simulink model "kinovaMicoSimscapeModel"  (R2021b)
(part 21 of 50)

Y2_4_1=(5991417*ddqr2)/50000000 - (1786417*ddqr3)/50000000 - (203*ddqr1*cos(q2))/100000 - (3393*ddqr2*cos(q3))/31250 + (3393*ddqr3*cos(q3))/62500 - (4329*ddqr4*cos(q4))/625000 - (1369*ddqr2*cos(2*q4))/2000000 + (1369*ddqr3*cos(2*q4))/2000000 + (3393*dq2*dqr3*sin(q3))/62500 + (3393*dq3*dqr2*sin(q3))/62500 - (3393*dq3*dqr3*sin(q3))/62500 + (4329*dq4*dqr4*sin(q4))/625000 - (841*dq1*dqr1*sin(2*q2))/20000 + (1369*dq2*dqr4*sin(2*q4))/2000000 + (1369*dq4*dqr2*sin(2*q4))/2000000 - (1369*dq3*dqr4*sin(2*q4))/2000000 - (1369*dq4*dqr3*sin(2*q4))/2000000 + (819*ddqr1*cos(q2)*cos(q3))/625000 + (1073*ddqr1*cos(q2)*cos(q4))/100000 + (1073*ddqr4*cos(q3)*cos(q4))/100000 + (819*ddqr1*sin(q2)*sin(q3))/625000 + (1073*ddqr2*sin(q3)*sin(q4))/50000 - (1073*ddqr3*sin(q3)*sin(q4))/100000 - (3393*dq1*dqr1*cos(2*q2)*sin(q3))/62500 + (3393*dq1*dqr1*sin(2*q2)*cos(q3))/62500 - (4329*ddqr1*cos(q2)*cos(q3)*cos(q4))/625000 - (259*ddqr1*cos(q2)*sin(q3)*sin(q4))/1000000 + (259*ddqr1*cos(q3)*sin(q2)*sin(q4))/1000000 - (4329*ddqr1*cos(q4)*sin(q2)*sin(q3))/625000 + (1717967*dq1*dqr1*cos(2*q2)*sin(2*q3))/100000000 - (1717967*dq1*dqr1*cos(2*q3)*sin(2*q2))/100000000 + (1369*ddqr1*sin(2*q4)*cos(q2)*sin(q3))/2000000 - (1369*ddqr1*sin(2*q4)*cos(q3)*sin(q2))/2000000 - (1369*dq1*dqr4*cos(q2)*sin(q3))/2000000 + (1369*dq1*dqr4*cos(q3)*sin(q2))/2000000 - (1369*dq4*dqr1*cos(q2)*sin(q3))/2000000 + (1369*dq4*dqr1*cos(q3)*sin(q2))/2000000 - (1073*dq1*dqr4*cos(q2)*sin(q4))/100000 - (1073*dq4*dqr1*cos(q2)*sin(q4))/100000 + (1073*dq2*dqr3*cos(q3)*sin(q4))/100000 + (1073*dq3*dqr2*cos(q3)*sin(q4))/100000 + (1073*dq2*dqr4*cos(q4)*sin(q3))/100000 - (1073*dq3*dqr3*cos(q3)*sin(q4))/100000 + (1073*dq4*dqr2*cos(q4)*sin(q3))/100000 - (1073*dq3*dqr4*cos(q4)*sin(q3))/100000 - (1073*dq4*dqr3*cos(q4)*sin(q3))/100000 - (1073*dq4*dqr4*cos(q3)*sin(q4))/100000 - (1073*dq1*dqr1*cos(2*q2)*cos(q3)*sin(q4))/100000 + (1369*dq1*dqr4*cos(2*q4)*cos(q2)*sin(q3))/2000000 - (1369*dq1*dqr4*cos(2*q4)*cos(q3)*sin(q2))/2000000 + (1369*dq4*dqr1*cos(2*q4)*cos(q2)*sin(q3))/2000000 - (1369*dq4*dqr1*cos(2*q4)*cos(q3)*sin(q2))/2000000 - (1073*dq1*dqr1*sin(2*q2)*sin(q3)*sin(q4))/100000 + (4329*dq1*dqr1*cos(2*q2)*cos(2*q3)*sin(q4))/625000 + (4329*dq1*dqr1*sin(2*q2)*sin(2*q3)*sin(q4))/625000 + (4329*dq1*dqr4*cos(q2)*cos(q3)*sin(q4))/625000 + (4329*dq4*dqr1*cos(q2)*cos(q3)*sin(q4))/625000 + (1369*dq1*dqr1*cos(2*q2)*cos(2*q4)*sin(2*q3))/4000000 - (1369*dq1*dqr1*cos(2*q3)*cos(2*q4)*sin(2*q2))/4000000 + (4329*dq1*dqr4*sin(q2)*sin(q3)*sin(q4))/625000 + (4329*dq4*dqr1*sin(q2)*sin(q3)*sin(q4))/625000;
Y2_5_1=(25433*dq3*dqr2*sin(q3))/400000 - (841*dq1*dqr1*sin(2*q2))/20000 - (25433*dq1*dqr1*cos(2*q2)*sin(q3))/400000 + (25433*dq1*dqr1*sin(2*q2)*cos(q3))/400000 - (1369*dq5*dqr1*cos(q2)*sin(q3))/4000000 + (1369*dq5*dqr1*cos(q3)*sin(q2))/4000000 + (4107*dq4*dqr1*cos(2*q5)*cos(q2)*sin(q3))/16000000 - (4107*dq4*dqr1*cos(2*q5)*cos(q3)*sin(q2))/16000000 - dq1*dqr1*cos(2*q2)*sin(2*q3)*((23717*3^(1/2))/40000000 - 36744657/1600000000) + dq1*dqr1*cos(2*q3)*sin(2*q2)*((23717*3^(1/2))/40000000 - 36744657/1600000000) - dq4*dqr1*cos(q2)*sin(q3)*((23717*3^(1/2))/20000000 + 2122493/800000000) + dq4*dqr1*cos(q3)*sin(q2)*((23717*3^(1/2))/20000000 + 2122493/800000000) + (1073*3^(1/2)*dq3*dqr2*cos(q5)*sin(q3))/200000 + (1073*dq4*dqr1*cos(q2)*cos(q4)*sin(q5))/100000 + (1073*dq4*dqr1*cos(q2)*cos(q5)*sin(q4))/200000 - (1073*dq3*dqr2*cos(q3)*cos(q4)*sin(q5))/100000 - (1073*dq3*dqr2*cos(q3)*cos(q5)*sin(q4))/200000 + (1073*dq5*dqr1*cos(q2)*cos(q4)*sin(q5))/200000 + (1073*dq5*dqr1*cos(q2)*cos(q5)*sin(q4))/100000 - (1073*dq4*dqr2*cos(q4)*cos(q5)*sin(q3))/200000 - (1073*dq5*dqr2*cos(q4)*cos(q5)*sin(q3))/100000 + (12321*dq1*dqr1*cos(2*q2)*cos(2*q5)*sin(2*q3))/32000000 - (12321*dq1*dqr1*cos(2*q3)*cos(2*q5)*sin(2*q2))/32000000 + (1073*dq4*dqr2*sin(q3)*sin(q4)*sin(q5))/100000 + (1073*dq5*dqr2*sin(q3)*sin(q4)*sin(q5))/200000 - dq4*dqr1*cos(q2)*sin(q4)*((18589*3^(1/2))/2000000 + 1073/100000) + dq3*dqr2*cos(q3)*sin(q4)*((18589*3^(1/2))/2000000 + 1073/100000) + dq4*dqr2*cos(q4)*sin(q3)*((18589*3^(1/2))/2000000 + 1073/100000) + (1369*dq1*dqr1*cos(2*q2)*cos(2*q4)*cos(2*q5)*sin(2*q3))/6400000 - (1369*dq1*dqr1*cos(2*q3)*cos(2*q4)*cos(2*q5)*sin(2*q2))/6400000 + (1073*dq1*dqr1*sin(2*q2)*cos(q4)*sin(q3)*sin(q5))/100000 + (1073*dq1*dqr1*sin(2*q2)*cos(q5)*sin(q3)*sin(q4))/200000 - (1369*3^(1/2)*dq5*dqr1*cos(q2)*cos(q3)*sin(q4))/4000000 - (1369*dq1*dqr1*cos(2*q2)*sin(2*q3)*sin(2*q4)*sin(2*q5))/8000000 + (1369*dq1*dqr1*cos(2*q3)*sin(2*q2)*sin(2*q4)*sin(2*q5))/8000000 - dq1*dqr1*cos(2*q2)*cos(q3)*sin(q4)*((18589*3^(1/2))/2000000 + 1073/100000) - (1369*3^(1/2)*dq5*dqr1*sin(q2)*sin(q3)*sin(q4))/4000000 - (32449*dq1*dqr1*cos(2*q2)*cos(2*q3)*cos(q4)*sin(q5))/4000000 + (1369*dq4*dqr1*cos(2*q4)*cos(2*q5)*cos(q2)*sin(q3))/3200000 - (1369*dq4*dqr1*cos(2*q4)*cos(2*q5)*cos(q3)*sin(q2))/3200000 + (1369*dq5*dqr1*cos(2*q4)*cos(2*q5)*cos(q2)*sin(q3))/4000000 - (1369*dq5*dqr1*cos(2*q4)*cos(2*q5)*cos(q3)*sin(q2))/4000000 - dq1*dqr1*sin(2*q2)*sin(q3)*sin(q4)*((18589*3^(1/2))/2000000 + 1073/100000) + dq1*dqr1*cos(2*q2)*cos(2*q4)*sin(2*q3)*((23717*3^(1/2))/40000000 + 1574893/1600000000) - dq1*dqr1*cos(2*q3)*cos(2*q4)*sin(2*q2)*((23717*3^(1/2))/40000000 + 1574893/1600000000) + dq4*dqr1*cos(2*q4)*cos(q2)*sin(q3)*((23717*3^(1/2))/20000000 + 1574893/800000000) - dq4*dqr1*cos(2*q4)*cos(q3)*sin(q2)*((23717*3^(1/2))/20000000 + 1574893/800000000) - (32449*dq1*dqr1*sin(2*q2)*sin(2*q3)*cos(q4)*sin(q5))/4000000 - (1369*dq4*dqr1*sin(2*q4)*sin(2*q5)*cos(q2)*sin(q3))/4000000 + (1369*dq4*dqr1*sin(2*q4)*sin(2*q5)*cos(q3)*sin(q2))/4000000 - (1369*dq5*dqr1*sin(2*q4)*sin(2*q5)*cos(q2)*sin(q3))/3200000 + (1369*dq5*dqr1*sin(2*q4)*sin(2*q5)*cos(q3)*sin(q2))/3200000 - (1073*3^(1/2)*dq1*dqr1*cos(2*q2)*cos(q5)*sin(q3))/200000 + (1073*3^(1/2)*dq1*dqr1*sin(2*q2)*cos(q3)*cos(q5))/200000 - (32449*dq4*dqr1*cos(q2)*cos(q3)*cos(q4)*sin(q5))/4000000 - (32449*dq5*dqr1*cos(q2)*cos(q3)*cos(q4)*sin(q5))/8000000 - (32449*dq5*dqr1*cos(q2)*cos(q3)*cos(q5)*sin(q4))/4000000 + dq1*dqr1*cos(2*q2)*sin(2*q3)*cos(q5)*((348207*3^(1/2))/80000000 + 1369/4000000) - dq1*dqr1*cos(2*q3)*sin(2*q2)*cos(q5)*((348207*3^(1/2))/80000000 + 1369/4000000) + dq1*dqr1*cos(2*q2)*cos(2*q3)*sin(q4)*((548467*3^(1/2))/80000000 + 32449/4000000) - (32449*dq4*dqr1*cos(q4)*sin(q2)*sin(q3)*sin(q5))/4000000 - (32449*dq5*dqr1*cos(q4)*sin(q2)*sin(q3)*sin(q5))/8000000 - (32449*dq5*dqr1*cos(q5)*sin(q2)*sin(q3)*sin(q4))/4000000 + dq1*dqr1*sin(2*q2)*sin(2*q3)*sin(q4)*((548467*3^(1/2))/80000000 + 32449/4000000) + dq4*dqr1*cos(q2)*cos(q5)*sin(q3)*((23717*3^(1/2))/40000000 + 1369/2000000) - dq4*dqr1*cos(q3)*cos(q5)*sin(q2)*((23717*3^(1/2))/40000000 + 1369/2000000) + dq5*dqr1*cos(q2)*cos(q5)*sin(q3)*((23717*3^(1/2))/40000000 + 1369/2000000) - dq5*dqr1*cos(q3)*cos(q5)*sin(q2)*((23717*3^(1/2))/40000000 + 1369/2000000) + dq4*dqr1*cos(q2)*cos(q3)*sin(q4)*((548467*3^(1/2))/80000000 + 32449/4000000) + (1073*dq1*dqr1*cos(2*q2)*cos(q3)*cos(q4)*sin(q5))/100000 + (1073*dq1*dqr1*cos(2*q2)*cos(q3)*cos(q5)*sin(q4))/200000 + dq4*dqr1*sin(q2)*sin(q3)*sin(q4)*((548467*3^(1/2))/80000000 + 32449/4000000) - (1369*3^(1/2)*dq1*dqr1*cos(2*q2)*cos(2*q3)*cos(2*q5)*sin(q4))/8000000 - (1369*3^(1/2)*dq1*dqr1*cos(2*q2)*cos(2*q3)*sin(2*q5)*cos(q4))/4000000 - dq4*dqr1*cos(2*q4)*cos(q2)*cos(q5)*sin(q3)*((23717*3^(1/2))/40000000 + 1369/2000000) + dq4*dqr1*cos(2*q4)*cos(q3)*cos(q5)*sin(q2)*((23717*3^(1/2))/40000000 + 1369/2000000) - dq5*dqr1*cos(2*q4)*cos(q2)*cos(q5)*sin(q3)*((23717*3^(1/2))/40000000 + 1369/2000000) + dq5*dqr1*cos(2*q4)*cos(q3)*cos(q5)*sin(q2)*((23717*3^(1/2))/40000000 + 1369/2000000) - (1369*3^(1/2)*dq1*dqr1*cos(2*q5)*sin(2*q2)*sin(2*q3)*sin(q4))/8000000 - (1369*3^(1/2)*dq1*dqr1*sin(2*q2)*sin(2*q3)*sin(2*q5)*cos(q4))/4000000 + dq4*dqr1*sin(2*q4)*cos(q2)*sin(q3)*sin(q5)*((23717*3^(1/2))/20000000 + 1369/1000000) - dq4*dqr1*sin(2*q4)*cos(q3)*sin(q2)*sin(q5)*((23717*3^(1/2))/20000000 + 1369/1000000) + dq5*dqr1*sin(2*q4)*cos(q2)*sin(q3)*sin(q5)*((23717*3^(1/2))/80000000 + 1369/4000000) - dq5*dqr1*sin(2*q4)*cos(q3)*sin(q2)*sin(q5)*((23717*3^(1/2))/80000000 + 1369/4000000) - (1369*3^(1/2)*dq4*dqr1*cos(2*q5)*cos(q2)*cos(q3)*sin(q4))/8000000 - (1369*3^(1/2)*dq4*dqr1*sin(2*q5)*cos(q2)*cos(q3)*cos(q4))/4000000 - (1369*3^(1/2)*dq5*dqr1*cos(2*q5)*cos(q2)*cos(q3)*sin(q4))/4000000 - (1369*3^(1/2)*dq5*dqr1*sin(2*q5)*cos(q2)*cos(q3)*cos(q4))/8000000 + dq1*dqr1*cos(2*q2)*cos(2*q3)*cos(q5)*sin(q4)*((1369*3^(1/2))/2000000 - 45547/20000000) - (1369*3^(1/2)*dq4*dqr1*cos(2*q5)*sin(q2)*sin(q3)*sin(q4))/8000000 - (1369*3^(1/2)*dq4*dqr1*sin(2*q5)*cos(q4)*sin(q2)*sin(q3))/4000000 - (1369*3^(1/2)*dq5*dqr1*cos(2*q5)*sin(q2)*sin(q3)*sin(q4))/4000000 - (1369*3^(1/2)*dq5*dqr1*sin(2*q5)*cos(q4)*sin(q2)*sin(q3))/8000000 + dq1*dqr1*sin(2*q2)*sin(2*q3)*cos(q5)*sin(q4)*((1369*3^(1/2))/2000000 - 45547/20000000) + dq4*dqr1*cos(q2)*cos(q3)*cos(q5)*sin(q4)*((1369*3^(1/2))/2000000 - 45547/20000000) + dq4*dqr1*cos(q5)*sin(q2)*sin(q3)*sin(q4)*((1369*3^(1/2))/2000000 - 45547/20000000) - dq1*dqr1*cos(2*q2)*cos(2*q4)*sin(2*q3)*cos(q5)*((23717*3^(1/2))/80000000 + 1369/4000000) + dq1*dqr1*cos(2*q3)*cos(2*q4)*sin(2*q2)*cos(q5)*((23717*3^(1/2))/80000000 + 1369/4000000) + dq1*dqr1*cos(2*q2)*sin(2*q3)*sin(2*q4)*sin(q5)*((23717*3^(1/2))/40000000 + 1369/2000000) - dq1*dqr1*cos(2*q3)*sin(2*q2)*sin(2*q4)*sin(q5)*((23717*3^(1/2))/40000000 + 1369/2000000);
Y2_5_2=(25433*dq2*dqr3*sin(q3))/400000 - (25433*dq3*dqr3*sin(q3))/400000 - (4107*dq5*dqr2*sin(2*q5))/16000000 + (4107*dq5*dqr3*sin(2*q5))/16000000 - dq5*dqr2*sin(q5)*((300773*3^(1/2))/80000000 - 1369/4000000) + dq5*dqr3*sin(q5)*((300773*3^(1/2))/80000000 - 1369/4000000) + dq4*dqr4*sin(q4)*((548467*3^(1/2))/80000000 + 32449/4000000) - (1369*3^(1/2)*dq5*dqr4*sin(q4))/4000000 + (1369*dq2*dqr4*cos(2*q4)*sin(2*q5))/4000000 + (1369*dq2*dqr4*cos(2*q5)*sin(2*q4))/3200000 + (1369*dq4*dqr2*cos(2*q4)*sin(2*q5))/4000000 + (1369*dq4*dqr2*cos(2*q5)*sin(2*q4))/3200000 - (1369*dq3*dqr4*cos(2*q4)*sin(2*q5))/4000000 - (1369*dq3*dqr4*cos(2*q5)*sin(2*q4))/3200000 - (1369*dq4*dqr3*cos(2*q4)*sin(2*q5))/4000000 - (1369*dq4*dqr3*cos(2*q5)*sin(2*q4))/3200000 + (1369*dq5*dqr2*cos(2*q4)*sin(2*q5))/3200000 + (1369*dq5*dqr2*cos(2*q5)*sin(2*q4))/4000000 - (1369*dq5*dqr3*cos(2*q4)*sin(2*q5))/3200000 - (1369*dq5*dqr3*cos(2*q5)*sin(2*q4))/4000000 + dq2*dqr4*sin(2*q4)*((23717*3^(1/2))/20000000 + 1574893/800000000) + dq4*dqr2*sin(2*q4)*((23717*3^(1/2))/20000000 + 1574893/800000000) - dq3*dqr4*sin(2*q4)*((23717*3^(1/2))/20000000 + 1574893/800000000) - dq4*dqr3*sin(2*q4)*((23717*3^(1/2))/20000000 + 1574893/800000000) - (32449*dq4*dqr4*cos(q4)*sin(q5))/4000000 - (32449*dq5*dqr4*cos(q4)*sin(q5))/8000000 - (32449*dq5*dqr4*cos(q5)*sin(q4))/4000000 + dq4*dqr4*cos(q5)*sin(q4)*((1369*3^(1/2))/2000000 - 45547/20000000) + (4107*dq1*dqr4*cos(2*q5)*cos(q2)*sin(q3))/16000000 - (4107*dq1*dqr4*cos(2*q5)*cos(q3)*sin(q2))/16000000 - dq1*dqr4*cos(q2)*sin(q3)*((23717*3^(1/2))/20000000 + 2122493/800000000) + dq1*dqr4*cos(q3)*sin(q2)*((23717*3^(1/2))/20000000 + 2122493/800000000) + (1073*3^(1/2)*dq2*dqr3*cos(q5)*sin(q3))/200000 - (1073*3^(1/2)*dq3*dqr3*cos(q5)*sin(q3))/200000 + (1073*3^(1/2)*dq5*dqr2*cos(q3)*sin(q5))/200000 - (1073*3^(1/2)*dq5*dqr3*cos(q3)*sin(q5))/200000 - dq2*dqr4*cos(2*q4)*sin(q5)*((23717*3^(1/2))/20000000 + 1369/1000000) - dq4*dqr2*cos(2*q4)*sin(q5)*((23717*3^(1/2))/20000000 + 1369/1000000) + dq3*dqr4*cos(2*q4)*sin(q5)*((23717*3^(1/2))/20000000 + 1369/1000000) + dq4*dqr3*cos(2*q4)*sin(q5)*((23717*3^(1/2))/20000000 + 1369/1000000) - dq2*dqr4*sin(2*q4)*cos(q5)*((23717*3^(1/2))/40000000 + 1369/2000000) - dq4*dqr2*sin(2*q4)*cos(q5)*((23717*3^(1/2))/40000000 + 1369/2000000) + dq3*dqr4*sin(2*q4)*cos(q5)*((23717*3^(1/2))/40000000 + 1369/2000000) + dq4*dqr3*sin(2*q4)*cos(q5)*((23717*3^(1/2))/40000000 + 1369/2000000) - dq5*dqr2*sin(2*q4)*cos(q5)*((23717*3^(1/2))/40000000 + 1369/2000000) + dq5*dqr3*sin(2*q4)*cos(q5)*((23717*3^(1/2))/40000000 + 1369/2000000) - dq5*dqr2*cos(2*q4)*sin(q5)*((23717*3^(1/2))/80000000 + 1369/4000000) + dq5*dqr3*cos(2*q4)*sin(q5)*((23717*3^(1/2))/80000000 + 1369/4000000) - (1369*3^(1/2)*dq4*dqr4*cos(2*q5)*sin(q4))/8000000 - (1369*3^(1/2)*dq4*dqr4*sin(2*q5)*cos(q4))/4000000 - (1369*3^(1/2)*dq5*dqr4*cos(2*q5)*sin(q4))/4000000 - (1369*3^(1/2)*dq5*dqr4*sin(2*q5)*cos(q4))/8000000 + (1073*dq1*dqr4*cos(q2)*cos(q4)*sin(q5))/100000 + (1073*dq1*dqr4*cos(q2)*cos(q5)*sin(q4))/200000 - (1073*dq2*dqr3*cos(q3)*cos(q4)*sin(q5))/100000 - (1073*dq2*dqr3*cos(q3)*cos(q5)*sin(q4))/200000 - (1073*dq2*dqr4*cos(q4)*cos(q5)*sin(q3))/200000 + (1073*dq3*dqr3*cos(q3)*cos(q4)*sin(q5))/100000 + (1073*dq3*dqr3*cos(q3)*cos(q5)*sin(q4))/200000 + (1073*dq3*dqr4*cos(q4)*cos(q5)*sin(q3))/200000 + (1073*dq4*dqr3*cos(q4)*cos(q5)*sin(q3))/200000 + (1073*dq4*dqr4*cos(q3)*cos(q4)*sin(q5))/100000 + (1073*dq4*dqr4*cos(q3)*cos(q5)*sin(q4))/200000 + (1073*dq5*dqr3*cos(q4)*cos(q5)*sin(q3))/100000 + (1073*dq5*dqr4*cos(q3)*cos(q4)*sin(q5))/200000 + (1073*dq5*dqr4*cos(q3)*cos(q5)*sin(q4))/100000 + (1073*dq2*dqr4*sin(q3)*sin(q4)*sin(q5))/100000 - (1073*dq3*dqr4*sin(q3)*sin(q4)*sin(q5))/100000 - (1073*dq4*dqr3*sin(q3)*sin(q4)*sin(q5))/100000 - (1073*dq5*dqr3*sin(q3)*sin(q4)*sin(q5))/200000 - dq1*dqr4*cos(q2)*sin(q4)*((18589*3^(1/2))/2000000 + 1073/100000) + dq2*dqr3*cos(q3)*sin(q4)*((18589*3^(1/2))/2000000 + 1073/100000) + dq2*dqr4*cos(q4)*sin(q3)*((18589*3^(1/2))/2000000 + 1073/100000) - dq3*dqr3*cos(q3)*sin(q4)*((18589*3^(1/2))/2000000 + 1073/100000) - dq3*dqr4*cos(q4)*sin(q3)*((18589*3^(1/2))/2000000 + 1073/100000) - dq4*dqr3*cos(q4)*sin(q3)*((18589*3^(1/2))/2000000 + 1073/100000) - dq4*dqr4*cos(q3)*sin(q4)*((18589*3^(1/2))/2000000 + 1073/100000) + (1369*dq1*dqr4*cos(2*q4)*cos(2*q5)*cos(q2)*sin(q3))/3200000 - (1369*dq1*dqr4*cos(2*q4)*cos(2*q5)*cos(q3)*sin(q2))/3200000 + dq1*dqr4*cos(2*q4)*cos(q2)*sin(q3)*((23717*3^(1/2))/20000000 + 1574893/800000000) - dq1*dqr4*cos(2*q4)*cos(q3)*sin(q2)*((23717*3^(1/2))/20000000 + 1574893/800000000) - (1369*dq1*dqr4*sin(2*q4)*sin(2*q5)*cos(q2)*sin(q3))/4000000 + (1369*dq1*dqr4*sin(2*q4)*sin(2*q5)*cos(q3)*sin(q2))/4000000 - (32449*dq1*dqr4*cos(q2)*cos(q3)*cos(q4)*sin(q5))/4000000 - (32449*dq1*dqr4*cos(q4)*sin(q2)*sin(q3)*sin(q5))/4000000 - (32449*dq1*dqr5*cos(q5)*sin(q2)*sin(q3)*sin(q4))/4000000 + dq1*dqr4*cos(q2)*cos(q5)*sin(q3)*((23717*3^(1/2))/40000000 + 1369/2000000) - dq1*dqr4*cos(q3)*cos(q5)*sin(q2)*((23717*3^(1/2))/40000000 + 1369/2000000) + dq1*dqr4*cos(q2)*cos(q3)*sin(q4)*((548467*3^(1/2))/80000000 + 32449/4000000) + dq1*dqr4*sin(q2)*sin(q3)*sin(q4)*((548467*3^(1/2))/80000000 + 32449/4000000) - dq1*dqr4*cos(2*q4)*cos(q2)*cos(q5)*sin(q3)*((23717*3^(1/2))/40000000 + 1369/2000000) + dq1*dqr4*cos(2*q4)*cos(q3)*cos(q5)*sin(q2)*((23717*3^(1/2))/40000000 + 1369/2000000) + dq1*dqr4*sin(2*q4)*cos(q2)*sin(q3)*sin(q5)*((23717*3^(1/2))/20000000 + 1369/1000000) - dq1*dqr4*sin(2*q4)*cos(q3)*sin(q2)*sin(q5)*((23717*3^(1/2))/20000000 + 1369/1000000) - (1369*3^(1/2)*dq1*dqr4*cos(2*q5)*cos(q2)*cos(q3)*sin(q4))/8000000 - (1369*3^(1/2)*dq1*dqr4*sin(2*q5)*cos(q2)*cos(q3)*cos(q4))/4000000 - (1369*3^(1/2)*dq1*dqr4*cos(2*q5)*sin(q2)*sin(q3)*sin(q4))/8000000 - (1369*3^(1/2)*dq1*dqr4*sin(2*q5)*cos(q4)*sin(q2)*sin(q3))/4000000 + dq1*dqr4*cos(q2)*cos(q3)*cos(q5)*sin(q4)*((1369*3^(1/2))/2000000 - 45547/20000000) + dq1*dqr4*cos(q5)*sin(q2)*sin(q3)*sin(q4)*((1369*3^(1/2))/2000000 - 45547/20000000);
Y2_5_3=(4107*dq3*dqr5*sin(2*q5))/16000000 - (4107*dq2*dqr5*sin(2*q5))/16000000 + (6139*ddqr1*cos(q2)*cos(q3))/4000000 + (6139*ddqr1*sin(q2)*sin(q3))/4000000 - (32449*ddqr4*sin(q4)*sin(q5))/4000000 - ddqr2*sin(2*q4)*sin(q5)*((23717*3^(1/2))/20000000 + 1369/1000000) + ddqr3*sin(2*q4)*sin(q5)*((23717*3^(1/2))/20000000 + 1369/1000000) - dq2*dqr5*sin(q5)*((300773*3^(1/2))/80000000 - 1369/4000000) + dq3*dqr5*sin(q5)*((300773*3^(1/2))/80000000 - 1369/4000000) - (1073*ddqr1*cos(q2)*cos(q4)*cos(q5))/200000 - (1369*3^(1/2)*ddqr4*sin(2*q5)*sin(q4))/4000000 + (1073*ddqr1*cos(q2)*sin(q4)*sin(q5))/100000 - (1073*ddqr2*cos(q4)*sin(q3)*sin(q5))/50000 - (1073*ddqr2*cos(q5)*sin(q3)*sin(q4))/100000 + (1073*ddqr3*cos(q4)*sin(q3)*sin(q5))/100000 + (1073*ddqr3*cos(q5)*sin(q3)*sin(q4))/200000 + (1073*ddqr4*cos(q3)*sin(q4)*sin(q5))/100000 + (1073*ddqr5*cos(q3)*sin(q4)*sin(q5))/200000 - (1369*3^(1/2)*dq4*dqr5*sin(q4))/4000000 + ddqr1*cos(q2)*cos(q4)*((18589*3^(1/2))/2000000 + 1073/100000) + (1369*dq2*dqr5*cos(2*q4)*sin(2*q5))/3200000 + (1369*dq2*dqr5*cos(2*q5)*sin(2*q4))/4000000 - (1369*dq3*dqr5*cos(2*q4)*sin(2*q5))/3200000 - (1369*dq3*dqr5*cos(2*q5)*sin(2*q4))/4000000 + ddqr2*sin(q3)*sin(q4)*((18589*3^(1/2))/1000000 + 1073/50000) - ddqr3*sin(q3)*sin(q4)*((18589*3^(1/2))/2000000 + 1073/100000) - ddqr5*sin(q4)*sin(q5)*((1369*3^(1/2))/2000000 + 58349/10000000) - (1369*dq1*dqr5*cos(q2)*sin(q3))/4000000 + (1369*dq1*dqr5*cos(q3)*sin(q2))/4000000 - (32449*dq4*dqr5*cos(q4)*sin(q5))/8000000 - (32449*dq4*dqr5*cos(q5)*sin(q4))/4000000 - (32449*dq5*dqr5*cos(q4)*sin(q5))/4000000 - (1073*3^(1/2)*ddqr5*sin(q3)*sin(q5))/200000 - dq5*dqr5*cos(q5)*sin(q4)*((1369*3^(1/2))/2000000 + 58349/10000000) + ddqr1*sin(2*q4)*cos(q2)*sin(q3)*((23717*3^(1/2))/20000000 + 1574893/800000000) - ddqr1*sin(2*q4)*cos(q3)*sin(q2)*((23717*3^(1/2))/20000000 + 1574893/800000000) - (32449*ddqr1*cos(q2)*cos(q3)*sin(q4)*sin(q5))/4000000 + (259*ddqr1*cos(q2)*cos(q4)*sin(q3)*sin(q5))/1000000 + (259*ddqr1*cos(q2)*cos(q5)*sin(q3)*sin(q4))/2000000 - (259*ddqr1*cos(q3)*cos(q4)*sin(q2)*sin(q5))/1000000 - (259*ddqr1*cos(q3)*cos(q5)*sin(q2)*sin(q4))/2000000 + (1073*3^(1/2)*dq2*dqr5*cos(q3)*sin(q5))/200000 - (1073*3^(1/2)*dq3*dqr5*cos(q3)*sin(q5))/200000 - (1073*3^(1/2)*dq5*dqr5*cos(q5)*sin(q3))/200000 - (32449*ddqr1*sin(q2)*sin(q3)*sin(q4)*sin(q5))/4000000 - dq2*dqr5*sin(2*q4)*cos(q5)*((23717*3^(1/2))/40000000 + 1369/2000000) + dq3*dqr5*sin(2*q4)*cos(q5)*((23717*3^(1/2))/40000000 + 1369/2000000) - dq2*dqr5*cos(2*q4)*sin(q5)*((23717*3^(1/2))/80000000 + 1369/4000000) + dq3*dqr5*cos(2*q4)*sin(q5)*((23717*3^(1/2))/80000000 + 1369/4000000) - ddqr1*cos(q2)*cos(q3)*cos(q4)*((548467*3^(1/2))/80000000 + 32449/4000000) - ddqr1*cos(q2)*sin(q3)*sin(q4)*((4487*3^(1/2))/20000000 + 259/1000000) + ddqr1*cos(q3)*sin(q2)*sin(q4)*((4487*3^(1/2))/20000000 + 259/1000000) - ddqr1*cos(q4)*sin(q2)*sin(q3)*((548467*3^(1/2))/80000000 + 32449/4000000) - (1369*3^(1/2)*dq4*dqr5*cos(2*q5)*sin(q4))/4000000 - (1369*3^(1/2)*dq4*dqr5*sin(2*q5)*cos(q4))/8000000 + (259*3^(1/2)*ddqr1*cos(q2)*cos(q3)*cos(q5))/2000000 + (1073*dq1*dqr5*cos(q2)*cos(q4)*sin(q5))/200000 + (1073*dq1*dqr5*cos(q2)*cos(q5)*sin(q4))/100000 - (1073*dq2*dqr5*cos(q4)*cos(q5)*sin(q3))/100000 + (1073*dq3*dqr5*cos(q4)*cos(q5)*sin(q3))/100000 + (1073*dq4*dqr5*cos(q3)*cos(q4)*sin(q5))/200000 + (1073*dq4*dqr5*cos(q3)*cos(q5)*sin(q4))/100000 + (1073*dq5*dqr5*cos(q3)*cos(q4)*sin(q5))/100000 + (1073*dq5*dqr5*cos(q3)*cos(q5)*sin(q4))/200000 + (259*3^(1/2)*ddqr1*cos(q5)*sin(q2)*sin(q3))/2000000 + (1073*dq2*dqr5*sin(q3)*sin(q4)*sin(q5))/200000 - (1073*dq3*dqr5*sin(q3)*sin(q4)*sin(q5))/200000 + (1369*ddqr1*cos(2*q4)*sin(2*q5)*cos(q2)*sin(q3))/4000000 - (1369*ddqr1*cos(2*q4)*sin(2*q5)*cos(q3)*sin(q2))/4000000 + (1369*ddqr1*cos(2*q5)*sin(2*q4)*cos(q2)*sin(q3))/3200000 - (1369*ddqr1*cos(2*q5)*sin(2*q4)*cos(q3)*sin(q2))/3200000 - (1369*3^(1/2)*ddqr1*sin(2*q5)*sin(q2)*sin(q3)*sin(q4))/4000000 - (1369*3^(1/2)*dq1*dqr5*cos(q2)*cos(q3)*sin(q4))/4000000 - (1369*3^(1/2)*dq1*dqr5*sin(q2)*sin(q3)*sin(q4))/4000000 - ddqr1*cos(q2)*cos(q3)*cos(q4)*cos(q5)*((1369*3^(1/2))/2000000 - 45547/20000000) + (1369*dq1*dqr5*cos(2*q4)*cos(2*q5)*cos(q2)*sin(q3))/4000000 - (1369*dq1*dqr5*cos(2*q4)*cos(2*q5)*cos(q3)*sin(q2))/4000000 - ddqr1*cos(q4)*cos(q5)*sin(q2)*sin(q3)*((1369*3^(1/2))/2000000 - 45547/20000000) - (1369*dq1*dqr5*sin(2*q4)*sin(2*q5)*cos(q2)*sin(q3))/3200000 + (1369*dq1*dqr5*sin(2*q4)*sin(2*q5)*cos(q3)*sin(q2))/3200000 - (32449*dq1*dqr5*cos(q2)*cos(q3)*cos(q4)*sin(q5))/8000000 - (32449*dq1*dqr5*cos(q2)*cos(q3)*cos(q5)*sin(q4))/4000000 - (32449*dq1*dqr5*cos(q4)*sin(q2)*sin(q3)*sin(q5))/8000000 - ddqr1*cos(2*q4)*cos(q2)*sin(q3)*sin(q5)*((23717*3^(1/2))/20000000 + 1369/1000000) + ddqr1*cos(2*q4)*cos(q3)*sin(q2)*sin(q5)*((23717*3^(1/2))/20000000 + 1369/1000000) - ddqr1*sin(2*q4)*cos(q2)*cos(q5)*sin(q3)*((23717*3^(1/2))/40000000 + 1369/2000000) + ddqr1*sin(2*q4)*cos(q3)*cos(q5)*sin(q2)*((23717*3^(1/2))/40000000 + 1369/2000000) + (1369*3^(1/2)*ddqr1*cos(2*q5)*cos(q2)*cos(q3)*cos(q4))/8000000 + dq1*dqr5*cos(q2)*cos(q5)*sin(q3)*((23717*3^(1/2))/40000000 + 1369/2000000) - dq1*dqr5*cos(q3)*cos(q5)*sin(q2)*((23717*3^(1/2))/40000000 + 1369/2000000) + (1369*3^(1/2)*ddqr1*cos(2*q5)*cos(q4)*sin(q2)*sin(q3))/8000000 - (1369*3^(1/2)*ddqr1*sin(2*q5)*cos(q2)*cos(q3)*sin(q4))/4000000 - dq1*dqr5*cos(2*q4)*cos(q2)*cos(q5)*sin(q3)*((23717*3^(1/2))/40000000 + 1369/2000000) + dq1*dqr5*cos(2*q4)*cos(q3)*cos(q5)*sin(q2)*((23717*3^(1/2))/40000000 + 1369/2000000) + dq1*dqr5*sin(2*q4)*cos(q2)*sin(q3)*sin(q5)*((23717*3^(1/2))/80000000 + 1369/4000000) - dq1*dqr5*sin(2*q4)*cos(q3)*sin(q2)*sin(q5)*((23717*3^(1/2))/80000000 + 1369/4000000) - (1369*3^(1/2)*dq1*dqr5*cos(2*q5)*cos(q2)*cos(q3)*sin(q4))/4000000 - (1369*3^(1/2)*dq1*dqr5*sin(2*q5)*cos(q2)*cos(q3)*cos(q4))/8000000 - (1369*3^(1/2)*dq1*dqr5*cos(2*q5)*sin(q2)*sin(q3)*sin(q4))/4000000 - (1369*3^(1/2)*dq1*dqr5*sin(2*q5)*cos(q4)*sin(q2)*sin(q3))/8000000;
Y2_5_4=ddqr2*((23717*3^(1/2))/20000000 + 108269643/800000000) - ddqr3*((23717*3^(1/2))/20000000 + 40989643/800000000) - (203*ddqr1*cos(q2))/100000 - (25433*ddqr2*cos(q3))/200000 + (25433*ddqr3*cos(q3))/400000 + (4107*ddqr2*cos(2*q5))/16000000 - (4107*ddqr3*cos(2*q5))/16000000 - (1369*ddqr2*cos(2*q4)*cos(2*q5))/3200000 + (1369*ddqr3*cos(2*q4)*cos(2*q5))/3200000 - ddqr2*cos(2*q4)*((23717*3^(1/2))/20000000 + 1574893/800000000) + ddqr3*cos(2*q4)*((23717*3^(1/2))/20000000 + 1574893/800000000) + (1369*ddqr2*sin(2*q4)*sin(2*q5))/4000000 - (1369*ddqr3*sin(2*q4)*sin(2*q5))/4000000 + (32449*ddqr5*cos(q4)*cos(q5))/4000000 + ddqr2*cos(q5)*((300773*3^(1/2))/40000000 - 1369/2000000) - ddqr3*cos(q5)*((300773*3^(1/2))/40000000 - 1369/2000000) - ddqr4*cos(q4)*((548467*3^(1/2))/80000000 + 32449/4000000) + (1369*3^(1/2)*ddqr5*cos(q4))/2000000 + (1369*3^(1/2)*ddqr4*cos(2*q5)*cos(q4))/8000000 - (1073*ddqr4*cos(q3)*cos(q4)*cos(q5))/200000 - (1073*ddqr5*cos(q3)*cos(q4)*cos(q5))/100000 + ddqr4*cos(q3)*cos(q4)*((18589*3^(1/2))/2000000 + 1073/100000) - ddqr4*cos(q4)*cos(q5)*((1369*3^(1/2))/2000000 - 45547/20000000) - (1073*3^(1/2)*ddqr2*cos(q3)*cos(q5))/100000 + (1073*3^(1/2)*ddqr3*cos(q3)*cos(q5))/200000 + ddqr2*cos(2*q4)*cos(q5)*((23717*3^(1/2))/40000000 + 1369/2000000) - ddqr3*cos(2*q4)*cos(q5)*((23717*3^(1/2))/40000000 + 1369/2000000);
Y2_6_1=-(ddqr1*cos(q2))/625;
Y2_7_1=(29*ddqr3*cos(q3))/100 - (29*ddqr2*cos(q3))/50 + (29*dq2*dqr3*sin(q3))/100 + (29*dq3*dqr2*sin(q3))/100 - (29*dq3*dqr3*sin(q3))/100 - (ddqr1*cos(q2)*cos(q3))/625 - (ddqr1*sin(q2)*sin(q3))/625 - (29*dq1*dqr1*cos(2*q2)*sin(q3))/100 + (29*dq1*dqr1*sin(2*q2)*cos(q3))/100;
Y2_8_1=(1231*ddqr3)/5000 - (1231*ddqr2)/5000 + (29*ddqr2*cos(q3))/50 - (29*ddqr3*cos(q3))/100 - (29*dq2*dqr3*sin(q3))/100 - (29*dq3*dqr2*sin(q3))/100 + (29*dq3*dqr3*sin(q3))/100 - (7*ddqr1*cos(q2)*cos(q3))/1000 - (7*ddqr1*sin(q2)*sin(q3))/1000 + (29*dq1*dqr1*cos(2*q2)*sin(q3))/100 - (29*dq1*dqr1*sin(2*q2)*cos(q3))/100 - (1231*dq1*dqr1*cos(2*q2)*sin(2*q3))/10000 + (1231*dq1*dqr1*cos(2*q3)*sin(2*q2))/10000;
Y2_9_1=(29*ddqr2*cos(q3))/100 - (29*ddqr3*cos(q3))/200 - ddqr2*((37*3^(1/2))/2000 + 117/625) + ddqr3*((37*3^(1/2))/2000 + 117/625) - (29*dq2*dqr3*sin(q3))/200 - (29*dq3*dqr2*sin(q3))/200 + (29*dq3*dqr3*sin(q3))/200 + (37*3^(1/2)*ddqr2*cos(2*q4))/2000 - (37*3^(1/2)*ddqr3*cos(2*q4))/2000 - (7*ddqr1*cos(q2)*cos(q3))/2000 - (7*ddqr1*sin(q2)*sin(q3))/2000 + ddqr4*cos(q4)*((117*3^(1/2))/1250 + 37/2000) - dq4*dqr4*sin(q4)*((117*3^(1/2))/1250 + 37/2000) + (29*dq1*dqr1*cos(2*q2)*sin(q3))/200 - (29*dq1*dqr1*sin(2*q2)*cos(q3))/200 - (37*3^(1/2)*dq2*dqr4*sin(2*q4))/2000 - (37*3^(1/2)*dq4*dqr2*sin(2*q4))/2000 + (37*3^(1/2)*dq3*dqr4*sin(2*q4))/2000 + (37*3^(1/2)*dq4*dqr3*sin(2*q4))/2000 - (29*3^(1/2)*ddqr1*cos(q2)*cos(q4))/200 - (29*3^(1/2)*ddqr4*cos(q3)*cos(q4))/200 - (29*3^(1/2)*ddqr2*sin(q3)*sin(q4))/100 + (29*3^(1/2)*ddqr3*sin(q3)*sin(q4))/200 - (37*3^(1/2)*ddqr1*sin(2*q4)*cos(q2)*sin(q3))/2000 + (37*3^(1/2)*ddqr1*sin(2*q4)*cos(q3)*sin(q2))/2000 + (37*3^(1/2)*dq1*dqr4*cos(q2)*sin(q3))/2000 - (37*3^(1/2)*dq1*dqr4*cos(q3)*sin(q2))/2000 + (37*3^(1/2)*dq4*dqr1*cos(q2)*sin(q3))/2000 - (37*3^(1/2)*dq4*dqr1*cos(q3)*sin(q2))/2000 + (29*3^(1/2)*dq1*dqr4*cos(q2)*sin(q4))/200 + (29*3^(1/2)*dq4*dqr1*cos(q2)*sin(q4))/200 - (29*3^(1/2)*dq2*dqr3*cos(q3)*sin(q4))/200 - (29*3^(1/2)*dq3*dqr2*cos(q3)*sin(q4))/200 - (29*3^(1/2)*dq2*dqr4*cos(q4)*sin(q3))/200 + (29*3^(1/2)*dq3*dqr3*cos(q3)*sin(q4))/200 - (29*3^(1/2)*dq4*dqr2*cos(q4)*sin(q3))/200 + (29*3^(1/2)*dq3*dqr4*cos(q4)*sin(q3))/200 + (29*3^(1/2)*dq4*dqr3*cos(q4)*sin(q3))/200 + (29*3^(1/2)*dq4*dqr4*cos(q3)*sin(q4))/200 + ddqr1*cos(q2)*cos(q3)*cos(q4)*((117*3^(1/2))/1250 + 37/2000) + ddqr1*cos(q4)*sin(q2)*sin(q3)*((117*3^(1/2))/1250 + 37/2000) + dq1*dqr1*cos(2*q2)*sin(2*q3)*((37*3^(1/2))/4000 - 117/1250) - dq1*dqr1*cos(2*q3)*sin(2*q2)*((37*3^(1/2))/4000 - 117/1250) + (7*3^(1/2)*ddqr1*cos(q2)*sin(q3)*sin(q4))/2000 - (7*3^(1/2)*ddqr1*cos(q3)*sin(q2)*sin(q4))/2000 - (37*3^(1/2)*dq1*dqr1*cos(2*q2)*cos(2*q4)*sin(2*q3))/4000 + (37*3^(1/2)*dq1*dqr1*cos(2*q3)*cos(2*q4)*sin(2*q2))/4000 + (29*3^(1/2)*dq1*dqr1*cos(2*q2)*cos(q3)*sin(q4))/200 - (37*3^(1/2)*dq1*dqr4*cos(2*q4)*cos(q2)*sin(q3))/2000 + (37*3^(1/2)*dq1*dqr4*cos(2*q4)*cos(q3)*sin(q2))/2000 - (37*3^(1/2)*dq4*dqr1*cos(2*q4)*cos(q2)*sin(q3))/2000 + (37*3^(1/2)*dq4*dqr1*cos(2*q4)*cos(q3)*sin(q2))/2000 - dq1*dqr1*cos(2*q2)*cos(2*q3)*sin(q4)*((117*3^(1/2))/1250 + 37/2000) + (29*3^(1/2)*dq1*dqr1*sin(2*q2)*sin(q3)*sin(q4))/200 - dq1*dqr1*sin(2*q2)*sin(2*q3)*sin(q4)*((117*3^(1/2))/1250 + 37/2000) - dq1*dqr4*cos(q2)*cos(q3)*sin(q4)*((117*3^(1/2))/1250 + 37/2000) - dq4*dqr1*cos(q2)*cos(q3)*sin(q4)*((117*3^(1/2))/1250 + 37/2000) - dq1*dqr4*sin(q2)*sin(q3)*sin(q4)*((117*3^(1/2))/1250 + 37/2000) - dq4*dqr1*sin(q2)*sin(q3)*sin(q4)*((117*3^(1/2))/1250 + 37/2000);
Y2_10_1=(29*dq1*dqr1*cos(2*q2)*sin(q3))/400 - (29*dq3*dqr2*sin(q3))/400 - (29*dq1*dqr1*sin(2*q2)*cos(q3))/400 - (87*dq3*dqr2*cos(q5)*sin(q3))/400 - (87*dq5*dqr2*cos(q3)*sin(q5))/400 + (87*dq1*dqr1*cos(2*q2)*cos(q5)*sin(q3))/400 - (87*dq1*dqr1*sin(2*q2)*cos(q3)*cos(q5))/400 + (29*3^(1/2)*dq4*dqr1*cos(q2)*sin(q4))/400 + (37*3^(1/2)*dq5*dqr1*cos(q2)*sin(q3))/4000 - (37*3^(1/2)*dq5*dqr1*cos(q3)*sin(q2))/4000 - (29*3^(1/2)*dq3*dqr2*cos(q3)*sin(q4))/400 - (29*3^(1/2)*dq4*dqr2*cos(q4)*sin(q3))/400 + (111*dq5*dqr1*cos(q2)*cos(q3)*sin(q4))/4000 + dq1*dqr1*cos(2*q2)*sin(2*q3)*((111*3^(1/2))/32000 - 6847/160000) - dq1*dqr1*cos(2*q3)*sin(2*q2)*((111*3^(1/2))/32000 - 6847/160000) + (111*dq5*dqr1*sin(q2)*sin(q3)*sin(q4))/4000 + dq4*dqr1*cos(q2)*sin(q3)*((333*3^(1/2))/16000 + 1923/80000) - dq4*dqr1*cos(q3)*sin(q2)*((333*3^(1/2))/16000 + 1923/80000) + (111*dq4*dqr1*cos(2*q5)*sin(q2)*sin(q3)*sin(q4))/8000 + (111*dq4*dqr1*sin(2*q5)*cos(q4)*sin(q2)*sin(q3))/4000 + (111*dq5*dqr1*cos(2*q5)*sin(q2)*sin(q3)*sin(q4))/4000 + (111*dq5*dqr1*sin(2*q5)*cos(q4)*sin(q2)*sin(q3))/8000 - (29*3^(1/2)*dq4*dqr1*cos(q2)*cos(q4)*sin(q5))/200 - (29*3^(1/2)*dq4*dqr1*cos(q2)*cos(q5)*sin(q4))/400 + (29*3^(1/2)*dq3*dqr2*cos(q3)*cos(q4)*sin(q5))/200 + (29*3^(1/2)*dq3*dqr2*cos(q3)*cos(q5)*sin(q4))/400 - (29*3^(1/2)*dq5*dqr1*cos(q2)*cos(q4)*sin(q5))/400 - (29*3^(1/2)*dq5*dqr1*cos(q2)*cos(q5)*sin(q4))/200 + (29*3^(1/2)*dq4*dqr2*cos(q4)*cos(q5)*sin(q3))/400 + (29*3^(1/2)*dq5*dqr2*cos(q4)*cos(q5)*sin(q3))/200 - (333*3^(1/2)*dq1*dqr1*cos(2*q2)*cos(2*q5)*sin(2*q3))/32000 + (333*3^(1/2)*dq1*dqr1*cos(2*q3)*cos(2*q5)*sin(2*q2))/32000 - dq4*dqr1*cos(2*q4)*cos(q2)*sin(q3)*((37*3^(1/2))/16000 + 1923/80000) + dq4*dqr1*cos(2*q4)*cos(q3)*sin(q2)*((37*3^(1/2))/16000 + 1923/80000) - (29*3^(1/2)*dq4*dqr2*sin(q3)*sin(q4)*sin(q5))/200 - (29*3^(1/2)*dq5*dqr2*sin(q3)*sin(q4)*sin(q5))/400 + (29*3^(1/2)*dq1*dqr1*cos(2*q2)*cos(q3)*sin(q4))/400 - (111*3^(1/2)*dq4*dqr1*cos(2*q5)*cos(q2)*sin(q3))/16000 + (111*3^(1/2)*dq4*dqr1*cos(2*q5)*cos(q3)*sin(q2))/16000 - dq1*dqr1*cos(2*q2)*cos(2*q3)*sin(q4)*((2513*3^(1/2))/40000 - 37/8000) - dq1*dqr1*cos(2*q2)*sin(2*q3)*cos(q5)*((37*3^(1/2))/3200 + 28233/160000) + dq1*dqr1*cos(2*q3)*sin(2*q2)*cos(q5)*((37*3^(1/2))/3200 + 28233/160000) + (29*3^(1/2)*dq1*dqr1*sin(2*q2)*sin(q3)*sin(q4))/400 + (111*dq1*dqr1*cos(2*q2)*cos(2*q3)*cos(2*q5)*sin(q4))/8000 + (111*dq1*dqr1*cos(2*q2)*cos(2*q3)*sin(2*q5)*cos(q4))/4000 - dq1*dqr1*sin(2*q2)*sin(2*q3)*sin(q4)*((2513*3^(1/2))/40000 - 37/8000) + (111*dq1*dqr1*cos(2*q5)*sin(2*q2)*sin(2*q3)*sin(q4))/8000 + (111*dq1*dqr1*sin(2*q2)*sin(2*q3)*sin(2*q5)*cos(q4))/4000 - dq4*dqr1*cos(q2)*cos(q3)*sin(q4)*((2513*3^(1/2))/40000 - 37/8000) - dq4*dqr1*cos(q2)*cos(q5)*sin(q3)*((111*3^(1/2))/8000 + 1923/80000) + dq4*dqr1*cos(q3)*cos(q5)*sin(q2)*((111*3^(1/2))/8000 + 1923/80000) - dq5*dqr1*cos(q2)*cos(q5)*sin(q3)*((111*3^(1/2))/8000 + 1923/80000) + dq5*dqr1*cos(q3)*cos(q5)*sin(q2)*((111*3^(1/2))/8000 + 1923/80000) + (111*dq4*dqr1*cos(2*q5)*cos(q2)*cos(q3)*sin(q4))/8000 + (111*dq4*dqr1*sin(2*q5)*cos(q2)*cos(q3)*cos(q4))/4000 + (111*dq5*dqr1*cos(2*q5)*cos(q2)*cos(q3)*sin(q4))/4000 + (111*dq5*dqr1*sin(2*q5)*cos(q2)*cos(q3)*cos(q4))/8000 - dq1*dqr1*cos(2*q2)*cos(2*q4)*sin(2*q3)*((37*3^(1/2))/32000 + 1923/160000) + dq1*dqr1*cos(2*q3)*cos(2*q4)*sin(2*q2)*((37*3^(1/2))/32000 + 1923/160000) - dq4*dqr1*sin(q2)*sin(q3)*sin(q4)*((2513*3^(1/2))/40000 - 37/8000) + dq4*dqr1*cos(2*q4)*cos(q2)*cos(q5)*sin(q3)*((111*3^(1/2))/8000 + 1923/80000) - dq4*dqr1*cos(2*q4)*cos(q3)*cos(q5)*sin(q2)*((111*3^(1/2))/8000 + 1923/80000) + dq5*dqr1*cos(2*q4)*cos(q2)*cos(q5)*sin(q3)*((111*3^(1/2))/8000 + 1923/80000) - dq5*dqr1*cos(2*q4)*cos(q3)*cos(q5)*sin(q2)*((111*3^(1/2))/8000 + 1923/80000) - dq4*dqr1*sin(2*q4)*cos(q2)*sin(q3)*sin(q5)*((111*3^(1/2))/4000 + 1923/40000) + dq4*dqr1*sin(2*q4)*cos(q3)*sin(q2)*sin(q5)*((111*3^(1/2))/4000 + 1923/40000) - dq5*dqr1*sin(2*q4)*cos(q2)*sin(q3)*sin(q5)*((111*3^(1/2))/16000 + 1923/160000) + dq5*dqr1*sin(2*q4)*cos(q3)*sin(q2)*sin(q5)*((111*3^(1/2))/16000 + 1923/160000) - (29*3^(1/2)*dq1*dqr1*cos(2*q2)*cos(q3)*cos(q4)*sin(q5))/200 - (29*3^(1/2)*dq1*dqr1*cos(2*q2)*cos(q3)*cos(q5)*sin(q4))/400 - (37*3^(1/2)*dq1*dqr1*cos(2*q2)*cos(2*q4)*cos(2*q5)*sin(2*q3))/6400 + (37*3^(1/2)*dq1*dqr1*cos(2*q3)*cos(2*q4)*cos(2*q5)*sin(2*q2))/6400 + dq1*dqr1*cos(2*q2)*cos(2*q3)*cos(q4)*sin(q5)*((877*3^(1/2))/8000 + 37/4000) + dq1*dqr1*cos(2*q2)*cos(2*q3)*cos(q5)*sin(q4)*((1231*3^(1/2))/40000 - 37/1000) - (29*3^(1/2)*dq1*dqr1*sin(2*q2)*cos(q4)*sin(q3)*sin(q5))/200 - (29*3^(1/2)*dq1*dqr1*sin(2*q2)*cos(q5)*sin(q3)*sin(q4))/400 + (37*3^(1/2)*dq1*dqr1*cos(2*q2)*sin(2*q3)*sin(2*q4)*sin(2*q5))/8000 - (37*3^(1/2)*dq1*dqr1*cos(2*q3)*sin(2*q2)*sin(2*q4)*sin(2*q5))/8000 + dq1*dqr1*sin(2*q2)*sin(2*q3)*cos(q4)*sin(q5)*((877*3^(1/2))/8000 + 37/4000) + dq1*dqr1*sin(2*q2)*sin(2*q3)*cos(q5)*sin(q4)*((1231*3^(1/2))/40000 - 37/1000) - (37*3^(1/2)*dq4*dqr1*cos(2*q4)*cos(2*q5)*cos(q2)*sin(q3))/3200 + (37*3^(1/2)*dq4*dqr1*cos(2*q4)*cos(2*q5)*cos(q3)*sin(q2))/3200 - (37*3^(1/2)*dq5*dqr1*cos(2*q4)*cos(2*q5)*cos(q2)*sin(q3))/4000 + (37*3^(1/2)*dq5*dqr1*cos(2*q4)*cos(2*q5)*cos(q3)*sin(q2))/4000 + dq4*dqr1*cos(q2)*cos(q3)*cos(q4)*sin(q5)*((877*3^(1/2))/8000 + 37/4000) + dq5*dqr1*cos(q2)*cos(q3)*cos(q5)*sin(q4)*((877*3^(1/2))/8000 + 37/4000) + dq5*dqr1*cos(q2)*cos(q3)*cos(q4)*sin(q5)*((877*3^(1/2))/16000 + 37/8000) + dq4*dqr1*cos(q2)*cos(q3)*cos(q5)*sin(q4)*((1231*3^(1/2))/40000 - 37/1000) + dq1*dqr1*cos(2*q2)*cos(2*q4)*sin(2*q3)*cos(q5)*((111*3^(1/2))/16000 + 1923/160000) - dq1*dqr1*cos(2*q3)*cos(2*q4)*sin(2*q2)*cos(q5)*((111*3^(1/2))/16000 + 1923/160000) + (37*3^(1/2)*dq4*dqr1*sin(2*q4)*sin(2*q5)*cos(q2)*sin(q3))/4000 - (37*3^(1/2)*dq4*dqr1*sin(2*q4)*sin(2*q5)*cos(q3)*sin(q2))/4000 + (37*3^(1/2)*dq5*dqr1*sin(2*q4)*sin(2*q5)*cos(q2)*sin(q3))/3200 - (37*3^(1/2)*dq5*dqr1*sin(2*q4)*sin(2*q5)*cos(q3)*sin(q2))/3200 + dq4*dqr1*cos(q4)*sin(q2)*sin(q3)*sin(q5)*((877*3^(1/2))/8000 + 37/4000) + dq5*dqr1*cos(q5)*sin(q2)*sin(q3)*sin(q4)*((877*3^(1/2))/8000 + 37/4000) + dq5*dqr1*cos(q4)*sin(q2)*sin(q3)*sin(q5)*((877*3^(1/2))/16000 + 37/8000) + dq4*dqr1*cos(q5)*sin(q2)*sin(q3)*sin(q4)*((1231*3^(1/2))/40000 - 37/1000) - dq1*dqr1*cos(2*q2)*sin(2*q3)*sin(2*q4)*sin(q5)*((111*3^(1/2))/8000 + 1923/80000) + dq1*dqr1*cos(2*q3)*sin(2*q2)*sin(2*q4)*sin(q5)*((111*3^(1/2))/8000 + 1923/80000);
Y2_10_2=(29*dq3*dqr3*sin(q3))/400 - (29*dq2*dqr3*sin(q3))/400 + (111*dq5*dqr4*sin(q4))/4000 - dq4*dqr4*sin(q4)*((2513*3^(1/2))/40000 - 37/8000) - dq5*dqr2*sin(q5)*((37*3^(1/2))/16000 - 24387/160000) + dq5*dqr3*sin(q5)*((37*3^(1/2))/16000 - 24387/160000) + (111*dq4*dqr4*cos(2*q5)*sin(q4))/8000 + (111*dq4*dqr4*sin(2*q5)*cos(q4))/4000 + (111*dq5*dqr4*cos(2*q5)*sin(q4))/4000 + (111*dq5*dqr4*sin(2*q5)*cos(q4))/8000 - dq2*dqr4*sin(2*q4)*((37*3^(1/2))/16000 + 1923/80000) - dq4*dqr2*sin(2*q4)*((37*3^(1/2))/16000 + 1923/80000) + dq3*dqr4*sin(2*q4)*((37*3^(1/2))/16000 + 1923/80000) + dq4*dqr3*sin(2*q4)*((37*3^(1/2))/16000 + 1923/80000) + (111*3^(1/2)*dq5*dqr2*sin(2*q5))/16000 - (111*3^(1/2)*dq5*dqr3*sin(2*q5))/16000 - (87*dq2*dqr3*cos(q5)*sin(q3))/400 + (87*dq3*dqr3*cos(q5)*sin(q3))/400 + (87*dq5*dqr3*cos(q3)*sin(q5))/400 + (29*3^(1/2)*dq1*dqr4*cos(q2)*sin(q4))/400 - (29*3^(1/2)*dq2*dqr3*cos(q3)*sin(q4))/400 - (29*3^(1/2)*dq2*dqr4*cos(q4)*sin(q3))/400 + (29*3^(1/2)*dq3*dqr3*cos(q3)*sin(q4))/400 + (29*3^(1/2)*dq3*dqr4*cos(q4)*sin(q3))/400 + (29*3^(1/2)*dq4*dqr3*cos(q4)*sin(q3))/400 + (29*3^(1/2)*dq4*dqr4*cos(q3)*sin(q4))/400 + dq2*dqr4*cos(2*q4)*sin(q5)*((111*3^(1/2))/4000 + 1923/40000) + dq4*dqr2*cos(2*q4)*sin(q5)*((111*3^(1/2))/4000 + 1923/40000) - dq3*dqr4*cos(2*q4)*sin(q5)*((111*3^(1/2))/4000 + 1923/40000) - dq4*dqr3*cos(2*q4)*sin(q5)*((111*3^(1/2))/4000 + 1923/40000) + dq2*dqr4*sin(2*q4)*cos(q5)*((111*3^(1/2))/8000 + 1923/80000) + dq4*dqr2*sin(2*q4)*cos(q5)*((111*3^(1/2))/8000 + 1923/80000) - dq3*dqr4*sin(2*q4)*cos(q5)*((111*3^(1/2))/8000 + 1923/80000) - dq4*dqr3*sin(2*q4)*cos(q5)*((111*3^(1/2))/8000 + 1923/80000) + dq5*dqr2*sin(2*q4)*cos(q5)*((111*3^(1/2))/8000 + 1923/80000) - dq5*dqr3*sin(2*q4)*cos(q5)*((111*3^(1/2))/8000 + 1923/80000) + dq5*dqr2*cos(2*q4)*sin(q5)*((111*3^(1/2))/16000 + 1923/160000) - dq5*dqr3*cos(2*q4)*sin(q5)*((111*3^(1/2))/16000 + 1923/160000) - (37*3^(1/2)*dq2*dqr4*cos(2*q4)*sin(2*q5))/4000 - (37*3^(1/2)*dq2*dqr4*cos(2*q5)*sin(2*q4))/3200 - (37*3^(1/2)*dq4*dqr2*cos(2*q4)*sin(2*q5))/4000 - (37*3^(1/2)*dq4*dqr2*cos(2*q5)*sin(2*q4))/3200 + (37*3^(1/2)*dq3*dqr4*cos(2*q4)*sin(2*q5))/4000 + (37*3^(1/2)*dq3*dqr4*cos(2*q5)*sin(2*q4))/3200 + (37*3^(1/2)*dq4*dqr3*cos(2*q4)*sin(2*q5))/4000 + (37*3^(1/2)*dq4*dqr3*cos(2*q5)*sin(2*q4))/3200 - (37*3^(1/2)*dq5*dqr2*cos(2*q4)*sin(2*q5))/3200 - (37*3^(1/2)*dq5*dqr2*cos(2*q5)*sin(2*q4))/4000 + (37*3^(1/2)*dq5*dqr3*cos(2*q4)*sin(2*q5))/3200 + (37*3^(1/2)*dq5*dqr3*cos(2*q5)*sin(2*q4))/4000 + dq4*dqr4*cos(q4)*sin(q5)*((877*3^(1/2))/8000 + 37/4000) + dq5*dqr4*cos(q5)*sin(q4)*((877*3^(1/2))/8000 + 37/4000) + dq5*dqr4*cos(q4)*sin(q5)*((877*3^(1/2))/16000 + 37/8000) + dq4*dqr4*cos(q5)*sin(q4)*((1231*3^(1/2))/40000 - 37/1000) + dq1*dqr4*cos(q2)*sin(q3)*((333*3^(1/2))/16000 + 1923/80000) - dq1*dqr4*cos(q3)*sin(q2)*((333*3^(1/2))/16000 + 1923/80000) + (111*dq1*dqr4*cos(2*q5)*sin(q2)*sin(q3)*sin(q4))/8000 + (111*dq1*dqr4*sin(2*q5)*cos(q4)*sin(q2)*sin(q3))/4000 + (111*dq1*dqr5*cos(2*q5)*sin(q2)*sin(q3)*sin(q4))/4000 - (29*3^(1/2)*dq1*dqr4*cos(q2)*cos(q4)*sin(q5))/200 - (29*3^(1/2)*dq1*dqr4*cos(q2)*cos(q5)*sin(q4))/400 + (29*3^(1/2)*dq2*dqr3*cos(q3)*cos(q4)*sin(q5))/200 + (29*3^(1/2)*dq2*dqr3*cos(q3)*cos(q5)*sin(q4))/400 + (29*3^(1/2)*dq2*dqr4*cos(q4)*cos(q5)*sin(q3))/400 - (29*3^(1/2)*dq3*dqr3*cos(q3)*cos(q4)*sin(q5))/200 - (29*3^(1/2)*dq3*dqr3*cos(q3)*cos(q5)*sin(q4))/400 - (29*3^(1/2)*dq3*dqr4*cos(q4)*cos(q5)*sin(q3))/400 - (29*3^(1/2)*dq4*dqr3*cos(q4)*cos(q5)*sin(q3))/400 - (29*3^(1/2)*dq4*dqr4*cos(q3)*cos(q4)*sin(q5))/200 - (29*3^(1/2)*dq4*dqr4*cos(q3)*cos(q5)*sin(q4))/400 - (29*3^(1/2)*dq5*dqr3*cos(q4)*cos(q5)*sin(q3))/200 - (29*3^(1/2)*dq5*dqr4*cos(q3)*cos(q4)*sin(q5))/400 - (29*3^(1/2)*dq5*dqr4*cos(q3)*cos(q5)*sin(q4))/200 - dq1*dqr4*cos(2*q4)*cos(q2)*sin(q3)*((37*3^(1/2))/16000 + 1923/80000) + dq1*dqr4*cos(2*q4)*cos(q3)*sin(q2)*((37*3^(1/2))/16000 + 1923/80000) - (29*3^(1/2)*dq2*dqr4*sin(q3)*sin(q4)*sin(q5))/200 + (29*3^(1/2)*dq3*dqr4*sin(q3)*sin(q4)*sin(q5))/200 + (29*3^(1/2)*dq4*dqr3*sin(q3)*sin(q4)*sin(q5))/200 + (29*3^(1/2)*dq5*dqr3*sin(q3)*sin(q4)*sin(q5))/400 - (111*3^(1/2)*dq1*dqr4*cos(2*q5)*cos(q2)*sin(q3))/16000 + (111*3^(1/2)*dq1*dqr4*cos(2*q5)*cos(q3)*sin(q2))/16000 - dq1*dqr4*cos(q2)*cos(q3)*sin(q4)*((2513*3^(1/2))/40000 - 37/8000) - dq1*dqr4*cos(q2)*cos(q5)*sin(q3)*((111*3^(1/2))/8000 + 1923/80000) + dq1*dqr4*cos(q3)*cos(q5)*sin(q2)*((111*3^(1/2))/8000 + 1923/80000) + (111*dq1*dqr4*cos(2*q5)*cos(q2)*cos(q3)*sin(q4))/8000 + (111*dq1*dqr4*sin(2*q5)*cos(q2)*cos(q3)*cos(q4))/4000 - dq1*dqr4*sin(q2)*sin(q3)*sin(q4)*((2513*3^(1/2))/40000 - 37/8000) + dq1*dqr4*cos(2*q4)*cos(q2)*cos(q5)*sin(q3)*((111*3^(1/2))/8000 + 1923/80000) - dq1*dqr4*cos(2*q4)*cos(q3)*cos(q5)*sin(q2)*((111*3^(1/2))/8000 + 1923/80000) - dq1*dqr4*sin(2*q4)*cos(q2)*sin(q3)*sin(q5)*((111*3^(1/2))/4000 + 1923/40000) + dq1*dqr4*sin(2*q4)*cos(q3)*sin(q2)*sin(q5)*((111*3^(1/2))/4000 + 1923/40000) - (37*3^(1/2)*dq1*dqr4*cos(2*q4)*cos(2*q5)*cos(q2)*sin(q3))/3200 + (37*3^(1/2)*dq1*dqr4*cos(2*q4)*cos(2*q5)*cos(q3)*sin(q2))/3200 + dq1*dqr4*cos(q2)*cos(q3)*cos(q4)*sin(q5)*((877*3^(1/2))/8000 + 37/4000) + dq1*dqr4*cos(q2)*cos(q3)*cos(q5)*sin(q4)*((1231*3^(1/2))/40000 - 37/1000) + (37*3^(1/2)*dq1*dqr4*sin(2*q4)*sin(2*q5)*cos(q2)*sin(q3))/4000 - (37*3^(1/2)*dq1*dqr4*sin(2*q4)*sin(2*q5)*cos(q3)*sin(q2))/4000 + dq1*dqr4*cos(q4)*sin(q2)*sin(q3)*sin(q5)*((877*3^(1/2))/8000 + 37/4000) + dq1*dqr5*cos(q5)*sin(q2)*sin(q3)*sin(q4)*((877*3^(1/2))/8000 + 37/4000) + dq1*dqr4*cos(q5)*sin(q2)*sin(q3)*sin(q4)*((1231*3^(1/2))/40000 - 37/1000);
Y2_10_3=(111*dq4*dqr5*sin(q4))/4000 - (7*ddqr1*cos(q2)*cos(q3))/4000 + (87*ddqr2*cos(q3)*cos(q5))/200 - (7*ddqr1*sin(q2)*sin(q3))/4000 + (87*ddqr5*sin(q3)*sin(q5))/400 + (111*ddqr4*sin(2*q5)*sin(q4))/4000 + ddqr2*sin(2*q4)*sin(q5)*((111*3^(1/2))/4000 + 1923/40000) - ddqr3*sin(2*q4)*sin(q5)*((111*3^(1/2))/4000 + 1923/40000) - dq2*dqr5*sin(q5)*((37*3^(1/2))/16000 - 24387/160000) + dq3*dqr5*sin(q5)*((37*3^(1/2))/16000 - 24387/160000) + (111*dq4*dqr5*cos(2*q5)*sin(q4))/4000 + (111*dq4*dqr5*sin(2*q5)*cos(q4))/8000 - (21*ddqr1*cos(q2)*cos(q3)*cos(q5))/4000 - (21*ddqr1*cos(q5)*sin(q2)*sin(q3))/4000 + ddqr4*sin(q4)*sin(q5)*((877*3^(1/2))/8000 + 37/4000) + ddqr5*sin(q4)*sin(q5)*((1577*3^(1/2))/20000 + 37/800) + (111*3^(1/2)*dq2*dqr5*sin(2*q5))/16000 - (111*3^(1/2)*dq3*dqr5*sin(2*q5))/16000 - (29*3^(1/2)*ddqr1*cos(q2)*cos(q4))/400 - (87*dq2*dqr5*cos(q3)*sin(q5))/400 + (87*dq3*dqr5*cos(q3)*sin(q5))/400 + (87*dq5*dqr5*cos(q5)*sin(q3))/400 - (29*3^(1/2)*ddqr2*sin(q3)*sin(q4))/200 + (29*3^(1/2)*ddqr3*sin(q3)*sin(q4))/400 + (37*3^(1/2)*dq1*dqr5*cos(q2)*sin(q3))/4000 - (37*3^(1/2)*dq1*dqr5*cos(q3)*sin(q2))/4000 + dq2*dqr5*sin(2*q4)*cos(q5)*((111*3^(1/2))/8000 + 1923/80000) - dq3*dqr5*sin(2*q4)*cos(q5)*((111*3^(1/2))/8000 + 1923/80000) + dq2*dqr5*cos(2*q4)*sin(q5)*((111*3^(1/2))/16000 + 1923/160000) - dq3*dqr5*cos(2*q4)*sin(q5)*((111*3^(1/2))/16000 + 1923/160000) + ddqr1*cos(q2)*cos(q3)*cos(q4)*((2513*3^(1/2))/40000 - 37/8000) - (111*ddqr1*cos(2*q5)*cos(q2)*cos(q3)*cos(q4))/8000 + ddqr1*cos(q4)*sin(q2)*sin(q3)*((2513*3^(1/2))/40000 - 37/8000) - (111*ddqr1*cos(2*q5)*cos(q4)*sin(q2)*sin(q3))/8000 + (111*ddqr1*sin(2*q5)*cos(q2)*cos(q3)*sin(q4))/4000 + (29*3^(1/2)*ddqr1*cos(q2)*cos(q4)*cos(q5))/400 + (111*ddqr1*sin(2*q5)*sin(q2)*sin(q3)*sin(q4))/4000 + (111*dq1*dqr5*cos(q2)*cos(q3)*sin(q4))/4000 + (7*3^(1/2)*ddqr1*cos(q2)*sin(q3)*sin(q4))/4000 - (7*3^(1/2)*ddqr1*cos(q3)*sin(q2)*sin(q4))/4000 - (29*3^(1/2)*ddqr1*cos(q2)*sin(q4)*sin(q5))/200 + (29*3^(1/2)*ddqr2*cos(q4)*sin(q3)*sin(q5))/100 + (29*3^(1/2)*ddqr2*cos(q5)*sin(q3)*sin(q4))/200 - (29*3^(1/2)*ddqr3*cos(q4)*sin(q3)*sin(q5))/200 - (29*3^(1/2)*ddqr3*cos(q5)*sin(q3)*sin(q4))/400 - (29*3^(1/2)*ddqr4*cos(q3)*sin(q4)*sin(q5))/200 - (29*3^(1/2)*ddqr5*cos(q3)*sin(q4)*sin(q5))/400 + (111*dq1*dqr5*sin(q2)*sin(q3)*sin(q4))/4000 - ddqr1*sin(2*q4)*cos(q2)*sin(q3)*((37*3^(1/2))/16000 + 1923/80000) + ddqr1*sin(2*q4)*cos(q3)*sin(q2)*((37*3^(1/2))/16000 + 1923/80000) - (37*3^(1/2)*dq2*dqr5*cos(2*q4)*sin(2*q5))/3200 - (37*3^(1/2)*dq2*dqr5*cos(2*q5)*sin(2*q4))/4000 + (37*3^(1/2)*dq3*dqr5*cos(2*q4)*sin(2*q5))/3200 + (37*3^(1/2)*dq3*dqr5*cos(2*q5)*sin(2*q4))/4000 + dq4*dqr5*cos(q5)*sin(q4)*((877*3^(1/2))/8000 + 37/4000) + dq5*dqr5*cos(q4)*sin(q5)*((877*3^(1/2))/8000 + 37/4000) + dq5*dqr5*cos(q5)*sin(q4)*((1577*3^(1/2))/20000 + 37/800) + dq4*dqr5*cos(q4)*sin(q5)*((877*3^(1/2))/16000 + 37/8000) + (111*dq1*dqr5*sin(2*q5)*cos(q4)*sin(q2)*sin(q3))/8000 - (29*3^(1/2)*dq1*dqr5*cos(q2)*cos(q4)*sin(q5))/400 - (29*3^(1/2)*dq1*dqr5*cos(q2)*cos(q5)*sin(q4))/200 + (29*3^(1/2)*dq2*dqr5*cos(q4)*cos(q5)*sin(q3))/200 - (29*3^(1/2)*dq3*dqr5*cos(q4)*cos(q5)*sin(q3))/200 - (29*3^(1/2)*dq4*dqr5*cos(q3)*cos(q4)*sin(q5))/400 - (29*3^(1/2)*dq4*dqr5*cos(q3)*cos(q5)*sin(q4))/200 - (29*3^(1/2)*dq5*dqr5*cos(q3)*cos(q4)*sin(q5))/200 - (29*3^(1/2)*dq5*dqr5*cos(q3)*cos(q5)*sin(q4))/400 - ddqr1*cos(q2)*cos(q3)*cos(q4)*cos(q5)*((1231*3^(1/2))/40000 - 37/1000) - (29*3^(1/2)*dq2*dqr5*sin(q3)*sin(q4)*sin(q5))/400 + (29*3^(1/2)*dq3*dqr5*sin(q3)*sin(q4)*sin(q5))/400 - (37*3^(1/2)*ddqr1*cos(2*q4)*sin(2*q5)*cos(q2)*sin(q3))/4000 + (37*3^(1/2)*ddqr1*cos(2*q4)*sin(2*q5)*cos(q3)*sin(q2))/4000 - (37*3^(1/2)*ddqr1*cos(2*q5)*sin(2*q4)*cos(q2)*sin(q3))/3200 + (37*3^(1/2)*ddqr1*cos(2*q5)*sin(2*q4)*cos(q3)*sin(q2))/3200 + ddqr1*cos(q2)*cos(q3)*sin(q4)*sin(q5)*((877*3^(1/2))/8000 + 37/4000) - ddqr1*cos(q4)*cos(q5)*sin(q2)*sin(q3)*((1231*3^(1/2))/40000 - 37/1000) + ddqr1*sin(q2)*sin(q3)*sin(q4)*sin(q5)*((877*3^(1/2))/8000 + 37/4000) - (7*3^(1/2)*ddqr1*cos(q2)*cos(q4)*sin(q3)*sin(q5))/2000 - (7*3^(1/2)*ddqr1*cos(q2)*cos(q5)*sin(q3)*sin(q4))/4000 + (7*3^(1/2)*ddqr1*cos(q3)*cos(q4)*sin(q2)*sin(q5))/2000 + (7*3^(1/2)*ddqr1*cos(q3)*cos(q5)*sin(q2)*sin(q4))/4000 + ddqr1*cos(2*q4)*cos(q2)*sin(q3)*sin(q5)*((111*3^(1/2))/4000 + 1923/40000) - ddqr1*cos(2*q4)*cos(q3)*sin(q2)*sin(q5)*((111*3^(1/2))/4000 + 1923/40000) + ddqr1*sin(2*q4)*cos(q2)*cos(q5)*sin(q3)*((111*3^(1/2))/8000 + 1923/80000) - ddqr1*sin(2*q4)*cos(q3)*cos(q5)*sin(q2)*((111*3^(1/2))/8000 + 1923/80000) - dq1*dqr5*cos(q2)*cos(q5)*sin(q3)*((111*3^(1/2))/8000 + 1923/80000) + dq1*dqr5*cos(q3)*cos(q5)*sin(q2)*((111*3^(1/2))/8000 + 1923/80000) + (111*dq1*dqr5*cos(2*q5)*cos(q2)*cos(q3)*sin(q4))/4000 + (111*dq1*dqr5*sin(2*q5)*cos(q2)*cos(q3)*cos(q4))/8000 + dq1*dqr5*cos(2*q4)*cos(q2)*cos(q5)*sin(q3)*((111*3^(1/2))/8000 + 1923/80000) - dq1*dqr5*cos(2*q4)*cos(q3)*cos(q5)*sin(q2)*((111*3^(1/2))/8000 + 1923/80000) - dq1*dqr5*sin(2*q4)*cos(q2)*sin(q3)*sin(q5)*((111*3^(1/2))/16000 + 1923/160000) + dq1*dqr5*sin(2*q4)*cos(q3)*sin(q2)*sin(q5)*((111*3^(1/2))/16000 + 1923/160000) - (37*3^(1/2)*dq1*dqr5*cos(2*q4)*cos(2*q5)*cos(q2)*sin(q3))/4000 + (37*3^(1/2)*dq1*dqr5*cos(2*q4)*cos(2*q5)*cos(q3)*sin(q2))/4000 + dq1*dqr5*cos(q2)*cos(q3)*cos(q5)*sin(q4)*((877*3^(1/2))/8000 + 37/4000) + dq1*dqr5*cos(q2)*cos(q3)*cos(q4)*sin(q5)*((877*3^(1/2))/16000 + 37/8000) + (37*3^(1/2)*dq1*dqr5*sin(2*q4)*sin(2*q5)*cos(q2)*sin(q3))/3200 - (37*3^(1/2)*dq1*dqr5*sin(2*q4)*sin(2*q5)*cos(q3)*sin(q2))/3200 + dq1*dqr5*cos(q4)*sin(q2)*sin(q3)*sin(q5)*((877*3^(1/2))/16000 + 37/8000);
Y2_10_4=(29*ddqr2*cos(q3))/200 - (29*ddqr3*cos(q3))/400 - (111*ddqr5*cos(q4))/2000 - ddqr2*((111*3^(1/2))/3200 + 10693/80000) + ddqr3*((111*3^(1/2))/3200 + 10693/80000) + ddqr2*cos(2*q4)*((37*3^(1/2))/16000 + 1923/80000) - ddqr3*cos(2*q4)*((37*3^(1/2))/16000 + 1923/80000) - (111*3^(1/2)*ddqr2*cos(2*q5))/16000 + (111*3^(1/2)*ddqr3*cos(2*q5))/16000 - (87*ddqr3*cos(q3)*cos(q5))/400 + ddqr4*cos(q4)*((2513*3^(1/2))/40000 - 37/8000) + ddqr2*cos(q5)*((37*3^(1/2))/8000 - 24387/80000) - ddqr3*cos(q5)*((37*3^(1/2))/8000 - 24387/80000) - (111*ddqr4*cos(2*q5)*cos(q4))/8000 + (37*3^(1/2)*ddqr2*cos(2*q4)*cos(2*q5))/3200 - (37*3^(1/2)*ddqr3*cos(2*q4)*cos(2*q5))/3200 - ddqr5*cos(q4)*cos(q5)*((877*3^(1/2))/8000 + 37/4000) - ddqr4*cos(q4)*cos(q5)*((1231*3^(1/2))/40000 - 37/1000) - (37*3^(1/2)*ddqr2*sin(2*q4)*sin(2*q5))/4000 + (37*3^(1/2)*ddqr3*sin(2*q4)*sin(2*q5))/4000 - (29*3^(1/2)*ddqr4*cos(q3)*cos(q4))/400 - ddqr2*cos(2*q4)*cos(q5)*((111*3^(1/2))/8000 + 1923/80000) + ddqr3*cos(2*q4)*cos(q5)*((111*3^(1/2))/8000 + 1923/80000) + (29*3^(1/2)*ddqr4*cos(q3)*cos(q4)*cos(q5))/400 + (29*3^(1/2)*ddqr5*cos(q3)*cos(q4)*cos(q5))/200;
Y2_11_1=(29*sin(q2))/100;
Y2_12_1=(29*sin(q2))/100 - (1231*sin(q2 - q3))/10000;
Y2_13_1=(37*sin(q2 - q3 + q4))/2000 - (117*sin(q2 - q3))/625 + (37*sin(q3 - q2 + q4))/2000 + (29*sin(q2))/100;
Y2_14_1=(37*sin(q2 - q3 + q4 - q5))/8000 - (877*sin(q2 - q3))/4000 - (37*sin(q2 - q3 - q4 + q5))/8000 + (29*sin(q2))/100 - (111*sin(q2 - q3 + q4 + q5))/8000 - (111*sin(q3 - q2 + q4 + q5))/8000 + sin(q2 - q3 + q4)*((641*3^(1/2))/40000 + 37/2000) + sin(q3 - q2 + q4)*((641*3^(1/2))/40000 + 37/2000) - (37*3^(1/2)*sin(q2 - q3 + q5))/4000 + (37*3^(1/2)*sin(q3 - q2 + q5))/4000;
Y2_15_1=ddqr2 - (dq1*dqr1*sin(2*q2))/2;
Y2_16_1=ddqr2 - ddqr3 + (dq1*dqr1*cos(2*q2)*sin(2*q3))/2 - (dq1*dqr1*cos(2*q3)*sin(2*q2))/2;
Y2_17_1=ddqr2 - ddqr3 + (dq1*dqr1*cos(2*q2)*sin(2*q3))/2 - (dq1*dqr1*cos(2*q3)*sin(2*q2))/2;
Y2_18_1=(5*ddqr2)/8 - (5*ddqr3)/8 - (3*ddqr2*cos(2*q4))/8 + (3*ddqr3*cos(2*q4))/8 + (3*dq2*dqr4*sin(2*q4))/8 + (3*dq4*dqr2*sin(2*q4))/8 - (3*dq3*dqr4*sin(2*q4))/8 - (3*dq4*dqr3*sin(2*q4))/8 - (3^(1/2)*ddqr4*cos(q4))/4 + (3^(1/2)*dq4*dqr4*sin(q4))/4 - (dq1*dqr1*cos(2*q2)*sin(2*q3))/16 + (dq1*dqr1*cos(2*q3)*sin(2*q2))/16 + (3*ddqr1*sin(2*q4)*cos(q2)*sin(q3))/8 - (3*ddqr1*sin(2*q4)*cos(q3)*sin(q2))/8 - (3*dq1*dqr4*cos(q2)*sin(q3))/8 + (3*dq1*dqr4*cos(q3)*sin(q2))/8 - (3*dq4*dqr1*cos(q2)*sin(q3))/8 + (3*dq4*dqr1*cos(q3)*sin(q2))/8 + (3*dq1*dqr4*cos(2*q4)*cos(q2)*sin(q3))/8 - (3*dq1*dqr4*cos(2*q4)*cos(q3)*sin(q2))/8 + (3*dq4*dqr1*cos(2*q4)*cos(q2)*sin(q3))/8 - (3*dq4*dqr1*cos(2*q4)*cos(q3)*sin(q2))/8 - (3^(1/2)*ddqr1*cos(q2)*cos(q3)*cos(q4))/4 - (3^(1/2)*ddqr1*cos(q4)*sin(q2)*sin(q3))/4 + (3*dq1*dqr1*cos(2*q2)*cos(2*q4)*sin(2*q3))/16 - (3*dq1*dqr1*cos(2*q3)*cos(2*q4)*sin(2*q2))/16 + (3^(1/2)*dq1*dqr4*cos(q2)*cos(q3)*sin(q4))/4 + (3^(1/2)*dq4*dqr1*cos(q2)*cos(q3)*sin(q4))/4 + (3^(1/2)*dq1*dqr4*sin(q2)*sin(q3)*sin(q4))/4 + (3^(1/2)*dq4*dqr1*sin(q2)*sin(q3)*sin(q4))/4 + (3^(1/2)*dq1*dqr1*cos(2*q2)*cos(2*q3)*sin(q4))/4 + (3^(1/2)*dq1*dqr1*sin(2*q2)*sin(2*q3)*sin(q4))/4;
Y2_19_1=(3*dq5*dqr3*sin(q5))/32 - (3*dq5*dqr2*sin(q5))/32 - (3*dq4*dqr2*sin(2*q4))/64 + (3*dq4*dqr3*sin(2*q4))/64 - (9*dq5*dqr2*sin(2*q5))/64 + (9*dq5*dqr3*sin(2*q5))/64 - (3*dq4*dqr2*cos(2*q4)*sin(q5))/8 - (3*dq4*dqr2*sin(2*q4)*cos(q5))/16 + (3*dq4*dqr3*cos(2*q4)*sin(q5))/8 + (3*dq4*dqr3*sin(2*q4)*cos(q5))/16 - (3*dq5*dqr2*cos(2*q4)*sin(q5))/32 - (3*dq5*dqr2*sin(2*q4)*cos(q5))/16 + (3*dq5*dqr3*cos(2*q4)*sin(q5))/32 + (3*dq5*dqr3*sin(2*q4)*cos(q5))/16 + (dq1*dqr1*cos(2*q2)*sin(2*q3))/128 - (dq1*dqr1*cos(2*q3)*sin(2*q2))/128 + (3*dq4*dqr2*cos(2*q4)*sin(2*q5))/16 + (15*dq4*dqr2*cos(2*q5)*sin(2*q4))/64 - (3*dq4*dqr3*cos(2*q4)*sin(2*q5))/16 - (15*dq4*dqr3*cos(2*q5)*sin(2*q4))/64 + (15*dq5*dqr2*cos(2*q4)*sin(2*q5))/64 + (3*dq5*dqr2*cos(2*q5)*sin(2*q4))/16 - (15*dq5*dqr3*cos(2*q4)*sin(2*q5))/64 - (3*dq5*dqr3*cos(2*q5)*sin(2*q4))/16 - (21*dq4*dqr1*cos(q2)*sin(q3))/64 + (21*dq4*dqr1*cos(q3)*sin(q2))/64 - (3*dq5*dqr1*cos(q2)*sin(q3))/16 + (3*dq5*dqr1*cos(q3)*sin(q2))/16 - (3*dq4*dqr1*cos(2*q4)*cos(q2)*sin(q3))/64 + (3*dq4*dqr1*cos(2*q4)*cos(q3)*sin(q2))/64 + (9*dq4*dqr1*cos(2*q5)*cos(q2)*sin(q3))/64 - (9*dq4*dqr1*cos(2*q5)*cos(q3)*sin(q2))/64 + (9*dq1*dqr1*cos(2*q2)*sin(2*q3)*cos(q5))/32 - (9*dq1*dqr1*cos(2*q3)*sin(2*q2)*cos(q5))/32 + (3*dq4*dqr1*cos(q2)*cos(q5)*sin(q3))/16 - (3*dq4*dqr1*cos(q3)*cos(q5)*sin(q2))/16 + (3*dq5*dqr1*cos(q2)*cos(q5)*sin(q3))/16 - (3*dq5*dqr1*cos(q3)*cos(q5)*sin(q2))/16 - (3*dq1*dqr1*cos(2*q2)*cos(2*q4)*sin(2*q3))/128 + (3*dq1*dqr1*cos(2*q3)*cos(2*q4)*sin(2*q2))/128 + (27*dq1*dqr1*cos(2*q2)*cos(2*q5)*sin(2*q3))/128 - (27*dq1*dqr1*cos(2*q3)*cos(2*q5)*sin(2*q2))/128 + (15*dq1*dqr1*cos(2*q2)*cos(2*q4)*cos(2*q5)*sin(2*q3))/128 - (15*dq1*dqr1*cos(2*q3)*cos(2*q4)*cos(2*q5)*sin(2*q2))/128 + (3*dq4*dqr1*sin(2*q4)*cos(q2)*sin(q3)*sin(q5))/8 - (3*dq4*dqr1*sin(2*q4)*cos(q3)*sin(q2)*sin(q5))/8 + (3*dq5*dqr1*sin(2*q4)*cos(q2)*sin(q3)*sin(q5))/32 - (3*dq5*dqr1*sin(2*q4)*cos(q3)*sin(q2)*sin(q5))/32 - (3^(1/2)*dq4*dqr1*cos(q2)*cos(q3)*sin(q4))/32 - (3*3^(1/2)*dq5*dqr1*cos(q2)*cos(q3)*sin(q4))/16 - (3*dq1*dqr1*cos(2*q2)*sin(2*q3)*sin(2*q4)*sin(2*q5))/32 + (3*dq1*dqr1*cos(2*q3)*sin(2*q2)*sin(2*q4)*sin(2*q5))/32 - (3^(1/2)*dq1*dqr4*sin(q2)*sin(q3)*sin(q4))/32 - (3^(1/2)*dq4*dqr1*sin(q2)*sin(q3)*sin(q4))/32 - (3*3^(1/2)*dq5*dqr1*sin(q2)*sin(q3)*sin(q4))/16 + (15*dq4*dqr1*cos(2*q4)*cos(2*q5)*cos(q2)*sin(q3))/64 - (15*dq4*dqr1*cos(2*q4)*cos(2*q5)*cos(q3)*sin(q2))/64 + (3*dq5*dqr1*cos(2*q4)*cos(2*q5)*cos(q2)*sin(q3))/16 - (3*dq5*dqr1*cos(2*q4)*cos(2*q5)*cos(q3)*sin(q2))/16 - (3*dq4*dqr1*sin(2*q4)*sin(2*q5)*cos(q2)*sin(q3))/16 + (3*dq4*dqr1*sin(2*q4)*sin(2*q5)*cos(q3)*sin(q2))/16 - (15*dq5*dqr1*sin(2*q4)*sin(2*q5)*cos(q2)*sin(q3))/64 + (15*dq5*dqr1*sin(2*q4)*sin(2*q5)*cos(q3)*sin(q2))/64 - (3*dq1*dqr1*cos(2*q2)*cos(2*q4)*sin(2*q3)*cos(q5))/32 + (3*dq1*dqr1*cos(2*q3)*cos(2*q4)*sin(2*q2)*cos(q5))/32 + (3*dq1*dqr1*cos(2*q2)*sin(2*q3)*sin(2*q4)*sin(q5))/16 - (3*dq1*dqr1*cos(2*q3)*sin(2*q2)*sin(2*q4)*sin(q5))/16 - (3^(1/2)*dq1*dqr1*cos(2*q2)*cos(2*q3)*sin(q4))/32 - (3*dq4*dqr1*cos(2*q4)*cos(q2)*cos(q5)*sin(q3))/16 + (3*dq4*dqr1*cos(2*q4)*cos(q3)*cos(q5)*sin(q2))/16 - (3*dq5*dqr1*cos(2*q4)*cos(q2)*cos(q5)*sin(q3))/16 + (3*dq5*dqr1*cos(2*q4)*cos(q3)*cos(q5)*sin(q2))/16 - (3^(1/2)*dq1*dqr1*sin(2*q2)*sin(2*q3)*sin(q4))/32 - (3*3^(1/2)*dq1*dqr1*cos(2*q2)*cos(2*q3)*cos(2*q5)*sin(q4))/32 - (3*3^(1/2)*dq1*dqr1*cos(2*q2)*cos(2*q3)*sin(2*q5)*cos(q4))/16 - (3^(1/2)*dq1*dqr4*cos(q4)*sin(q2)*sin(q3)*sin(q5))/8 + (3^(1/2)*dq1*dqr4*cos(q5)*sin(q2)*sin(q3)*sin(q4))/8 - (3^(1/2)*dq4*dqr1*cos(q4)*sin(q2)*sin(q3)*sin(q5))/8 + (3^(1/2)*dq4*dqr1*cos(q5)*sin(q2)*sin(q3)*sin(q4))/8 - (3^(1/2)*dq5*dqr1*cos(q4)*sin(q2)*sin(q3)*sin(q5))/16 - (3^(1/2)*dq5*dqr1*cos(q5)*sin(q2)*sin(q3)*sin(q4))/8 - (3*3^(1/2)*dq1*dqr1*cos(2*q5)*sin(2*q2)*sin(2*q3)*sin(q4))/32 - (3*3^(1/2)*dq1*dqr1*sin(2*q2)*sin(2*q3)*sin(2*q5)*cos(q4))/16 - (3*3^(1/2)*dq4*dqr1*cos(2*q5)*cos(q2)*cos(q3)*sin(q4))/32 - (3*3^(1/2)*dq4*dqr1*sin(2*q5)*cos(q2)*cos(q3)*cos(q4))/16 - (3*3^(1/2)*dq5*dqr1*cos(2*q5)*cos(q2)*cos(q3)*sin(q4))/16 - (3*3^(1/2)*dq5*dqr1*sin(2*q5)*cos(q2)*cos(q3)*cos(q4))/32 - (3*3^(1/2)*dq1*dqr4*cos(2*q5)*sin(q2)*sin(q3)*sin(q4))/32 - (3*3^(1/2)*dq4*dqr1*cos(2*q5)*sin(q2)*sin(q3)*sin(q4))/32 - (3*3^(1/2)*dq4*dqr1*sin(2*q5)*cos(q4)*sin(q2)*sin(q3))/16 - (3*3^(1/2)*dq5*dqr1*cos(2*q5)*sin(q2)*sin(q3)*sin(q4))/16 - (3*3^(1/2)*dq5*dqr1*sin(2*q5)*cos(q4)*sin(q2)*sin(q3))/32 - (3^(1/2)*dq1*dqr1*cos(2*q2)*cos(2*q3)*cos(q4)*sin(q5))/8 + (3^(1/2)*dq1*dqr1*cos(2*q2)*cos(2*q3)*cos(q5)*sin(q4))/8 - (3^(1/2)*dq1*dqr1*sin(2*q2)*sin(2*q3)*cos(q4)*sin(q5))/8 + (3^(1/2)*dq1*dqr1*sin(2*q2)*sin(2*q3)*cos(q5)*sin(q4))/8 - (3^(1/2)*dq4*dqr1*cos(q2)*cos(q3)*cos(q4)*sin(q5))/8 + (3^(1/2)*dq4*dqr1*cos(q2)*cos(q3)*cos(q5)*sin(q4))/8 - (3^(1/2)*dq5*dqr1*cos(q2)*cos(q3)*cos(q4)*sin(q5))/16 - (3^(1/2)*dq5*dqr1*cos(q2)*cos(q3)*cos(q5)*sin(q4))/8;
Y2_19_2=(3*dq3*dqr5*sin(q5))/32 - (3*dq2*dqr5*sin(q5))/32 - (3*dq2*dqr4*sin(2*q4))/64 + (3*dq3*dqr4*sin(2*q4))/64 - (9*dq2*dqr5*sin(2*q5))/64 + (9*dq3*dqr5*sin(2*q5))/64 - (3*dq2*dqr4*cos(2*q4)*sin(q5))/8 - (3*dq2*dqr4*sin(2*q4)*cos(q5))/16 - (3*dq2*dqr5*cos(2*q4)*sin(q5))/32 - (3*dq2*dqr5*sin(2*q4)*cos(q5))/16 + (3*dq3*dqr4*cos(2*q4)*sin(q5))/8 + (3*dq3*dqr4*sin(2*q4)*cos(q5))/16 + (3*dq3*dqr5*cos(2*q4)*sin(q5))/32 + (3*dq3*dqr5*sin(2*q4)*cos(q5))/16 - (3^(1/2)*dq4*dqr4*sin(q4))/32 - (3*3^(1/2)*dq4*dqr5*sin(q4))/16 - (3*3^(1/2)*dq5*dqr4*sin(q4))/16 + (3*dq2*dqr4*cos(2*q4)*sin(2*q5))/16 + (15*dq2*dqr4*cos(2*q5)*sin(2*q4))/64 + (15*dq2*dqr5*cos(2*q4)*sin(2*q5))/64 + (3*dq2*dqr5*cos(2*q5)*sin(2*q4))/16 - (3*dq3*dqr4*cos(2*q4)*sin(2*q5))/16 - (15*dq3*dqr4*cos(2*q5)*sin(2*q4))/64 - (15*dq3*dqr5*cos(2*q4)*sin(2*q5))/64 - (3*dq3*dqr5*cos(2*q5)*sin(2*q4))/16 - (3*ddqr1*sin(2*q4)*cos(q2)*sin(q3))/64 + (3*ddqr1*sin(2*q4)*cos(q3)*sin(q2))/64 - (21*dq1*dqr4*cos(q2)*sin(q3))/64 + (21*dq1*dqr4*cos(q3)*sin(q2))/64 - (3*dq1*dqr5*cos(q2)*sin(q3))/16 + (3*dq1*dqr5*cos(q3)*sin(q2))/16 - (3^(1/2)*ddqr4*sin(q4)*sin(q5))/8 - (3*dq1*dqr4*cos(2*q4)*cos(q2)*sin(q3))/64 + (3*dq1*dqr4*cos(2*q4)*cos(q3)*sin(q2))/64 + (9*dq1*dqr4*cos(2*q5)*cos(q2)*sin(q3))/64 - (9*dq1*dqr4*cos(2*q5)*cos(q3)*sin(q2))/64 - (3^(1/2)*dq4*dqr4*cos(q4)*sin(q5))/8 + (3^(1/2)*dq4*dqr4*cos(q5)*sin(q4))/8 - (3^(1/2)*dq4*dqr5*cos(q4)*sin(q5))/16 - (3^(1/2)*dq4*dqr5*cos(q5)*sin(q4))/8 - (3^(1/2)*dq5*dqr4*cos(q4)*sin(q5))/16 - (3^(1/2)*dq5*dqr4*cos(q5)*sin(q4))/8 - (3^(1/2)*dq5*dqr5*cos(q4)*sin(q5))/8 - (3^(1/2)*dq5*dqr5*cos(q5)*sin(q4))/4 - (3*ddqr1*cos(2*q4)*cos(q2)*sin(q3)*sin(q5))/8 + (3*ddqr1*cos(2*q4)*cos(q3)*sin(q2)*sin(q5))/8 - (3*ddqr1*sin(2*q4)*cos(q2)*cos(q5)*sin(q3))/16 + (3*ddqr1*sin(2*q4)*cos(q3)*cos(q5)*sin(q2))/16 - (3*3^(1/2)*dq4*dqr4*cos(2*q5)*sin(q4))/32 - (3*3^(1/2)*dq4*dqr4*sin(2*q5)*cos(q4))/16 - (3*3^(1/2)*dq4*dqr5*cos(2*q5)*sin(q4))/16 - (3*3^(1/2)*dq4*dqr5*sin(2*q5)*cos(q4))/32 - (3*3^(1/2)*dq5*dqr4*cos(2*q5)*sin(q4))/16 - (3*3^(1/2)*dq5*dqr4*sin(2*q5)*cos(q4))/32 + (3*dq1*dqr4*cos(q2)*cos(q5)*sin(q3))/16 - (3*dq1*dqr4*cos(q3)*cos(q5)*sin(q2))/16 + (3*dq1*dqr5*cos(q2)*cos(q5)*sin(q3))/16 - (3*dq1*dqr5*cos(q3)*cos(q5)*sin(q2))/16 + (3^(1/2)*ddqr1*cos(q4)*sin(q2)*sin(q3))/32 + (3*ddqr1*cos(2*q4)*sin(2*q5)*cos(q2)*sin(q3))/16 - (3*ddqr1*cos(2*q4)*sin(2*q5)*cos(q3)*sin(q2))/16 + (15*ddqr1*cos(2*q5)*sin(2*q4)*cos(q2)*sin(q3))/64 - (15*ddqr1*cos(2*q5)*sin(2*q4)*cos(q3)*sin(q2))/64 + (3*dq1*dqr4*sin(2*q4)*cos(q2)*sin(q3)*sin(q5))/8 - (3*dq1*dqr4*sin(2*q4)*cos(q3)*sin(q2)*sin(q5))/8 + (3*dq1*dqr5*sin(2*q4)*cos(q2)*sin(q3)*sin(q5))/32 - (3*dq1*dqr5*sin(2*q4)*cos(q3)*sin(q2)*sin(q5))/32 - (3*3^(1/2)*ddqr1*sin(2*q5)*sin(q2)*sin(q3)*sin(q4))/16 - (3^(1/2)*dq1*dqr4*cos(q2)*cos(q3)*sin(q4))/32 - (3*3^(1/2)*dq1*dqr5*cos(q2)*cos(q3)*sin(q4))/16 - (3*3^(1/2)*dq1*dqr5*sin(q2)*sin(q3)*sin(q4))/16 + (15*dq1*dqr4*cos(2*q4)*cos(2*q5)*cos(q2)*sin(q3))/64 - (15*dq1*dqr4*cos(2*q4)*cos(2*q5)*cos(q3)*sin(q2))/64 + (3*dq1*dqr5*cos(2*q4)*cos(2*q5)*cos(q2)*sin(q3))/16 - (3*dq1*dqr5*cos(2*q4)*cos(2*q5)*cos(q3)*sin(q2))/16 - (3*dq1*dqr4*sin(2*q4)*sin(2*q5)*cos(q2)*sin(q3))/16 + (3*dq1*dqr4*sin(2*q4)*sin(2*q5)*cos(q3)*sin(q2))/16 - (15*dq1*dqr5*sin(2*q4)*sin(2*q5)*cos(q2)*sin(q3))/64 + (15*dq1*dqr5*sin(2*q4)*sin(2*q5)*cos(q3)*sin(q2))/64 - (3^(1/2)*ddqr1*cos(q2)*cos(q3)*sin(q4)*sin(q5))/8 - (3^(1/2)*ddqr1*cos(q4)*cos(q5)*sin(q2)*sin(q3))/8 - (3^(1/2)*ddqr1*sin(q2)*sin(q3)*sin(q4)*sin(q5))/8 - (3*dq1*dqr4*cos(2*q4)*cos(q2)*cos(q5)*sin(q3))/16 + (3*dq1*dqr4*cos(2*q4)*cos(q3)*cos(q5)*sin(q2))/16 - (3*dq1*dqr5*cos(2*q4)*cos(q2)*cos(q5)*sin(q3))/16 + (3*dq1*dqr5*cos(2*q4)*cos(q3)*cos(q5)*sin(q2))/16 + (3*3^(1/2)*ddqr1*cos(2*q5)*cos(q4)*sin(q2)*sin(q3))/32 - (3^(1/2)*dq1*dqr5*cos(q4)*sin(q2)*sin(q3)*sin(q5))/16 - (3^(1/2)*dq1*dqr5*cos(q5)*sin(q2)*sin(q3)*sin(q4))/8 - (3*3^(1/2)*dq1*dqr4*cos(2*q5)*cos(q2)*cos(q3)*sin(q4))/32 - (3*3^(1/2)*dq1*dqr4*sin(2*q5)*cos(q2)*cos(q3)*cos(q4))/16 - (3*3^(1/2)*dq1*dqr5*cos(2*q5)*cos(q2)*cos(q3)*sin(q4))/16 - (3*3^(1/2)*dq1*dqr5*sin(2*q5)*cos(q2)*cos(q3)*cos(q4))/32 - (3*3^(1/2)*dq1*dqr4*sin(2*q5)*cos(q4)*sin(q2)*sin(q3))/16 - (3*3^(1/2)*dq1*dqr5*cos(2*q5)*sin(q2)*sin(q3)*sin(q4))/16 - (3*3^(1/2)*dq1*dqr5*sin(2*q5)*cos(q4)*sin(q2)*sin(q3))/32 - (3^(1/2)*dq1*dqr4*cos(q2)*cos(q3)*cos(q4)*sin(q5))/8 + (3^(1/2)*dq1*dqr4*cos(q2)*cos(q3)*cos(q5)*sin(q4))/8 - (3^(1/2)*dq1*dqr5*cos(q2)*cos(q3)*cos(q4)*sin(q5))/16 - (3^(1/2)*dq1*dqr5*cos(q2)*cos(q3)*cos(q5)*sin(q4))/8;
Y2_19_3=(43*ddqr2)/64 - (43*ddqr3)/64 + (3*ddqr2*cos(q5))/16 - (3*ddqr3*cos(q5))/16 + (3*ddqr2*cos(2*q4))/64 + (9*ddqr2*cos(2*q5))/64 - (3*ddqr3*cos(2*q4))/64 - (9*ddqr3*cos(2*q5))/64 - (15*ddqr2*cos(2*q4)*cos(2*q5))/64 + (15*ddqr3*cos(2*q4)*cos(2*q5))/64 + (3*ddqr2*sin(2*q4)*sin(2*q5))/16 - (3*ddqr3*sin(2*q4)*sin(2*q5))/16 + (3*ddqr2*cos(2*q4)*cos(q5))/16 - (3*ddqr3*cos(2*q4)*cos(q5))/16 - (3*ddqr2*sin(2*q4)*sin(q5))/8 + (3*ddqr3*sin(2*q4)*sin(q5))/8 + (3^(1/2)*ddqr4*cos(q4))/32 + (3*3^(1/2)*ddqr5*cos(q4))/8 + (3*3^(1/2)*ddqr4*cos(2*q5)*cos(q4))/32 - (3*3^(1/2)*ddqr4*sin(2*q5)*sin(q4))/16 - (3^(1/2)*ddqr4*cos(q4)*cos(q5))/8 + (3^(1/2)*ddqr5*cos(q4)*cos(q5))/8 - (3^(1/2)*ddqr5*sin(q4)*sin(q5))/4 + (3^(1/2)*ddqr1*cos(q2)*cos(q3)*cos(q4))/32 - (3^(1/2)*ddqr1*cos(q2)*cos(q3)*cos(q4)*cos(q5))/8 + (3*3^(1/2)*ddqr1*cos(2*q5)*cos(q2)*cos(q3)*cos(q4))/32 - (3*3^(1/2)*ddqr1*sin(2*q5)*cos(q2)*cos(q3)*sin(q4))/16;
Y2_20_1=-sin(q2);
Y2_21_1=-sin(q2 - q3);
Y2_22_1=sin(q2 - q3);
Y2_23_1=sin(q2 - q3)/2 - (3^(1/2)*sin(q2 - q3 + q4))/4 - (3^(1/2)*sin(q3 - q2 + q4))/4;
Y2_24_1=sin(q2 - q3)/4 + (3*sin(q2 - q3 + q5))/8 - (3*sin(q3 - q2 + q5))/8 - (3^(1/2)*sin(q2 - q3 + q4 - q5))/16 + (3^(1/2)*sin(q2 - q3 - q4 + q5))/16 - (3^(1/2)*sin(q2 - q3 + q4))/8 - (3^(1/2)*sin(q3 - q2 + q4))/8 + (3*3^(1/2)*sin(q2 - q3 + q4 + q5))/16 + (3*3^(1/2)*sin(q3 - q2 + q4 + q5))/16;
Y3_3_1=(1515361*ddqr3)/100000000 - (1515361*ddqr2)/100000000 + (35699*ddqr2*cos(q3))/1000000 - (8617*ddqr1*cos(q2 - q3))/10000000 - (35699*dq1*dqr1*sin(q3))/2000000 - (35699*dq2*dqr2*sin(q3))/1000000 + (35699*dq1*dqr1*cos(2*q2)*sin(q3))/2000000 - (35699*dq1*dqr1*sin(2*q2)*cos(q3))/2000000 - (1515361*dq1*dqr1*cos(2*q2)*sin(2*q3))/200000000 + (1515361*dq1*dqr1*cos(2*q3)*sin(2*q2))/200000000;
Y3_4_1=(1786417*ddqr3)/50000000 - (1786417*ddqr2)/50000000 + (35927*ddqr1*cos(q2 - q3 + q4))/10000000 + (33337*ddqr1*cos(q3 - q2 + q4))/10000000 + (1073*ddqr2*cos(q3 + q4))/200000 + (3393*ddqr2*cos(q3))/62500 + (4329*ddqr4*cos(q4))/625000 - (1369*ddqr1*cos(q2 - q3 + 2*q4))/4000000 + (1369*ddqr1*cos(q3 - q2 + 2*q4))/4000000 - (819*ddqr1*cos(q2 - q3))/625000 - (1073*ddqr2*cos(q3 - q4))/200000 + (1369*ddqr2*cos(2*q4))/2000000 - (1369*ddqr3*cos(2*q4))/2000000 - (3393*dq1*dqr1*sin(q3))/125000 - (3393*dq2*dqr2*sin(q3))/62500 - (4329*dq4*dqr4*sin(q4))/625000 - (1369*dq2*dqr4*sin(2*q4))/2000000 - (1369*dq4*dqr2*sin(2*q4))/2000000 + (1369*dq3*dqr4*sin(2*q4))/2000000 + (1369*dq4*dqr3*sin(2*q4))/2000000 + (3393*dq1*dqr1*cos(2*q2)*sin(q3))/125000 - (3393*dq1*dqr1*sin(2*q2)*cos(q3))/125000 - (1717967*dq1*dqr1*cos(2*q2)*sin(2*q3))/100000000 + (1717967*dq1*dqr1*cos(2*q3)*sin(2*q2))/100000000 - (1073*dq1*dqr1*cos(q3)*sin(q4))/200000 + (1369*dq1*dqr4*cos(q2)*sin(q3))/2000000 - (1369*dq1*dqr4*cos(q3)*sin(q2))/2000000 + (1369*dq4*dqr1*cos(q2)*sin(q3))/2000000 - (1369*dq4*dqr1*cos(q3)*sin(q2))/2000000 - (1073*dq2*dqr2*cos(q3)*sin(q4))/100000 + (1073*dq1*dqr1*cos(2*q2)*cos(q3)*sin(q4))/200000 - (1369*dq1*dqr4*cos(2*q4)*cos(q2)*sin(q3))/2000000 + (1369*dq1*dqr4*cos(2*q4)*cos(q3)*sin(q2))/2000000 - (1369*dq4*dqr1*cos(2*q4)*cos(q2)*sin(q3))/2000000 + (1369*dq4*dqr1*cos(2*q4)*cos(q3)*sin(q2))/2000000 + (1073*dq1*dqr1*sin(2*q2)*sin(q3)*sin(q4))/200000 - (4329*dq1*dqr1*cos(2*q2)*cos(2*q3)*sin(q4))/625000 - (4329*dq1*dqr1*sin(2*q2)*sin(2*q3)*sin(q4))/625000 - (4329*dq1*dqr4*cos(q2)*cos(q3)*sin(q4))/625000 - (4329*dq4*dqr1*cos(q2)*cos(q3)*sin(q4))/625000 - (1369*dq1*dqr1*cos(2*q2)*cos(2*q4)*sin(2*q3))/4000000 + (1369*dq1*dqr1*cos(2*q3)*cos(2*q4)*sin(2*q2))/4000000 - (4329*dq1*dqr4*sin(q2)*sin(q3)*sin(q4))/625000 - (4329*dq4*dqr1*sin(q2)*sin(q3)*sin(q4))/625000;
Y3_5_1=dq5*dqr2*sin(q5)*((300773*3^(1/2))/80000000 - 1369/4000000) - (25433*dq2*dqr2*sin(q3))/400000 - (25433*dq1*dqr1*sin(q3))/800000 + (25433*dq1*dqr1*cos(2*q2)*sin(q3))/800000 - (25433*dq1*dqr1*sin(2*q2)*cos(q3))/800000 - (1369*dq4*dqr2*cos(2*q5)*sin(2*q4))/3200000 + (1369*dq5*dqr1*cos(q2)*sin(q3))/4000000 - (1369*dq5*dqr1*cos(q3)*sin(q2))/4000000 - (4107*dq4*dqr1*cos(2*q5)*cos(q2)*sin(q3))/16000000 + (4107*dq4*dqr1*cos(2*q5)*cos(q3)*sin(q2))/16000000 + dq1*dqr1*cos(2*q2)*sin(2*q3)*((23717*3^(1/2))/40000000 - 36744657/1600000000) - dq1*dqr1*cos(2*q3)*sin(2*q2)*((23717*3^(1/2))/40000000 - 36744657/1600000000) + dq4*dqr1*cos(q2)*sin(q3)*((23717*3^(1/2))/20000000 + 2122493/800000000) - dq4*dqr1*cos(q3)*sin(q2)*((23717*3^(1/2))/20000000 + 2122493/800000000) - (1073*3^(1/2)*dq1*dqr1*cos(q5)*sin(q3))/400000 - (1073*3^(1/2)*dq2*dqr2*cos(q5)*sin(q3))/200000 + dq4*dqr2*cos(2*q4)*sin(q5)*((23717*3^(1/2))/20000000 + 1369/1000000) + dq4*dqr2*sin(2*q4)*cos(q5)*((23717*3^(1/2))/40000000 + 1369/2000000) + dq5*dqr2*sin(2*q4)*cos(q5)*((23717*3^(1/2))/40000000 + 1369/2000000) + dq5*dqr2*cos(2*q4)*sin(q5)*((23717*3^(1/2))/80000000 + 1369/4000000) + (1073*dq1*dqr1*cos(q3)*cos(q4)*sin(q5))/200000 + (1073*dq1*dqr1*cos(q3)*cos(q5)*sin(q4))/400000 + (1073*dq2*dqr2*cos(q3)*cos(q4)*sin(q5))/100000 + (1073*dq2*dqr2*cos(q3)*cos(q5)*sin(q4))/200000 - (12321*dq1*dqr1*cos(2*q2)*cos(2*q5)*sin(2*q3))/32000000 + (12321*dq1*dqr1*cos(2*q3)*cos(2*q5)*sin(2*q2))/32000000 - dq2*dqr2*cos(q3)*sin(q4)*((18589*3^(1/2))/2000000 + 1073/100000) - dq1*dqr1*cos(q3)*sin(q4)*((18589*3^(1/2))/4000000 + 1073/200000) - (1369*dq1*dqr1*cos(2*q2)*cos(2*q4)*cos(2*q5)*sin(2*q3))/6400000 + (1369*dq1*dqr1*cos(2*q3)*cos(2*q4)*cos(2*q5)*sin(2*q2))/6400000 - (1073*dq1*dqr1*sin(2*q2)*cos(q4)*sin(q3)*sin(q5))/200000 - (1073*dq1*dqr1*sin(2*q2)*cos(q5)*sin(q3)*sin(q4))/400000 + (1369*3^(1/2)*dq5*dqr1*cos(q2)*cos(q3)*sin(q4))/4000000 + (1369*dq1*dqr1*cos(2*q2)*sin(2*q3)*sin(2*q4)*sin(2*q5))/8000000 - (1369*dq1*dqr1*cos(2*q3)*sin(2*q2)*sin(2*q4)*sin(2*q5))/8000000 + dq1*dqr1*cos(2*q2)*cos(q3)*sin(q4)*((18589*3^(1/2))/4000000 + 1073/200000) + (1369*3^(1/2)*dq5*dqr1*sin(q2)*sin(q3)*sin(q4))/4000000 + (32449*dq1*dqr1*cos(2*q2)*cos(2*q3)*cos(q4)*sin(q5))/4000000 - (1369*dq4*dqr1*cos(2*q4)*cos(2*q5)*cos(q2)*sin(q3))/3200000 + (1369*dq4*dqr1*cos(2*q4)*cos(2*q5)*cos(q3)*sin(q2))/3200000 - (1369*dq5*dqr1*cos(2*q4)*cos(2*q5)*cos(q2)*sin(q3))/4000000 + (1369*dq5*dqr1*cos(2*q4)*cos(2*q5)*cos(q3)*sin(q2))/4000000 + dq1*dqr1*sin(2*q2)*sin(q3)*sin(q4)*((18589*3^(1/2))/4000000 + 1073/200000) - dq1*dqr1*cos(2*q2)*cos(2*q4)*sin(2*q3)*((23717*3^(1/2))/40000000 + 1574893/1600000000) + dq1*dqr1*cos(2*q3)*cos(2*q4)*sin(2*q2)*((23717*3^(1/2))/40000000 + 1574893/1600000000) - dq4*dqr1*cos(2*q4)*cos(q2)*sin(q3)*((23717*3^(1/2))/20000000 + 1574893/800000000) + dq4*dqr1*cos(2*q4)*cos(q3)*sin(q2)*((23717*3^(1/2))/20000000 + 1574893/800000000) + (32449*dq1*dqr1*sin(2*q2)*sin(2*q3)*cos(q4)*sin(q5))/4000000 + (1369*dq4*dqr1*sin(2*q4)*sin(2*q5)*cos(q2)*sin(q3))/4000000 - (1369*dq4*dqr1*sin(2*q4)*sin(2*q5)*cos(q3)*sin(q2))/4000000 + (1369*dq5*dqr1*sin(2*q4)*sin(2*q5)*cos(q2)*sin(q3))/3200000 - (1369*dq5*dqr1*sin(2*q4)*sin(2*q5)*cos(q3)*sin(q2))/3200000 + (1073*3^(1/2)*dq1*dqr1*cos(2*q2)*cos(q5)*sin(q3))/400000 - (1073*3^(1/2)*dq1*dqr1*sin(2*q2)*cos(q3)*cos(q5))/400000 + (32449*dq4*dqr1*cos(q2)*cos(q3)*cos(q4)*sin(q5))/4000000 + (32449*dq5*dqr1*cos(q2)*cos(q3)*cos(q4)*sin(q5))/8000000 + (32449*dq5*dqr1*cos(q2)*cos(q3)*cos(q5)*sin(q4))/4000000 - dq1*dqr1*cos(2*q2)*sin(2*q3)*cos(q5)*((348207*3^(1/2))/80000000 + 1369/4000000) + dq1*dqr1*cos(2*q3)*sin(2*q2)*cos(q5)*((348207*3^(1/2))/80000000 + 1369/4000000) - dq1*dqr1*cos(2*q2)*cos(2*q3)*sin(q4)*((548467*3^(1/2))/80000000 + 32449/4000000) + (32449*dq4*dqr1*cos(q4)*sin(q2)*sin(q3)*sin(q5))/4000000 + (32449*dq5*dqr1*cos(q4)*sin(q2)*sin(q3)*sin(q5))/8000000 + (32449*dq5*dqr1*cos(q5)*sin(q2)*sin(q3)*sin(q4))/4000000 - dq1*dqr1*sin(2*q2)*sin(2*q3)*sin(q4)*((548467*3^(1/2))/80000000 + 32449/4000000) - dq4*dqr1*cos(q2)*cos(q5)*sin(q3)*((23717*3^(1/2))/40000000 + 1369/2000000) + dq4*dqr1*cos(q3)*cos(q5)*sin(q2)*((23717*3^(1/2))/40000000 + 1369/2000000) - dq5*dqr1*cos(q2)*cos(q5)*sin(q3)*((23717*3^(1/2))/40000000 + 1369/2000000) + dq5*dqr1*cos(q3)*cos(q5)*sin(q2)*((23717*3^(1/2))/40000000 + 1369/2000000) - dq4*dqr1*cos(q2)*cos(q3)*sin(q4)*((548467*3^(1/2))/80000000 + 32449/4000000) - (1073*dq1*dqr1*cos(2*q2)*cos(q3)*cos(q4)*sin(q5))/200000 - (1073*dq1*dqr1*cos(2*q2)*cos(q3)*cos(q5)*sin(q4))/400000 - dq4*dqr1*sin(q2)*sin(q3)*sin(q4)*((548467*3^(1/2))/80000000 + 32449/4000000) + (1369*3^(1/2)*dq1*dqr1*cos(2*q2)*cos(2*q3)*cos(2*q5)*sin(q4))/8000000 + (1369*3^(1/2)*dq1*dqr1*cos(2*q2)*cos(2*q3)*sin(2*q5)*cos(q4))/4000000 + dq4*dqr1*cos(2*q4)*cos(q2)*cos(q5)*sin(q3)*((23717*3^(1/2))/40000000 + 1369/2000000) - dq4*dqr1*cos(2*q4)*cos(q3)*cos(q5)*sin(q2)*((23717*3^(1/2))/40000000 + 1369/2000000) + dq5*dqr1*cos(2*q4)*cos(q2)*cos(q5)*sin(q3)*((23717*3^(1/2))/40000000 + 1369/2000000) - dq5*dqr1*cos(2*q4)*cos(q3)*cos(q5)*sin(q2)*((23717*3^(1/2))/40000000 + 1369/2000000) + (1369*3^(1/2)*dq1*dqr1*cos(2*q5)*sin(2*q2)*sin(2*q3)*sin(q4))/8000000 + (1369*3^(1/2)*dq1*dqr1*sin(2*q2)*sin(2*q3)*sin(2*q5)*cos(q4))/4000000 - dq4*dqr1*sin(2*q4)*cos(q2)*sin(q3)*sin(q5)*((23717*3^(1/2))/20000000 + 1369/1000000) + dq4*dqr1*sin(2*q4)*cos(q3)*sin(q2)*sin(q5)*((23717*3^(1/2))/20000000 + 1369/1000000) - dq5*dqr1*sin(2*q4)*cos(q2)*sin(q3)*sin(q5)*((23717*3^(1/2))/80000000 + 1369/4000000) + dq5*dqr1*sin(2*q4)*cos(q3)*sin(q2)*sin(q5)*((23717*3^(1/2))/80000000 + 1369/4000000) + (1369*3^(1/2)*dq4*dqr1*cos(2*q5)*cos(q2)*cos(q3)*sin(q4))/8000000 + (1369*3^(1/2)*dq4*dqr1*sin(2*q5)*cos(q2)*cos(q3)*cos(q4))/4000000 + (1369*3^(1/2)*dq5*dqr1*cos(2*q5)*cos(q2)*cos(q3)*sin(q4))/4000000 + (1369*3^(1/2)*dq5*dqr1*sin(2*q5)*cos(q2)*cos(q3)*cos(q4))/8000000 - dq1*dqr1*cos(2*q2)*cos(2*q3)*cos(q5)*sin(q4)*((1369*3^(1/2))/2000000 - 45547/20000000) + (1369*3^(1/2)*dq4*dqr1*cos(2*q5)*sin(q2)*sin(q3)*sin(q4))/8000000 + (1369*3^(1/2)*dq4*dqr1*sin(2*q5)*cos(q4)*sin(q2)*sin(q3))/4000000 + (1369*3^(1/2)*dq5*dqr1*cos(2*q5)*sin(q2)*sin(q3)*sin(q4))/4000000 + (1369*3^(1/2)*dq5*dqr1*sin(2*q5)*cos(q4)*sin(q2)*sin(q3))/8000000 - dq1*dqr1*sin(2*q2)*sin(2*q3)*cos(q5)*sin(q4)*((1369*3^(1/2))/2000000 - 45547/20000000) - dq4*dqr1*cos(q2)*cos(q3)*cos(q5)*sin(q4)*((1369*3^(1/2))/2000000 - 45547/20000000) - dq4*dqr1*cos(q5)*sin(q2)*sin(q3)*sin(q4)*((1369*3^(1/2))/2000000 - 45547/20000000) + dq1*dqr1*cos(2*q2)*cos(2*q4)*sin(2*q3)*cos(q5)*((23717*3^(1/2))/80000000 + 1369/4000000) - dq1*dqr1*cos(2*q3)*cos(2*q4)*sin(2*q2)*cos(q5)*((23717*3^(1/2))/80000000 + 1369/4000000) - dq1*dqr1*cos(2*q2)*sin(2*q3)*sin(2*q4)*sin(q5)*((23717*3^(1/2))/40000000 + 1369/2000000) + dq1*dqr1*cos(2*q3)*sin(2*q2)*sin(2*q4)*sin(q5)*((23717*3^(1/2))/40000000 + 1369/2000000);
Y3_5_2=(4107*dq2*dqr5*sin(2*q5))/16000000 + (4107*dq5*dqr2*sin(2*q5))/16000000 - (4107*dq5*dqr3*sin(2*q5))/16000000 + dq2*dqr5*sin(q5)*((300773*3^(1/2))/80000000 - 1369/4000000) - dq3*dqr5*sin(q5)*((300773*3^(1/2))/80000000 - 1369/4000000) - dq5*dqr3*sin(q5)*((300773*3^(1/2))/80000000 - 1369/4000000) - dq4*dqr4*sin(q4)*((548467*3^(1/2))/80000000 + 32449/4000000) + (1369*3^(1/2)*dq4*dqr5*sin(q4))/4000000 + (1369*3^(1/2)*dq5*dqr4*sin(q4))/4000000 - (1369*dq2*dqr4*cos(2*q4)*sin(2*q5))/4000000 - (1369*dq2*dqr4*cos(2*q5)*sin(2*q4))/3200000 - (1369*dq4*dqr2*cos(2*q4)*sin(2*q5))/4000000 - (1369*dq2*dqr5*cos(2*q4)*sin(2*q5))/3200000 - (1369*dq2*dqr5*cos(2*q5)*sin(2*q4))/4000000 + (1369*dq3*dqr4*cos(2*q4)*sin(2*q5))/4000000 + (1369*dq3*dqr4*cos(2*q5)*sin(2*q4))/3200000 + (1369*dq4*dqr3*cos(2*q4)*sin(2*q5))/4000000 + (1369*dq4*dqr3*cos(2*q5)*sin(2*q4))/3200000 - (1369*dq5*dqr2*cos(2*q4)*sin(2*q5))/3200000 - (1369*dq5*dqr2*cos(2*q5)*sin(2*q4))/4000000 + (1369*dq5*dqr3*cos(2*q4)*sin(2*q5))/3200000 + (1369*dq5*dqr3*cos(2*q5)*sin(2*q4))/4000000 - dq2*dqr4*sin(2*q4)*((23717*3^(1/2))/20000000 + 1574893/800000000) - dq4*dqr2*sin(2*q4)*((23717*3^(1/2))/20000000 + 1574893/800000000) + dq3*dqr4*sin(2*q4)*((23717*3^(1/2))/20000000 + 1574893/800000000) + dq4*dqr3*sin(2*q4)*((23717*3^(1/2))/20000000 + 1574893/800000000) + (1369*dq1*dqr5*cos(q2)*sin(q3))/4000000 - (1369*dq1*dqr5*cos(q3)*sin(q2))/4000000 + (32449*dq4*dqr4*cos(q4)*sin(q5))/4000000 + (32449*dq4*dqr5*cos(q4)*sin(q5))/8000000 + (32449*dq4*dqr5*cos(q5)*sin(q4))/4000000 + (32449*dq5*dqr4*cos(q4)*sin(q5))/8000000 + (32449*dq5*dqr4*cos(q5)*sin(q4))/4000000 + (32449*dq5*dqr5*cos(q4)*sin(q5))/4000000 + dq5*dqr5*cos(q5)*sin(q4)*((1369*3^(1/2))/2000000 + 58349/10000000) - dq4*dqr4*cos(q5)*sin(q4)*((1369*3^(1/2))/2000000 - 45547/20000000) - (4107*dq1*dqr4*cos(2*q5)*cos(q2)*sin(q3))/16000000 + (4107*dq1*dqr4*cos(2*q5)*cos(q3)*sin(q2))/16000000 + dq1*dqr4*cos(q2)*sin(q3)*((23717*3^(1/2))/20000000 + 2122493/800000000) - dq1*dqr4*cos(q3)*sin(q2)*((23717*3^(1/2))/20000000 + 2122493/800000000) + dq2*dqr4*cos(2*q4)*sin(q5)*((23717*3^(1/2))/20000000 + 1369/1000000) - dq3*dqr4*cos(2*q4)*sin(q5)*((23717*3^(1/2))/20000000 + 1369/1000000) - dq4*dqr3*cos(2*q4)*sin(q5)*((23717*3^(1/2))/20000000 + 1369/1000000) + dq2*dqr4*sin(2*q4)*cos(q5)*((23717*3^(1/2))/40000000 + 1369/2000000) + dq2*dqr5*sin(2*q4)*cos(q5)*((23717*3^(1/2))/40000000 + 1369/2000000) - dq3*dqr4*sin(2*q4)*cos(q5)*((23717*3^(1/2))/40000000 + 1369/2000000) - dq4*dqr3*sin(2*q4)*cos(q5)*((23717*3^(1/2))/40000000 + 1369/2000000) - dq3*dqr5*sin(2*q4)*cos(q5)*((23717*3^(1/2))/40000000 + 1369/2000000) - dq5*dqr3*sin(2*q4)*cos(q5)*((23717*3^(1/2))/40000000 + 1369/2000000) + dq2*dqr5*cos(2*q4)*sin(q5)*((23717*3^(1/2))/80000000 + 1369/4000000) - dq3*dqr5*cos(2*q4)*sin(q5)*((23717*3^(1/2))/80000000 + 1369/4000000) - dq5*dqr3*cos(2*q4)*sin(q5)*((23717*3^(1/2))/80000000 + 1369/4000000) + (1369*3^(1/2)*dq4*dqr4*cos(2*q5)*sin(q4))/8000000 + (1369*3^(1/2)*dq4*dqr4*sin(2*q5)*cos(q4))/4000000 + (1369*3^(1/2)*dq4*dqr5*cos(2*q5)*sin(q4))/4000000 + (1369*3^(1/2)*dq4*dqr5*sin(2*q5)*cos(q4))/8000000 + (1369*3^(1/2)*dq5*dqr4*cos(2*q5)*sin(q4))/4000000 + (1369*3^(1/2)*dq5*dqr4*sin(2*q5)*cos(q4))/8000000 + (1369*3^(1/2)*dq1*dqr5*cos(q2)*cos(q3)*sin(q4))/4000000 + (1369*3^(1/2)*dq1*dqr5*sin(q2)*sin(q3)*sin(q4))/4000000 - (1369*dq1*dqr4*cos(2*q4)*cos(2*q5)*cos(q2)*sin(q3))/3200000 + (1369*dq1*dqr4*cos(2*q4)*cos(2*q5)*cos(q3)*sin(q2))/3200000 - (1369*dq1*dqr5*cos(2*q4)*cos(2*q5)*cos(q2)*sin(q3))/4000000 + (1369*dq1*dqr5*cos(2*q4)*cos(2*q5)*cos(q3)*sin(q2))/4000000 - dq1*dqr4*cos(2*q4)*cos(q2)*sin(q3)*((23717*3^(1/2))/20000000 + 1574893/800000000) + dq1*dqr4*cos(2*q4)*cos(q3)*sin(q2)*((23717*3^(1/2))/20000000 + 1574893/800000000) + (1369*dq1*dqr4*sin(2*q4)*sin(2*q5)*cos(q2)*sin(q3))/4000000 - (1369*dq1*dqr4*sin(2*q4)*sin(2*q5)*cos(q3)*sin(q2))/4000000 + (1369*dq1*dqr5*sin(2*q4)*sin(2*q5)*cos(q2)*sin(q3))/3200000 - (1369*dq1*dqr5*sin(2*q4)*sin(2*q5)*cos(q3)*sin(q2))/3200000 + (32449*dq1*dqr4*cos(q2)*cos(q3)*cos(q4)*sin(q5))/4000000 + (32449*dq1*dqr5*cos(q2)*cos(q3)*cos(q4)*sin(q5))/8000000 + (32449*dq1*dqr5*cos(q2)*cos(q3)*cos(q5)*sin(q4))/4000000 + (32449*dq1*dqr4*cos(q4)*sin(q2)*sin(q3)*sin(q5))/4000000 + (32449*dq1*dqr5*cos(q4)*sin(q2)*sin(q3)*sin(q5))/8000000 + (32449*dq1*dqr5*cos(q5)*sin(q2)*sin(q3)*sin(q4))/4000000 - dq1*dqr4*cos(q2)*cos(q5)*sin(q3)*((23717*3^(1/2))/40000000 + 1369/2000000) + dq1*dqr4*cos(q3)*cos(q5)*sin(q2)*((23717*3^(1/2))/40000000 + 1369/2000000) - dq1*dqr5*cos(q2)*cos(q5)*sin(q3)*((23717*3^(1/2))/40000000 + 1369/2000000) + dq1*dqr5*cos(q3)*cos(q5)*sin(q2)*((23717*3^(1/2))/40000000 + 1369/2000000) - dq1*dqr4*cos(q2)*cos(q3)*sin(q4)*((548467*3^(1/2))/80000000 + 32449/4000000) - dq1*dqr4*sin(q2)*sin(q3)*sin(q4)*((548467*3^(1/2))/80000000 + 32449/4000000) + dq1*dqr4*cos(2*q4)*cos(q2)*cos(q5)*sin(q3)*((23717*3^(1/2))/40000000 + 1369/2000000) - dq1*dqr4*cos(2*q4)*cos(q3)*cos(q5)*sin(q2)*((23717*3^(1/2))/40000000 + 1369/2000000) + dq1*dqr5*cos(2*q4)*cos(q2)*cos(q5)*sin(q3)*((23717*3^(1/2))/40000000 + 1369/2000000) - dq1*dqr5*cos(2*q4)*cos(q3)*cos(q5)*sin(q2)*((23717*3^(1/2))/40000000 + 1369/2000000) - dq1*dqr4*sin(2*q4)*cos(q2)*sin(q3)*sin(q5)*((23717*3^(1/2))/20000000 + 1369/1000000) + dq1*dqr4*sin(2*q4)*cos(q3)*sin(q2)*sin(q5)*((23717*3^(1/2))/20000000 + 1369/1000000) - dq1*dqr5*sin(2*q4)*cos(q2)*sin(q3)*sin(q5)*((23717*3^(1/2))/80000000 + 1369/4000000) + dq1*dqr5*sin(2*q4)*cos(q3)*sin(q2)*sin(q5)*((23717*3^(1/2))/80000000 + 1369/4000000) + (1369*3^(1/2)*dq1*dqr4*cos(2*q5)*cos(q2)*cos(q3)*sin(q4))/8000000 + (1369*3^(1/2)*dq1*dqr4*sin(2*q5)*cos(q2)*cos(q3)*cos(q4))/4000000 + (1369*3^(1/2)*dq1*dqr5*cos(2*q5)*cos(q2)*cos(q3)*sin(q4))/4000000 + (1369*3^(1/2)*dq1*dqr5*sin(2*q5)*cos(q2)*cos(q3)*cos(q4))/8000000 + (1369*3^(1/2)*dq1*dqr4*cos(2*q5)*sin(q2)*sin(q3)*sin(q4))/8000000 + (1369*3^(1/2)*dq1*dqr4*sin(2*q5)*cos(q4)*sin(q2)*sin(q3))/4000000 + (1369*3^(1/2)*dq1*dqr5*cos(2*q5)*sin(q2)*sin(q3)*sin(q4))/4000000 + (1369*3^(1/2)*dq1*dqr5*sin(2*q5)*cos(q4)*sin(q2)*sin(q3))/8000000 - dq1*dqr4*cos(q2)*cos(q3)*cos(q5)*sin(q4)*((1369*3^(1/2))/2000000 - 45547/20000000) - dq1*dqr4*cos(q5)*sin(q2)*sin(q3)*sin(q4)*((1369*3^(1/2))/2000000 - 45547/20000000);
Y3_5_3=ddqr3*((23717*3^(1/2))/20000000 + 40989643/800000000) - ddqr2*((23717*3^(1/2))/20000000 + 40989643/800000000) + (1369*ddqr2*cos(2*q4 - 2*q5))/32000000 + (12321*ddqr2*cos(2*q4 + 2*q5))/32000000 - (1369*ddqr3*cos(2*q4 - 2*q5))/32000000 - (12321*ddqr3*cos(2*q4 + 2*q5))/32000000 + (1073*ddqr2*cos(q3 + q4 - q5))/800000 - (1073*ddqr2*cos(q3 - q4 + q5))/800000 + (3219*ddqr2*cos(q4 - q3 + q5))/800000 + (1369*ddqr1*cos(q2 - q3 - 2*q4 + 2*q5))/64000000 - (1369*ddqr1*cos(q2 - q3 + 2*q4 - 2*q5))/64000000 - (12321*ddqr1*cos(q2 - q3 + 2*q4 + 2*q5))/64000000 + (12321*ddqr1*cos(q3 - q2 + 2*q4 + 2*q5))/64000000 + (25433*ddqr2*cos(q3))/400000 - (6139*ddqr1*cos(q2 - q3))/4000000 - (3219*ddqr2*cos(q3 + q4 + q5))/800000 - (4107*ddqr2*cos(2*q5))/16000000 + (4107*ddqr3*cos(2*q5))/16000000 - ddqr1*cos(q2 - q3 + 2*q4)*((23717*3^(1/2))/40000000 + 1574893/1600000000) + ddqr1*cos(q3 - q2 + 2*q4)*((23717*3^(1/2))/40000000 + 1574893/1600000000) + (1073*3^(1/2)*ddqr2*cos(q3 - q5))/400000 + (1369*3^(1/2)*ddqr4*cos(q4 - 2*q5))/16000000 - (4107*3^(1/2)*ddqr4*cos(q4 + 2*q5))/16000000 + ddqr1*cos(q2 - q3 + q4 - q5)*((1369*3^(1/2))/8000000 + 14911/10000000) + ddqr1*cos(q2 - q3 - q4 + q5)*((1369*3^(1/2))/8000000 + 28527/20000000) + ddqr1*cos(q2 - q3 - 2*q4 + q5)*((23717*3^(1/2))/160000000 + 1369/8000000) + ddqr1*cos(q2 - q3 + 2*q4 + q5)*((71151*3^(1/2))/160000000 + 4107/8000000) - ddqr1*cos(q3 - q2 + 2*q4 + q5)*((71151*3^(1/2))/160000000 + 4107/8000000) + ddqr2*cos(2*q4)*((23717*3^(1/2))/20000000 + 1574893/800000000) - ddqr3*cos(2*q4)*((23717*3^(1/2))/20000000 + 1574893/800000000) + ddqr2*cos(2*q4 - q5)*((23717*3^(1/2))/80000000 + 1369/4000000) - ddqr3*cos(2*q4 - q5)*((23717*3^(1/2))/80000000 + 1369/4000000) + ddqr1*cos(q2 - q3 + q4)*((113283*3^(1/2))/32000000 + 6697/1600000) + ddqr1*cos(q3 - q2 + q4)*((530519*3^(1/2))/160000000 + 31413/8000000) + (1369*3^(1/2)*ddqr1*cos(q2 - q3 + q4 - 2*q5))/32000000 - (4107*3^(1/2)*ddqr1*cos(q2 - q3 + q4 + 2*q5))/32000000 - (4107*3^(1/2)*ddqr1*cos(q3 - q2 + q4 + 2*q5))/32000000 - (4107*dq3*dqr5*sin(2*q5))/16000000 + ddqr2*cos(q3 + q4)*((18589*3^(1/2))/4000000 + 1073/200000) + ddqr4*cos(q4 + q5)*((1369*3^(1/2))/4000000 - 12987/2500000) - ddqr5*cos(q4 + q5)*((1369*3^(1/2))/4000000 + 278943/40000000) - ddqr1*cos(q2 - q3 + 2*q4 - q5)*((23717*3^(1/2))/160000000 + 1369/8000000) - (259*3^(1/2)*ddqr1*cos(q2 - q3 + q5))/4000000 - (259*3^(1/2)*ddqr1*cos(q3 - q2 + q5))/4000000 - ddqr2*cos(q5)*((300773*3^(1/2))/40000000 - 1369/2000000) + ddqr3*cos(q5)*((300773*3^(1/2))/40000000 - 1369/2000000) + ddqr4*cos(q4)*((548467*3^(1/2))/80000000 + 32449/4000000) + (1073*3^(1/2)*ddqr2*cos(q3 + q5))/400000 + (1369*3^(1/2)*ddqr1*cos(q2 - q3 - q4 + 2*q5))/32000000 + ddqr1*cos(q3 - q2 + q4 + q5)*((1369*3^(1/2))/8000000 - 100011/40000000) + ddqr1*cos(q2 - q3 + q4 + q5)*((1369*3^(1/2))/8000000 - 107781/40000000) - ddqr2*cos(q3 - q4)*((18589*3^(1/2))/4000000 + 1073/200000) + ddqr4*cos(q4 - q5)*((1369*3^(1/2))/4000000 + 58349/20000000) + ddqr5*cos(q4 - q5)*((1369*3^(1/2))/4000000 - 45547/40000000) - ddqr2*cos(2*q4 + q5)*((71151*3^(1/2))/80000000 + 4107/4000000) + ddqr3*cos(2*q4 + q5)*((71151*3^(1/2))/80000000 + 4107/4000000) - (1369*3^(1/2)*ddqr5*cos(q4))/2000000 + (1369*dq3*dqr5*cos(2*q4)*sin(2*q5))/3200000 + (1369*dq3*dqr5*cos(2*q5)*sin(2*q4))/4000000;
Y3_7_1=(29*ddqr2*cos(q3))/100 + (ddqr1*cos(q2 - q3))/625 - (29*dq1*dqr1*sin(q3))/200 - (29*dq2*dqr2*sin(q3))/100 + (29*dq1*dqr1*cos(2*q2)*sin(q3))/200 - (29*dq1*dqr1*sin(2*q2)*cos(q3))/200;
Y3_8_1=(1231*ddqr2)/5000 - (1231*ddqr3)/5000 - (29*ddqr2*cos(q3))/100 + (7*ddqr1*cos(q2 - q3))/1000 + (29*dq1*dqr1*sin(q3))/200 + (29*dq2*dqr2*sin(q3))/100 - (29*dq1*dqr1*cos(2*q2)*sin(q3))/200 + (29*dq1*dqr1*sin(2*q2)*cos(q3))/200 + (1231*dq1*dqr1*cos(2*q2)*sin(2*q3))/10000 - (1231*dq1*dqr1*cos(2*q3)*sin(2*q2))/10000;
Y3_9_1=(7*ddqr1*cos(q2 - q3))/2000 - (29*ddqr2*cos(q3))/200 + ddqr2*((37*3^(1/2))/2000 + 117/625) - ddqr3*((37*3^(1/2))/2000 + 117/625) + (29*dq1*dqr1*sin(q3))/400 + (29*dq2*dqr2*sin(q3))/200 + (29*3^(1/2)*ddqr2*cos(q3 - q4))/400 - (37*3^(1/2)*ddqr2*cos(2*q4))/2000 + (37*3^(1/2)*ddqr3*cos(2*q4))/2000 - ddqr1*cos(q3 - q2 + q4)*((901*3^(1/2))/20000 + 37/4000) - ddqr1*cos(q2 - q3 + q4)*((971*3^(1/2))/20000 + 37/4000) - ddqr4*cos(q4)*((117*3^(1/2))/1250 + 37/2000) - (29*3^(1/2)*ddqr2*cos(q3 + q4))/400 + (37*3^(1/2)*ddqr1*cos(q2 - q3 + 2*q4))/4000 - (37*3^(1/2)*ddqr1*cos(q3 - q2 + 2*q4))/4000 + dq4*dqr4*sin(q4)*((117*3^(1/2))/1250 + 37/2000) - (29*dq1*dqr1*cos(2*q2)*sin(q3))/400 + (29*dq1*dqr1*sin(2*q2)*cos(q3))/400 + (37*3^(1/2)*dq2*dqr4*sin(2*q4))/2000 + (37*3^(1/2)*dq4*dqr2*sin(2*q4))/2000 - (37*3^(1/2)*dq3*dqr4*sin(2*q4))/2000 - (37*3^(1/2)*dq4*dqr3*sin(2*q4))/2000 + (29*3^(1/2)*dq1*dqr1*cos(q3)*sin(q4))/400 - (37*3^(1/2)*dq1*dqr4*cos(q2)*sin(q3))/2000 + (37*3^(1/2)*dq1*dqr4*cos(q3)*sin(q2))/2000 - (37*3^(1/2)*dq4*dqr1*cos(q2)*sin(q3))/2000 + (37*3^(1/2)*dq4*dqr1*cos(q3)*sin(q2))/2000 + (29*3^(1/2)*dq2*dqr2*cos(q3)*sin(q4))/200 - dq1*dqr1*cos(2*q2)*sin(2*q3)*((37*3^(1/2))/4000 - 117/1250) + dq1*dqr1*cos(2*q3)*sin(2*q2)*((37*3^(1/2))/4000 - 117/1250) + (37*3^(1/2)*dq1*dqr1*cos(2*q2)*cos(2*q4)*sin(2*q3))/4000 - (37*3^(1/2)*dq1*dqr1*cos(2*q3)*cos(2*q4)*sin(2*q2))/4000 - (29*3^(1/2)*dq1*dqr1*cos(2*q2)*cos(q3)*sin(q4))/400 + (37*3^(1/2)*dq1*dqr4*cos(2*q4)*cos(q2)*sin(q3))/2000 - (37*3^(1/2)*dq1*dqr4*cos(2*q4)*cos(q3)*sin(q2))/2000 + (37*3^(1/2)*dq4*dqr1*cos(2*q4)*cos(q2)*sin(q3))/2000 - (37*3^(1/2)*dq4*dqr1*cos(2*q4)*cos(q3)*sin(q2))/2000 + dq1*dqr1*cos(2*q2)*cos(2*q3)*sin(q4)*((117*3^(1/2))/1250 + 37/2000) - (29*3^(1/2)*dq1*dqr1*sin(2*q2)*sin(q3)*sin(q4))/400 + dq1*dqr1*sin(2*q2)*sin(2*q3)*sin(q4)*((117*3^(1/2))/1250 + 37/2000) + dq1*dqr4*cos(q2)*cos(q3)*sin(q4)*((117*3^(1/2))/1250 + 37/2000) + dq4*dqr1*cos(q2)*cos(q3)*sin(q4)*((117*3^(1/2))/1250 + 37/2000) + dq1*dqr4*sin(q2)*sin(q3)*sin(q4)*((117*3^(1/2))/1250 + 37/2000) + dq4*dqr1*sin(q2)*sin(q3)*sin(q4)*((117*3^(1/2))/1250 + 37/2000);
Y3_10_1=(29*dq1*dqr1*sin(q3))/800 + (29*dq2*dqr2*sin(q3))/400 + dq5*dqr2*sin(q5)*((37*3^(1/2))/16000 - 24387/160000) - (29*dq1*dqr1*cos(2*q2)*sin(q3))/800 + (29*dq1*dqr1*sin(2*q2)*cos(q3))/800 + (87*dq1*dqr1*cos(q5)*sin(q3))/800 + (87*dq2*dqr2*cos(q5)*sin(q3))/400 - (87*dq1*dqr1*cos(2*q2)*cos(q5)*sin(q3))/800 + (87*dq1*dqr1*sin(2*q2)*cos(q3)*cos(q5))/800 + (29*3^(1/2)*dq1*dqr1*cos(q3)*sin(q4))/800 + (29*3^(1/2)*dq2*dqr2*cos(q3)*sin(q4))/400 - (37*3^(1/2)*dq5*dqr1*cos(q2)*sin(q3))/4000 + (37*3^(1/2)*dq5*dqr1*cos(q3)*sin(q2))/4000 - dq4*dqr2*cos(2*q4)*sin(q5)*((111*3^(1/2))/4000 + 1923/40000) - dq4*dqr2*sin(2*q4)*cos(q5)*((111*3^(1/2))/8000 + 1923/80000) - dq5*dqr2*sin(2*q4)*cos(q5)*((111*3^(1/2))/8000 + 1923/80000) - dq5*dqr2*cos(2*q4)*sin(q5)*((111*3^(1/2))/16000 + 1923/160000) - (111*dq5*dqr1*cos(q2)*cos(q3)*sin(q4))/4000 - dq1*dqr1*cos(2*q2)*sin(2*q3)*((111*3^(1/2))/32000 - 6847/160000) + dq1*dqr1*cos(2*q3)*sin(2*q2)*((111*3^(1/2))/32000 - 6847/160000) - (111*dq5*dqr1*sin(q2)*sin(q3)*sin(q4))/4000 + (37*3^(1/2)*dq4*dqr2*cos(2*q5)*sin(2*q4))/3200 - dq4*dqr1*cos(q2)*sin(q3)*((333*3^(1/2))/16000 + 1923/80000) + dq4*dqr1*cos(q3)*sin(q2)*((333*3^(1/2))/16000 + 1923/80000) - (111*dq4*dqr1*cos(2*q5)*sin(q2)*sin(q3)*sin(q4))/8000 - (111*dq4*dqr1*sin(2*q5)*cos(q4)*sin(q2)*sin(q3))/4000 - (111*dq5*dqr1*cos(2*q5)*sin(q2)*sin(q3)*sin(q4))/4000 - (111*dq5*dqr1*sin(2*q5)*cos(q4)*sin(q2)*sin(q3))/8000 - (29*3^(1/2)*dq1*dqr1*cos(q3)*cos(q4)*sin(q5))/400 - (29*3^(1/2)*dq1*dqr1*cos(q3)*cos(q5)*sin(q4))/800 - (29*3^(1/2)*dq2*dqr2*cos(q3)*cos(q4)*sin(q5))/200 - (29*3^(1/2)*dq2*dqr2*cos(q3)*cos(q5)*sin(q4))/400 + (333*3^(1/2)*dq1*dqr1*cos(2*q2)*cos(2*q5)*sin(2*q3))/32000 - (333*3^(1/2)*dq1*dqr1*cos(2*q3)*cos(2*q5)*sin(2*q2))/32000 + dq4*dqr1*cos(2*q4)*cos(q2)*sin(q3)*((37*3^(1/2))/16000 + 1923/80000) - dq4*dqr1*cos(2*q4)*cos(q3)*sin(q2)*((37*3^(1/2))/16000 + 1923/80000) - (29*3^(1/2)*dq1*dqr1*cos(2*q2)*cos(q3)*sin(q4))/800 + (111*3^(1/2)*dq4*dqr1*cos(2*q5)*cos(q2)*sin(q3))/16000 - (111*3^(1/2)*dq4*dqr1*cos(2*q5)*cos(q3)*sin(q2))/16000 + dq1*dqr1*cos(2*q2)*cos(2*q3)*sin(q4)*((2513*3^(1/2))/40000 - 37/8000) + dq1*dqr1*cos(2*q2)*sin(2*q3)*cos(q5)*((37*3^(1/2))/3200 + 28233/160000) - dq1*dqr1*cos(2*q3)*sin(2*q2)*cos(q5)*((37*3^(1/2))/3200 + 28233/160000) - (29*3^(1/2)*dq1*dqr1*sin(2*q2)*sin(q3)*sin(q4))/800 - (111*dq1*dqr1*cos(2*q2)*cos(2*q3)*cos(2*q5)*sin(q4))/8000 - (111*dq1*dqr1*cos(2*q2)*cos(2*q3)*sin(2*q5)*cos(q4))/4000 + dq1*dqr1*sin(2*q2)*sin(2*q3)*sin(q4)*((2513*3^(1/2))/40000 - 37/8000) - (111*dq1*dqr1*cos(2*q5)*sin(2*q2)*sin(2*q3)*sin(q4))/8000 - (111*dq1*dqr1*sin(2*q2)*sin(2*q3)*sin(2*q5)*cos(q4))/4000 + dq4*dqr1*cos(q2)*cos(q3)*sin(q4)*((2513*3^(1/2))/40000 - 37/8000) + dq4*dqr1*cos(q2)*cos(q5)*sin(q3)*((111*3^(1/2))/8000 + 1923/80000) - dq4*dqr1*cos(q3)*cos(q5)*sin(q2)*((111*3^(1/2))/8000 + 1923/80000) + dq5*dqr1*cos(q2)*cos(q5)*sin(q3)*((111*3^(1/2))/8000 + 1923/80000) - dq5*dqr1*cos(q3)*cos(q5)*sin(q2)*((111*3^(1/2))/8000 + 1923/80000) - (111*dq4*dqr1*cos(2*q5)*cos(q2)*cos(q3)*sin(q4))/8000 - (111*dq4*dqr1*sin(2*q5)*cos(q2)*cos(q3)*cos(q4))/4000 - (111*dq5*dqr1*cos(2*q5)*cos(q2)*cos(q3)*sin(q4))/4000 - (111*dq5*dqr1*sin(2*q5)*cos(q2)*cos(q3)*cos(q4))/8000 + dq1*dqr1*cos(2*q2)*cos(2*q4)*sin(2*q3)*((37*3^(1/2))/32000 + 1923/160000) - dq1*dqr1*cos(2*q3)*cos(2*q4)*sin(2*q2)*((37*3^(1/2))/32000 + 1923/160000) + dq4*dqr1*sin(q2)*sin(q3)*sin(q4)*((2513*3^(1/2))/40000 - 37/8000) - dq4*dqr1*cos(2*q4)*cos(q2)*cos(q5)*sin(q3)*((111*3^(1/2))/8000 + 1923/80000) + dq4*dqr1*cos(2*q4)*cos(q3)*cos(q5)*sin(q2)*((111*3^(1/2))/8000 + 1923/80000) - dq5*dqr1*cos(2*q4)*cos(q2)*cos(q5)*sin(q3)*((111*3^(1/2))/8000 + 1923/80000) + dq5*dqr1*cos(2*q4)*cos(q3)*cos(q5)*sin(q2)*((111*3^(1/2))/8000 + 1923/80000) + dq4*dqr1*sin(2*q4)*cos(q2)*sin(q3)*sin(q5)*((111*3^(1/2))/4000 + 1923/40000) - dq4*dqr1*sin(2*q4)*cos(q3)*sin(q2)*sin(q5)*((111*3^(1/2))/4000 + 1923/40000) + dq5*dqr1*sin(2*q4)*cos(q2)*sin(q3)*sin(q5)*((111*3^(1/2))/16000 + 1923/160000) - dq5*dqr1*sin(2*q4)*cos(q3)*sin(q2)*sin(q5)*((111*3^(1/2))/16000 + 1923/160000) + (29*3^(1/2)*dq1*dqr1*cos(2*q2)*cos(q3)*cos(q4)*sin(q5))/400 + (29*3^(1/2)*dq1*dqr1*cos(2*q2)*cos(q3)*cos(q5)*sin(q4))/800 + (37*3^(1/2)*dq1*dqr1*cos(2*q2)*cos(2*q4)*cos(2*q5)*sin(2*q3))/6400 - (37*3^(1/2)*dq1*dqr1*cos(2*q3)*cos(2*q4)*cos(2*q5)*sin(2*q2))/6400 - dq1*dqr1*cos(2*q2)*cos(2*q3)*cos(q4)*sin(q5)*((877*3^(1/2))/8000 + 37/4000) - dq1*dqr1*cos(2*q2)*cos(2*q3)*cos(q5)*sin(q4)*((1231*3^(1/2))/40000 - 37/1000) + (29*3^(1/2)*dq1*dqr1*sin(2*q2)*cos(q4)*sin(q3)*sin(q5))/400 + (29*3^(1/2)*dq1*dqr1*sin(2*q2)*cos(q5)*sin(q3)*sin(q4))/800 - (37*3^(1/2)*dq1*dqr1*cos(2*q2)*sin(2*q3)*sin(2*q4)*sin(2*q5))/8000 + (37*3^(1/2)*dq1*dqr1*cos(2*q3)*sin(2*q2)*sin(2*q4)*sin(2*q5))/8000 - dq1*dqr1*sin(2*q2)*sin(2*q3)*cos(q4)*sin(q5)*((877*3^(1/2))/8000 + 37/4000) - dq1*dqr1*sin(2*q2)*sin(2*q3)*cos(q5)*sin(q4)*((1231*3^(1/2))/40000 - 37/1000) + (37*3^(1/2)*dq4*dqr1*cos(2*q4)*cos(2*q5)*cos(q2)*sin(q3))/3200 - (37*3^(1/2)*dq4*dqr1*cos(2*q4)*cos(2*q5)*cos(q3)*sin(q2))/3200 + (37*3^(1/2)*dq5*dqr1*cos(2*q4)*cos(2*q5)*cos(q2)*sin(q3))/4000 - (37*3^(1/2)*dq5*dqr1*cos(2*q4)*cos(2*q5)*cos(q3)*sin(q2))/4000 - dq4*dqr1*cos(q2)*cos(q3)*cos(q4)*sin(q5)*((877*3^(1/2))/8000 + 37/4000) - dq5*dqr1*cos(q2)*cos(q3)*cos(q5)*sin(q4)*((877*3^(1/2))/8000 + 37/4000) - dq5*dqr1*cos(q2)*cos(q3)*cos(q4)*sin(q5)*((877*3^(1/2))/16000 + 37/8000) - dq4*dqr1*cos(q2)*cos(q3)*cos(q5)*sin(q4)*((1231*3^(1/2))/40000 - 37/1000) - dq1*dqr1*cos(2*q2)*cos(2*q4)*sin(2*q3)*cos(q5)*((111*3^(1/2))/16000 + 1923/160000) + dq1*dqr1*cos(2*q3)*cos(2*q4)*sin(2*q2)*cos(q5)*((111*3^(1/2))/16000 + 1923/160000) - (37*3^(1/2)*dq4*dqr1*sin(2*q4)*sin(2*q5)*cos(q2)*sin(q3))/4000 + (37*3^(1/2)*dq4*dqr1*sin(2*q4)*sin(2*q5)*cos(q3)*sin(q2))/4000 - (37*3^(1/2)*dq5*dqr1*sin(2*q4)*sin(2*q5)*cos(q2)*sin(q3))/3200 + (37*3^(1/2)*dq5*dqr1*sin(2*q4)*sin(2*q5)*cos(q3)*sin(q2))/3200 - dq4*dqr1*cos(q4)*sin(q2)*sin(q3)*sin(q5)*((877*3^(1/2))/8000 + 37/4000) - dq5*dqr1*cos(q5)*sin(q2)*sin(q3)*sin(q4)*((877*3^(1/2))/8000 + 37/4000) - dq5*dqr1*cos(q4)*sin(q2)*sin(q3)*sin(q5)*((877*3^(1/2))/16000 + 37/8000) - dq4*dqr1*cos(q5)*sin(q2)*sin(q3)*sin(q4)*((1231*3^(1/2))/40000 - 37/1000) + dq1*dqr1*cos(2*q2)*sin(2*q3)*sin(2*q4)*sin(q5)*((111*3^(1/2))/8000 + 1923/80000) - dq1*dqr1*cos(2*q3)*sin(2*q2)*sin(2*q4)*sin(q5)*((111*3^(1/2))/8000 + 1923/80000);
Y3_10_2=dq4*dqr4*sin(q4)*((2513*3^(1/2))/40000 - 37/8000) - (111*dq5*dqr4*sin(q4))/4000 - (111*dq4*dqr5*sin(q4))/4000 + dq2*dqr5*sin(q5)*((37*3^(1/2))/16000 - 24387/160000) - dq3*dqr5*sin(q5)*((37*3^(1/2))/16000 - 24387/160000) - dq5*dqr3*sin(q5)*((37*3^(1/2))/16000 - 24387/160000) - (111*dq4*dqr4*cos(2*q5)*sin(q4))/8000 - (111*dq4*dqr4*sin(2*q5)*cos(q4))/4000 - (111*dq4*dqr5*cos(2*q5)*sin(q4))/4000 - (111*dq4*dqr5*sin(2*q5)*cos(q4))/8000 - (111*dq5*dqr4*cos(2*q5)*sin(q4))/4000 - (111*dq5*dqr4*sin(2*q5)*cos(q4))/8000 + dq2*dqr4*sin(2*q4)*((37*3^(1/2))/16000 + 1923/80000) + dq4*dqr2*sin(2*q4)*((37*3^(1/2))/16000 + 1923/80000) - dq3*dqr4*sin(2*q4)*((37*3^(1/2))/16000 + 1923/80000) - dq4*dqr3*sin(2*q4)*((37*3^(1/2))/16000 + 1923/80000) - (111*3^(1/2)*dq2*dqr5*sin(2*q5))/16000 - (111*3^(1/2)*dq5*dqr2*sin(2*q5))/16000 + (111*3^(1/2)*dq5*dqr3*sin(2*q5))/16000 - (37*3^(1/2)*dq1*dqr5*cos(q2)*sin(q3))/4000 + (37*3^(1/2)*dq1*dqr5*cos(q3)*sin(q2))/4000 - dq2*dqr4*cos(2*q4)*sin(q5)*((111*3^(1/2))/4000 + 1923/40000) + dq3*dqr4*cos(2*q4)*sin(q5)*((111*3^(1/2))/4000 + 1923/40000) + dq4*dqr3*cos(2*q4)*sin(q5)*((111*3^(1/2))/4000 + 1923/40000) - dq2*dqr4*sin(2*q4)*cos(q5)*((111*3^(1/2))/8000 + 1923/80000) - dq2*dqr5*sin(2*q4)*cos(q5)*((111*3^(1/2))/8000 + 1923/80000) + dq3*dqr4*sin(2*q4)*cos(q5)*((111*3^(1/2))/8000 + 1923/80000) + dq4*dqr3*sin(2*q4)*cos(q5)*((111*3^(1/2))/8000 + 1923/80000) + dq3*dqr5*sin(2*q4)*cos(q5)*((111*3^(1/2))/8000 + 1923/80000) + dq5*dqr3*sin(2*q4)*cos(q5)*((111*3^(1/2))/8000 + 1923/80000) - dq2*dqr5*cos(2*q4)*sin(q5)*((111*3^(1/2))/16000 + 1923/160000) + dq3*dqr5*cos(2*q4)*sin(q5)*((111*3^(1/2))/16000 + 1923/160000) + dq5*dqr3*cos(2*q4)*sin(q5)*((111*3^(1/2))/16000 + 1923/160000) - (111*dq1*dqr5*cos(q2)*cos(q3)*sin(q4))/4000 - (111*dq1*dqr5*sin(q2)*sin(q3)*sin(q4))/4000 + (37*3^(1/2)*dq2*dqr4*cos(2*q4)*sin(2*q5))/4000 + (37*3^(1/2)*dq2*dqr4*cos(2*q5)*sin(2*q4))/3200 + (37*3^(1/2)*dq4*dqr2*cos(2*q4)*sin(2*q5))/4000 + (37*3^(1/2)*dq2*dqr5*cos(2*q4)*sin(2*q5))/3200 + (37*3^(1/2)*dq2*dqr5*cos(2*q5)*sin(2*q4))/4000 - (37*3^(1/2)*dq3*dqr4*cos(2*q4)*sin(2*q5))/4000 - (37*3^(1/2)*dq3*dqr4*cos(2*q5)*sin(2*q4))/3200 - (37*3^(1/2)*dq4*dqr3*cos(2*q4)*sin(2*q5))/4000 - (37*3^(1/2)*dq4*dqr3*cos(2*q5)*sin(2*q4))/3200 + (37*3^(1/2)*dq5*dqr2*cos(2*q4)*sin(2*q5))/3200 + (37*3^(1/2)*dq5*dqr2*cos(2*q5)*sin(2*q4))/4000 - (37*3^(1/2)*dq5*dqr3*cos(2*q4)*sin(2*q5))/3200 - (37*3^(1/2)*dq5*dqr3*cos(2*q5)*sin(2*q4))/4000 - dq4*dqr4*cos(q4)*sin(q5)*((877*3^(1/2))/8000 + 37/4000) - dq4*dqr5*cos(q5)*sin(q4)*((877*3^(1/2))/8000 + 37/4000) - dq5*dqr4*cos(q5)*sin(q4)*((877*3^(1/2))/8000 + 37/4000) - dq5*dqr5*cos(q4)*sin(q5)*((877*3^(1/2))/8000 + 37/4000) - dq5*dqr5*cos(q5)*sin(q4)*((1577*3^(1/2))/20000 + 37/800) - dq4*dqr5*cos(q4)*sin(q5)*((877*3^(1/2))/16000 + 37/8000) - dq5*dqr4*cos(q4)*sin(q5)*((877*3^(1/2))/16000 + 37/8000) - dq4*dqr4*cos(q5)*sin(q4)*((1231*3^(1/2))/40000 - 37/1000) - dq1*dqr4*cos(q2)*sin(q3)*((333*3^(1/2))/16000 + 1923/80000) + dq1*dqr4*cos(q3)*sin(q2)*((333*3^(1/2))/16000 + 1923/80000) - (111*dq1*dqr4*cos(2*q5)*sin(q2)*sin(q3)*sin(q4))/8000 - (111*dq1*dqr4*sin(2*q5)*cos(q4)*sin(q2)*sin(q3))/4000 - (111*dq1*dqr5*cos(2*q5)*sin(q2)*sin(q3)*sin(q4))/4000 - (111*dq1*dqr5*sin(2*q5)*cos(q4)*sin(q2)*sin(q3))/8000 + dq1*dqr4*cos(2*q4)*cos(q2)*sin(q3)*((37*3^(1/2))/16000 + 1923/80000) - dq1*dqr4*cos(2*q4)*cos(q3)*sin(q2)*((37*3^(1/2))/16000 + 1923/80000) + (111*3^(1/2)*dq1*dqr4*cos(2*q5)*cos(q2)*sin(q3))/16000 - (111*3^(1/2)*dq1*dqr4*cos(2*q5)*cos(q3)*sin(q2))/16000 + dq1*dqr4*cos(q2)*cos(q3)*sin(q4)*((2513*3^(1/2))/40000 - 37/8000) + dq1*dqr4*cos(q2)*cos(q5)*sin(q3)*((111*3^(1/2))/8000 + 1923/80000) - dq1*dqr4*cos(q3)*cos(q5)*sin(q2)*((111*3^(1/2))/8000 + 1923/80000) + dq1*dqr5*cos(q2)*cos(q5)*sin(q3)*((111*3^(1/2))/8000 + 1923/80000) - dq1*dqr5*cos(q3)*cos(q5)*sin(q2)*((111*3^(1/2))/8000 + 1923/80000) - (111*dq1*dqr4*cos(2*q5)*cos(q2)*cos(q3)*sin(q4))/8000 - (111*dq1*dqr4*sin(2*q5)*cos(q2)*cos(q3)*cos(q4))/4000 - (111*dq1*dqr5*cos(2*q5)*cos(q2)*cos(q3)*sin(q4))/4000 - (111*dq1*dqr5*sin(2*q5)*cos(q2)*cos(q3)*cos(q4))/8000 + dq1*dqr4*sin(q2)*sin(q3)*sin(q4)*((2513*3^(1/2))/40000 - 37/8000) - dq1*dqr4*cos(2*q4)*cos(q2)*cos(q5)*sin(q3)*((111*3^(1/2))/8000 + 1923/80000) + dq1*dqr4*cos(2*q4)*cos(q3)*cos(q5)*sin(q2)*((111*3^(1/2))/8000 + 1923/80000) - dq1*dqr5*cos(2*q4)*cos(q2)*cos(q5)*sin(q3)*((111*3^(1/2))/8000 + 1923/80000) + dq1*dqr5*cos(2*q4)*cos(q3)*cos(q5)*sin(q2)*((111*3^(1/2))/8000 + 1923/80000) + dq1*dqr4*sin(2*q4)*cos(q2)*sin(q3)*sin(q5)*((111*3^(1/2))/4000 + 1923/40000) - dq1*dqr4*sin(2*q4)*cos(q3)*sin(q2)*sin(q5)*((111*3^(1/2))/4000 + 1923/40000) + dq1*dqr5*sin(2*q4)*cos(q2)*sin(q3)*sin(q5)*((111*3^(1/2))/16000 + 1923/160000) - dq1*dqr5*sin(2*q4)*cos(q3)*sin(q2)*sin(q5)*((111*3^(1/2))/16000 + 1923/160000) + (37*3^(1/2)*dq1*dqr4*cos(2*q4)*cos(2*q5)*cos(q2)*sin(q3))/3200 - (37*3^(1/2)*dq1*dqr4*cos(2*q4)*cos(2*q5)*cos(q3)*sin(q2))/3200 + (37*3^(1/2)*dq1*dqr5*cos(2*q4)*cos(2*q5)*cos(q2)*sin(q3))/4000 - (37*3^(1/2)*dq1*dqr5*cos(2*q4)*cos(2*q5)*cos(q3)*sin(q2))/4000 - dq1*dqr4*cos(q2)*cos(q3)*cos(q4)*sin(q5)*((877*3^(1/2))/8000 + 37/4000) - dq1*dqr5*cos(q2)*cos(q3)*cos(q5)*sin(q4)*((877*3^(1/2))/8000 + 37/4000) - dq1*dqr5*cos(q2)*cos(q3)*cos(q4)*sin(q5)*((877*3^(1/2))/16000 + 37/8000) - dq1*dqr4*cos(q2)*cos(q3)*cos(q5)*sin(q4)*((1231*3^(1/2))/40000 - 37/1000) - (37*3^(1/2)*dq1*dqr4*sin(2*q4)*sin(2*q5)*cos(q2)*sin(q3))/4000 + (37*3^(1/2)*dq1*dqr4*sin(2*q4)*sin(2*q5)*cos(q3)*sin(q2))/4000 - (37*3^(1/2)*dq1*dqr5*sin(2*q4)*sin(2*q5)*cos(q2)*sin(q3))/3200 + (37*3^(1/2)*dq1*dqr5*sin(2*q4)*sin(2*q5)*cos(q3)*sin(q2))/3200 - dq1*dqr4*cos(q4)*sin(q2)*sin(q3)*sin(q5)*((877*3^(1/2))/8000 + 37/4000) - dq1*dqr5*cos(q5)*sin(q2)*sin(q3)*sin(q4)*((877*3^(1/2))/8000 + 37/4000) - dq1*dqr5*cos(q4)*sin(q2)*sin(q3)*sin(q5)*((877*3^(1/2))/16000 + 37/8000) - dq1*dqr4*cos(q5)*sin(q2)*sin(q3)*sin(q4)*((1231*3^(1/2))/40000 - 37/1000);
Y3_10_3=(333*ddqr1*cos(q2 - q3 + q4 + 2*q5))/32000 - (111*ddqr1*cos(q2 - q3 + q4 - 2*q5))/32000 + (333*ddqr1*cos(q3 - q2 + q4 + 2*q5))/32000 + (21*ddqr1*cos(q2 - q3 + q5))/8000 + (21*ddqr1*cos(q3 - q2 + q5))/8000 - (87*ddqr2*cos(q3 + q5))/800 - (111*ddqr1*cos(q2 - q3 - q4 + 2*q5))/32000 - (29*ddqr2*cos(q3))/400 + (111*ddqr5*cos(q4))/2000 + (7*ddqr1*cos(q2 - q3))/4000 - (87*ddqr2*cos(q3 - q5))/800 - (111*ddqr4*cos(q4 - 2*q5))/16000 + (333*ddqr4*cos(q4 + 2*q5))/16000 + ddqr2*((111*3^(1/2))/3200 + 10693/80000) - ddqr3*((111*3^(1/2))/3200 + 10693/80000) - ddqr2*cos(2*q4)*((37*3^(1/2))/16000 + 1923/80000) + ddqr3*cos(2*q4)*((37*3^(1/2))/16000 + 1923/80000) + (29*3^(1/2)*ddqr2*cos(q3 - q4))/800 - ddqr1*cos(q2 - q3 + q4 - q5)*((403*3^(1/2))/20000 + 37/3200) - ddqr1*cos(q2 - q3 - q4 + q5)*((771*3^(1/2))/40000 + 37/3200) - ddqr1*cos(q2 - q3 - 2*q4 + q5)*((111*3^(1/2))/32000 + 1923/320000) - ddqr1*cos(q2 - q3 + 2*q4 + q5)*((333*3^(1/2))/32000 + 5769/320000) + ddqr1*cos(q3 - q2 + 2*q4 + q5)*((333*3^(1/2))/32000 + 5769/320000) + (87*3^(1/2)*ddqr2*cos(q3 + q4 + q5))/1600 - ddqr2*cos(2*q4 - q5)*((111*3^(1/2))/16000 + 1923/160000) + ddqr3*cos(2*q4 - q5)*((111*3^(1/2))/16000 + 1923/160000) + (111*3^(1/2)*ddqr2*cos(2*q5))/16000 - (111*3^(1/2)*ddqr3*cos(2*q5))/16000 - ddqr1*cos(q3 - q2 + q4)*((2443*3^(1/2))/80000 - 37/16000) - ddqr1*cos(q2 - q3 + q4)*((2583*3^(1/2))/80000 - 37/16000) - (37*3^(1/2)*ddqr2*cos(2*q4 - 2*q5))/32000 - (333*3^(1/2)*ddqr2*cos(2*q4 + 2*q5))/32000 + (37*3^(1/2)*ddqr3*cos(2*q4 - 2*q5))/32000 + (333*3^(1/2)*ddqr3*cos(2*q4 + 2*q5))/32000 + ddqr4*cos(q4 + q5)*((351*3^(1/2))/5000 - 111/8000) + ddqr5*cos(q4 + q5)*((7539*3^(1/2))/80000 + 111/4000) + ddqr1*cos(q2 - q3 + 2*q4 - q5)*((111*3^(1/2))/32000 + 1923/320000) - (29*3^(1/2)*ddqr2*cos(q3 + q4 - q5))/1600 + (29*3^(1/2)*ddqr2*cos(q3 - q4 + q5))/1600 - (87*3^(1/2)*ddqr2*cos(q4 - q3 + q5))/1600 - ddqr4*cos(q4)*((2513*3^(1/2))/40000 - 37/8000) - ddqr2*cos(q5)*((37*3^(1/2))/8000 - 24387/80000) + ddqr3*cos(q5)*((37*3^(1/2))/8000 - 24387/80000) + ddqr1*cos(q2 - q3 + 2*q4)*((37*3^(1/2))/32000 + 1923/160000) - ddqr1*cos(q3 - q2 + 2*q4)*((37*3^(1/2))/32000 + 1923/160000) - (29*3^(1/2)*ddqr2*cos(q3 + q4))/800 - (37*3^(1/2)*ddqr1*cos(q2 - q3 - 2*q4 + 2*q5))/64000 + (37*3^(1/2)*ddqr1*cos(q2 - q3 + 2*q4 - 2*q5))/64000 + (333*3^(1/2)*ddqr1*cos(q2 - q3 + 2*q4 + 2*q5))/64000 - (333*3^(1/2)*ddqr1*cos(q3 - q2 + 2*q4 + 2*q5))/64000 + ddqr1*cos(q3 - q2 + q4 + q5)*((2703*3^(1/2))/80000 - 111/16000) + ddqr1*cos(q2 - q3 + q4 + q5)*((2913*3^(1/2))/80000 - 111/16000) - ddqr4*cos(q4 - q5)*((1577*3^(1/2))/40000 + 37/1600) + ddqr5*cos(q4 - q5)*((1231*3^(1/2))/80000 - 37/2000) + ddqr2*cos(2*q4 + q5)*((333*3^(1/2))/16000 + 5769/160000) - ddqr3*cos(2*q4 + q5)*((333*3^(1/2))/16000 + 5769/160000) + (111*3^(1/2)*dq3*dqr5*sin(2*q5))/16000 - (37*3^(1/2)*dq3*dqr5*cos(2*q4)*sin(2*q5))/3200 - (37*3^(1/2)*dq3*dqr5*cos(2*q5)*sin(2*q4))/4000;
Y3_12_1=(1231*sin(q2 - q3))/10000;
Y3_13_1=(117*sin(q2 - q3))/625 - (37*sin(q2 - q3 + q4))/2000 - (37*sin(q3 - q2 + q4))/2000;
Y3_14_1=(877*sin(q2 - q3))/4000 - (37*sin(q2 - q3 + q4 - q5))/8000 + (37*sin(q2 - q3 - q4 + q5))/8000 + (111*sin(q2 - q3 + q4 + q5))/8000 + (111*sin(q3 - q2 + q4 + q5))/8000 - sin(q2 - q3 + q4)*((641*3^(1/2))/40000 + 37/2000) - sin(q3 - q2 + q4)*((641*3^(1/2))/40000 + 37/2000) + (37*3^(1/2)*sin(q2 - q3 + q5))/4000 - (37*3^(1/2)*sin(q3 - q2 + q5))/4000;
Y3_16_1=ddqr3 - ddqr2 - (dq1*dqr1*cos(2*q2)*sin(2*q3))/2 + (dq1*dqr1*cos(2*q3)*sin(2*q2))/2;
Y3_17_1=ddqr3 - ddqr2 - (dq1*dqr1*cos(2*q2)*sin(2*q3))/2 + (dq1*dqr1*cos(2*q3)*sin(2*q2))/2;
Y3_18_1=(5*ddqr3)/8 - (5*ddqr2)/8 - (3*ddqr1*cos(q2 - q3 + 2*q4))/16 + (3*ddqr1*cos(q3 - q2 + 2*q4))/16 + (3*ddqr2*cos(2*q4))/8 - (3*ddqr3*cos(2*q4))/8 - (3*dq2*dqr4*sin(2*q4))/8 - (3*dq4*dqr2*sin(2*q4))/8 + (3*dq3*dqr4*sin(2*q4))/8 + (3*dq4*dqr3*sin(2*q4))/8 + (3^(1/2)*ddqr1*cos(q2 - q3 + q4))/8 + (3^(1/2)*ddqr1*cos(q3 - q2 + q4))/8 + (3^(1/2)*ddqr4*cos(q4))/4 - (3^(1/2)*dq4*dqr4*sin(q4))/4 + (dq1*dqr1*cos(2*q2)*sin(2*q3))/16 - (dq1*dqr1*cos(2*q3)*sin(2*q2))/16 + (3*dq1*dqr4*cos(q2)*sin(q3))/8 - (3*dq1*dqr4*cos(q3)*sin(q2))/8 + (3*dq4*dqr1*cos(q2)*sin(q3))/8 - (3*dq4*dqr1*cos(q3)*sin(q2))/8 - (3*dq1*dqr4*cos(2*q4)*cos(q2)*sin(q3))/8 + (3*dq1*dqr4*cos(2*q4)*cos(q3)*sin(q2))/8 - (3*dq4*dqr1*cos(2*q4)*cos(q2)*sin(q3))/8 + (3*dq4*dqr1*cos(2*q4)*cos(q3)*sin(q2))/8 - (3*dq1*dqr1*cos(2*q2)*cos(2*q4)*sin(2*q3))/16 + (3*dq1*dqr1*cos(2*q3)*cos(2*q4)*sin(2*q2))/16 - (3^(1/2)*dq1*dqr4*cos(q2)*cos(q3)*sin(q4))/4 - (3^(1/2)*dq4*dqr1*cos(q2)*cos(q3)*sin(q4))/4 - (3^(1/2)*dq1*dqr4*sin(q2)*sin(q3)*sin(q4))/4 - (3^(1/2)*dq4*dqr1*sin(q2)*sin(q3)*sin(q4))/4 - (3^(1/2)*dq1*dqr1*cos(2*q2)*cos(2*q3)*sin(q4))/4 - (3^(1/2)*dq1*dqr1*sin(2*q2)*sin(2*q3)*sin(q4))/4;
Y3_19_1=(3*dq5*dqr2*sin(q5))/32 - (3*dq5*dqr3*sin(q5))/32 + (3*dq4*dqr2*sin(2*q4))/64 - (3*dq4*dqr3*sin(2*q4))/64 + (9*dq5*dqr2*sin(2*q5))/64 - (9*dq5*dqr3*sin(2*q5))/64 + (3*dq4*dqr2*cos(2*q4)*sin(q5))/8 + (3*dq4*dqr2*sin(2*q4)*cos(q5))/16 - (3*dq4*dqr3*cos(2*q4)*sin(q5))/8 - (3*dq4*dqr3*sin(2*q4)*cos(q5))/16 + (3*dq5*dqr2*cos(2*q4)*sin(q5))/32 + (3*dq5*dqr2*sin(2*q4)*cos(q5))/16 - (3*dq5*dqr3*cos(2*q4)*sin(q5))/32 - (3*dq5*dqr3*sin(2*q4)*cos(q5))/16 - (dq1*dqr1*cos(2*q2)*sin(2*q3))/128 + (dq1*dqr1*cos(2*q3)*sin(2*q2))/128 - (3*dq4*dqr2*cos(2*q4)*sin(2*q5))/16 - (15*dq4*dqr2*cos(2*q5)*sin(2*q4))/64 + (3*dq4*dqr3*cos(2*q4)*sin(2*q5))/16 + (15*dq4*dqr3*cos(2*q5)*sin(2*q4))/64 - (15*dq5*dqr2*cos(2*q4)*sin(2*q5))/64 - (3*dq5*dqr2*cos(2*q5)*sin(2*q4))/16 + (15*dq5*dqr3*cos(2*q4)*sin(2*q5))/64 + (3*dq5*dqr3*cos(2*q5)*sin(2*q4))/16 + (21*dq4*dqr1*cos(q2)*sin(q3))/64 - (21*dq4*dqr1*cos(q3)*sin(q2))/64 + (3*dq5*dqr1*cos(q2)*sin(q3))/16 - (3*dq5*dqr1*cos(q3)*sin(q2))/16 + (3*dq4*dqr1*cos(2*q4)*cos(q2)*sin(q3))/64 - (3*dq4*dqr1*cos(2*q4)*cos(q3)*sin(q2))/64 - (9*dq4*dqr1*cos(2*q5)*cos(q2)*sin(q3))/64 + (9*dq4*dqr1*cos(2*q5)*cos(q3)*sin(q2))/64 - (9*dq1*dqr1*cos(2*q2)*sin(2*q3)*cos(q5))/32 + (9*dq1*dqr1*cos(2*q3)*sin(2*q2)*cos(q5))/32 - (3*dq4*dqr1*cos(q2)*cos(q5)*sin(q3))/16 + (3*dq4*dqr1*cos(q3)*cos(q5)*sin(q2))/16 - (3*dq5*dqr1*cos(q2)*cos(q5)*sin(q3))/16 + (3*dq5*dqr1*cos(q3)*cos(q5)*sin(q2))/16 + (3*dq1*dqr1*cos(2*q2)*cos(2*q4)*sin(2*q3))/128 - (3*dq1*dqr1*cos(2*q3)*cos(2*q4)*sin(2*q2))/128 - (27*dq1*dqr1*cos(2*q2)*cos(2*q5)*sin(2*q3))/128 + (27*dq1*dqr1*cos(2*q3)*cos(2*q5)*sin(2*q2))/128 - (15*dq1*dqr1*cos(2*q2)*cos(2*q4)*cos(2*q5)*sin(2*q3))/128 + (15*dq1*dqr1*cos(2*q3)*cos(2*q4)*cos(2*q5)*sin(2*q2))/128 - (3*dq4*dqr1*sin(2*q4)*cos(q2)*sin(q3)*sin(q5))/8 + (3*dq4*dqr1*sin(2*q4)*cos(q3)*sin(q2)*sin(q5))/8 - (3*dq5*dqr1*sin(2*q4)*cos(q2)*sin(q3)*sin(q5))/32 + (3*dq5*dqr1*sin(2*q4)*cos(q3)*sin(q2)*sin(q5))/32 + (3^(1/2)*dq4*dqr1*cos(q2)*cos(q3)*sin(q4))/32 + (3*3^(1/2)*dq5*dqr1*cos(q2)*cos(q3)*sin(q4))/16 + (3*dq1*dqr1*cos(2*q2)*sin(2*q3)*sin(2*q4)*sin(2*q5))/32 - (3*dq1*dqr1*cos(2*q3)*sin(2*q2)*sin(2*q4)*sin(2*q5))/32 + (3^(1/2)*dq1*dqr4*sin(q2)*sin(q3)*sin(q4))/32 + (3^(1/2)*dq4*dqr1*sin(q2)*sin(q3)*sin(q4))/32 + (3*3^(1/2)*dq5*dqr1*sin(q2)*sin(q3)*sin(q4))/16 - (15*dq4*dqr1*cos(2*q4)*cos(2*q5)*cos(q2)*sin(q3))/64 + (15*dq4*dqr1*cos(2*q4)*cos(2*q5)*cos(q3)*sin(q2))/64 - (3*dq5*dqr1*cos(2*q4)*cos(2*q5)*cos(q2)*sin(q3))/16 + (3*dq5*dqr1*cos(2*q4)*cos(2*q5)*cos(q3)*sin(q2))/16 + (3*dq4*dqr1*sin(2*q4)*sin(2*q5)*cos(q2)*sin(q3))/16 - (3*dq4*dqr1*sin(2*q4)*sin(2*q5)*cos(q3)*sin(q2))/16 + (15*dq5*dqr1*sin(2*q4)*sin(2*q5)*cos(q2)*sin(q3))/64 - (15*dq5*dqr1*sin(2*q4)*sin(2*q5)*cos(q3)*sin(q2))/64 + (3*dq1*dqr1*cos(2*q2)*cos(2*q4)*sin(2*q3)*cos(q5))/32 - (3*dq1*dqr1*cos(2*q3)*cos(2*q4)*sin(2*q2)*cos(q5))/32 - (3*dq1*dqr1*cos(2*q2)*sin(2*q3)*sin(2*q4)*sin(q5))/16 + (3*dq1*dqr1*cos(2*q3)*sin(2*q2)*sin(2*q4)*sin(q5))/16 + (3^(1/2)*dq1*dqr1*cos(2*q2)*cos(2*q3)*sin(q4))/32 + (3*dq4*dqr1*cos(2*q4)*cos(q2)*cos(q5)*sin(q3))/16 - (3*dq4*dqr1*cos(2*q4)*cos(q3)*cos(q5)*sin(q2))/16 + (3*dq5*dqr1*cos(2*q4)*cos(q2)*cos(q5)*sin(q3))/16 - (3*dq5*dqr1*cos(2*q4)*cos(q3)*cos(q5)*sin(q2))/16 + (3^(1/2)*dq1*dqr1*sin(2*q2)*sin(2*q3)*sin(q4))/32 + (3*3^(1/2)*dq1*dqr1*cos(2*q2)*cos(2*q3)*cos(2*q5)*sin(q4))/32 + (3*3^(1/2)*dq1*dqr1*cos(2*q2)*cos(2*q3)*sin(2*q5)*cos(q4))/16 + (3^(1/2)*dq1*dqr4*cos(q4)*sin(q2)*sin(q3)*sin(q5))/8 - (3^(1/2)*dq1*dqr4*cos(q5)*sin(q2)*sin(q3)*sin(q4))/8 + (3^(1/2)*dq4*dqr1*cos(q4)*sin(q2)*sin(q3)*sin(q5))/8 - (3^(1/2)*dq4*dqr1*cos(q5)*sin(q2)*sin(q3)*sin(q4))/8 + (3^(1/2)*dq5*dqr1*cos(q4)*sin(q2)*sin(q3)*sin(q5))/16 + (3^(1/2)*dq5*dqr1*cos(q5)*sin(q2)*sin(q3)*sin(q4))/8 + (3*3^(1/2)*dq1*dqr1*cos(2*q5)*sin(2*q2)*sin(2*q3)*sin(q4))/32 + (3*3^(1/2)*dq1*dqr1*sin(2*q2)*sin(2*q3)*sin(2*q5)*cos(q4))/16 + (3*3^(1/2)*dq4*dqr1*cos(2*q5)*cos(q2)*cos(q3)*sin(q4))/32 + (3*3^(1/2)*dq4*dqr1*sin(2*q5)*cos(q2)*cos(q3)*cos(q4))/16 + (3*3^(1/2)*dq5*dqr1*cos(2*q5)*cos(q2)*cos(q3)*sin(q4))/16 + (3*3^(1/2)*dq5*dqr1*sin(2*q5)*cos(q2)*cos(q3)*cos(q4))/32 + (3*3^(1/2)*dq1*dqr4*cos(2*q5)*sin(q2)*sin(q3)*sin(q4))/32 + (3*3^(1/2)*dq4*dqr1*cos(2*q5)*sin(q2)*sin(q3)*sin(q4))/32 + (3*3^(1/2)*dq4*dqr1*sin(2*q5)*cos(q4)*sin(q2)*sin(q3))/16 + (3*3^(1/2)*dq5*dqr1*cos(2*q5)*sin(q2)*sin(q3)*sin(q4))/16 + (3*3^(1/2)*dq5*dqr1*sin(2*q5)*cos(q4)*sin(q2)*sin(q3))/32 + (3^(1/2)*dq1*dqr1*cos(2*q2)*cos(2*q3)*cos(q4)*sin(q5))/8 - (3^(1/2)*dq1*dqr1*cos(2*q2)*cos(2*q3)*cos(q5)*sin(q4))/8 + (3^(1/2)*dq1*dqr1*sin(2*q2)*sin(2*q3)*cos(q4)*sin(q5))/8 - (3^(1/2)*dq1*dqr1*sin(2*q2)*sin(2*q3)*cos(q5)*sin(q4))/8 + (3^(1/2)*dq4*dqr1*cos(q2)*cos(q3)*cos(q4)*sin(q5))/8 - (3^(1/2)*dq4*dqr1*cos(q2)*cos(q3)*cos(q5)*sin(q4))/8 + (3^(1/2)*dq5*dqr1*cos(q2)*cos(q3)*cos(q4)*sin(q5))/16 + (3^(1/2)*dq5*dqr1*cos(q2)*cos(q3)*cos(q5)*sin(q4))/8;
Y3_19_2=(3*ddqr1*cos(q2 - q3 - 2*q4 + q5))/64 + (9*ddqr1*cos(q2 - q3 + 2*q4 + q5))/64 - (9*ddqr1*cos(q3 - q2 + 2*q4 + q5))/64 - (3*ddqr1*cos(q2 - q3 + 2*q4 - q5))/64 + (3*ddqr1*cos(q2 - q3 - 2*q4 + 2*q5))/256 - (3*ddqr1*cos(q2 - q3 + 2*q4 - 2*q5))/256 - (27*ddqr1*cos(q2 - q3 + 2*q4 + 2*q5))/256 + (27*ddqr1*cos(q3 - q2 + 2*q4 + 2*q5))/256 + (3*ddqr1*cos(q2 - q3 + 2*q4))/128 - (3*ddqr1*cos(q3 - q2 + 2*q4))/128 + (3*dq2*dqr5*sin(q5))/32 - (3*dq3*dqr5*sin(q5))/32 + (3^(1/2)*ddqr1*cos(q2 - q3 + q4 - q5))/16 + (3^(1/2)*ddqr1*cos(q2 - q3 - q4 + q5))/16 + (3*3^(1/2)*ddqr1*cos(q2 - q3 + q4 - 2*q5))/128 - (9*3^(1/2)*ddqr1*cos(q2 - q3 + q4 + 2*q5))/128 - (9*3^(1/2)*ddqr1*cos(q3 - q2 + q4 + 2*q5))/128 + (3*dq2*dqr4*sin(2*q4))/64 - (3*dq3*dqr4*sin(2*q4))/64 + (9*dq2*dqr5*sin(2*q5))/64 - (9*dq3*dqr5*sin(2*q5))/64 - (3^(1/2)*ddqr1*cos(q2 - q3 + q4))/64 + (3*3^(1/2)*ddqr1*cos(q2 - q3 - q4 + 2*q5))/128 + (3*dq2*dqr4*cos(2*q4)*sin(q5))/8 + (3*dq2*dqr4*sin(2*q4)*cos(q5))/16 + (3*dq2*dqr5*cos(2*q4)*sin(q5))/32 + (3*dq2*dqr5*sin(2*q4)*cos(q5))/16 - (3*dq3*dqr4*cos(2*q4)*sin(q5))/8 - (3*dq3*dqr4*sin(2*q4)*cos(q5))/16 - (3*dq3*dqr5*cos(2*q4)*sin(q5))/32 - (3*dq3*dqr5*sin(2*q4)*cos(q5))/16 + (3^(1/2)*dq4*dqr4*sin(q4))/32 + (3*3^(1/2)*dq4*dqr5*sin(q4))/16 + (3*3^(1/2)*dq5*dqr4*sin(q4))/16 - (3*dq2*dqr4*cos(2*q4)*sin(2*q5))/16 - (15*dq2*dqr4*cos(2*q5)*sin(2*q4))/64 - (15*dq2*dqr5*cos(2*q4)*sin(2*q5))/64 - (3*dq2*dqr5*cos(2*q5)*sin(2*q4))/16 + (3*dq3*dqr4*cos(2*q4)*sin(2*q5))/16 + (15*dq3*dqr4*cos(2*q5)*sin(2*q4))/64 + (15*dq3*dqr5*cos(2*q4)*sin(2*q5))/64 + (3*dq3*dqr5*cos(2*q5)*sin(2*q4))/16 + (21*dq1*dqr4*cos(q2)*sin(q3))/64 - (21*dq1*dqr4*cos(q3)*sin(q2))/64 + (3*dq1*dqr5*cos(q2)*sin(q3))/16 - (3*dq1*dqr5*cos(q3)*sin(q2))/16 + (3*dq1*dqr4*cos(2*q4)*cos(q2)*sin(q3))/64 - (3*dq1*dqr4*cos(2*q4)*cos(q3)*sin(q2))/64 - (9*dq1*dqr4*cos(2*q5)*cos(q2)*sin(q3))/64 + (9*dq1*dqr4*cos(2*q5)*cos(q3)*sin(q2))/64 + (3^(1/2)*dq4*dqr4*cos(q4)*sin(q5))/8 - (3^(1/2)*dq4*dqr4*cos(q5)*sin(q4))/8 + (3^(1/2)*dq4*dqr5*cos(q4)*sin(q5))/16 + (3^(1/2)*dq4*dqr5*cos(q5)*sin(q4))/8 + (3^(1/2)*dq5*dqr4*cos(q4)*sin(q5))/16 + (3^(1/2)*dq5*dqr4*cos(q5)*sin(q4))/8 + (3^(1/2)*dq5*dqr5*cos(q4)*sin(q5))/8 + (3^(1/2)*dq5*dqr5*cos(q5)*sin(q4))/4 + (3*3^(1/2)*dq4*dqr4*cos(2*q5)*sin(q4))/32 + (3*3^(1/2)*dq4*dqr4*sin(2*q5)*cos(q4))/16 + (3*3^(1/2)*dq4*dqr5*cos(2*q5)*sin(q4))/16 + (3*3^(1/2)*dq4*dqr5*sin(2*q5)*cos(q4))/32 + (3*3^(1/2)*dq5*dqr4*cos(2*q5)*sin(q4))/16 + (3*3^(1/2)*dq5*dqr4*sin(2*q5)*cos(q4))/32 - (3*dq1*dqr4*cos(q2)*cos(q5)*sin(q3))/16 + (3*dq1*dqr4*cos(q3)*cos(q5)*sin(q2))/16 - (3*dq1*dqr5*cos(q2)*cos(q5)*sin(q3))/16 + (3*dq1*dqr5*cos(q3)*cos(q5)*sin(q2))/16 - (3*dq1*dqr4*sin(2*q4)*cos(q2)*sin(q3)*sin(q5))/8 + (3*dq1*dqr4*sin(2*q4)*cos(q3)*sin(q2)*sin(q5))/8 - (3*dq1*dqr5*sin(2*q4)*cos(q2)*sin(q3)*sin(q5))/32 + (3*dq1*dqr5*sin(2*q4)*cos(q3)*sin(q2)*sin(q5))/32 + (3^(1/2)*dq1*dqr4*cos(q2)*cos(q3)*sin(q4))/32 + (3*3^(1/2)*dq1*dqr5*cos(q2)*cos(q3)*sin(q4))/16 + (3*3^(1/2)*dq1*dqr5*sin(q2)*sin(q3)*sin(q4))/16 - (15*dq1*dqr4*cos(2*q4)*cos(2*q5)*cos(q2)*sin(q3))/64 + (15*dq1*dqr4*cos(2*q4)*cos(2*q5)*cos(q3)*sin(q2))/64 - (3*dq1*dqr5*cos(2*q4)*cos(2*q5)*cos(q2)*sin(q3))/16 + (3*dq1*dqr5*cos(2*q4)*cos(2*q5)*cos(q3)*sin(q2))/16 + (3*dq1*dqr4*sin(2*q4)*sin(2*q5)*cos(q2)*sin(q3))/16 - (3*dq1*dqr4*sin(2*q4)*sin(2*q5)*cos(q3)*sin(q2))/16 + (15*dq1*dqr5*sin(2*q4)*sin(2*q5)*cos(q2)*sin(q3))/64 - (15*dq1*dqr5*sin(2*q4)*sin(2*q5)*cos(q3)*sin(q2))/64 + (3*dq1*dqr4*cos(2*q4)*cos(q2)*cos(q5)*sin(q3))/16 - (3*dq1*dqr4*cos(2*q4)*cos(q3)*cos(q5)*sin(q2))/16 + (3*dq1*dqr5*cos(2*q4)*cos(q2)*cos(q5)*sin(q3))/16 - (3*dq1*dqr5*cos(2*q4)*cos(q3)*cos(q5)*sin(q2))/16 + (3^(1/2)*dq1*dqr5*cos(q4)*sin(q2)*sin(q3)*sin(q5))/16 + (3^(1/2)*dq1*dqr5*cos(q5)*sin(q2)*sin(q3)*sin(q4))/8 + (3*3^(1/2)*dq1*dqr4*cos(2*q5)*cos(q2)*cos(q3)*sin(q4))/32 + (3*3^(1/2)*dq1*dqr4*sin(2*q5)*cos(q2)*cos(q3)*cos(q4))/16 + (3*3^(1/2)*dq1*dqr5*cos(2*q5)*cos(q2)*cos(q3)*sin(q4))/16 + (3*3^(1/2)*dq1*dqr5*sin(2*q5)*cos(q2)*cos(q3)*cos(q4))/32 + (3*3^(1/2)*dq1*dqr4*sin(2*q5)*cos(q4)*sin(q2)*sin(q3))/16 + (3*3^(1/2)*dq1*dqr5*cos(2*q5)*sin(q2)*sin(q3)*sin(q4))/16 + (3*3^(1/2)*dq1*dqr5*sin(2*q5)*cos(q4)*sin(q2)*sin(q3))/32 + (3^(1/2)*dq1*dqr4*cos(q2)*cos(q3)*cos(q4)*sin(q5))/8 - (3^(1/2)*dq1*dqr4*cos(q2)*cos(q3)*cos(q5)*sin(q4))/8 + (3^(1/2)*dq1*dqr5*cos(q2)*cos(q3)*cos(q4)*sin(q5))/16 + (3^(1/2)*dq1*dqr5*cos(q2)*cos(q3)*cos(q5)*sin(q4))/8;
Y3_19_3=(43*ddqr3)/64 - (43*ddqr2)/64 + (3*ddqr2*cos(2*q4 - q5))/32 + (3*ddqr2*cos(2*q4 - 2*q5))/128 + (27*ddqr2*cos(2*q4 + 2*q5))/128 - (3*ddqr3*cos(2*q4 - q5))/32 - (3*ddqr3*cos(2*q4 - 2*q5))/128 - (27*ddqr3*cos(2*q4 + 2*q5))/128 - (3*ddqr2*cos(q5))/16 + (3*ddqr3*cos(q5))/16 - (9*ddqr2*cos(2*q4 + q5))/32 + (9*ddqr3*cos(2*q4 + q5))/32 - (3*ddqr2*cos(2*q4))/64 - (9*ddqr2*cos(2*q5))/64 + (3*ddqr3*cos(2*q4))/64 + (9*ddqr3*cos(2*q5))/64 + (3^(1/2)*ddqr4*cos(q4 - q5))/8 + (3*3^(1/2)*ddqr4*cos(q4 - 2*q5))/64 - (9*3^(1/2)*ddqr4*cos(q4 + 2*q5))/64 + (3^(1/2)*ddqr5*cos(q4 - q5))/16 - (3^(1/2)*ddqr1*cos(q3 - q2 + q4))/64 - (3*3^(1/2)*ddqr5*cos(q4 + q5))/16 - (3^(1/2)*ddqr4*cos(q4))/32 - (3*3^(1/2)*ddqr5*cos(q4))/8;
Y3_21_1=sin(q2 - q3);
Y3_22_1=-sin(q2 - q3);
Y3_23_1=(3^(1/2)*sin(q2 - q3 + q4))/4 - sin(q2 - q3)/2 + (3^(1/2)*sin(q3 - q2 + q4))/4;
Y3_24_1=(3*sin(q3 - q2 + q5))/8 - (3*sin(q2 - q3 + q5))/8 - sin(q2 - q3)/4 + (3^(1/2)*sin(q2 - q3 + q4 - q5))/16 - (3^(1/2)*sin(q2 - q3 - q4 + q5))/16 + (3^(1/2)*sin(q2 - q3 + q4))/8 + (3^(1/2)*sin(q3 - q2 + q4))/8 - (3*3^(1/2)*sin(q2 - q3 + q4 + q5))/16 - (3*3^(1/2)*sin(q3 - q2 + q4 + q5))/16;
Y4_4_1=(1369*ddqr4)/1000000 + (33337*ddqr1*cos(q2 - q3 + q4))/10000000 - (35927*ddqr1*cos(q3 - q2 + q4))/10000000 - (1073*ddqr1*cos(q2 + q4))/200000 + (1073*ddqr2*cos(q3 + q4))/200000 - (4329*ddqr2*cos(q4))/625000 + (4329*ddqr3*cos(q4))/625000 + (1369*ddqr1*cos(q2 - q3))/1000000 + (1073*ddqr1*cos(q2 - q4))/200000 + (1073*ddqr2*cos(q3 - q4))/200000 - (259*dq1*dqr1*sin(q4))/1000000 + (1369*dq1*dqr1*sin(2*q4))/4000000 - (1369*dq2*dqr2*sin(2*q4))/2000000 + (1369*dq2*dqr3*sin(2*q4))/2000000 + (1369*dq3*dqr2*sin(2*q4))/2000000 - (1369*dq3*dqr3*sin(2*q4))/2000000 + (1369*dq1*dqr2*cos(q2)*sin(q3))/2000000 - (1369*dq1*dqr2*cos(q3)*sin(q2))/2000000 + (1369*dq2*dqr1*cos(q2)*sin(q3))/2000000 - (1369*dq2*dqr1*cos(q3)*sin(q2))/2000000 - (1073*dq1*dqr1*cos(q4)*sin(q3))/200000 + (1073*dq1*dqr2*cos(q2)*sin(q4))/100000 - (1369*dq1*dqr3*cos(q2)*sin(q3))/2000000 + (1369*dq1*dqr3*cos(q3)*sin(q2))/2000000 + (1073*dq2*dqr1*cos(q2)*sin(q4))/100000 - (1369*dq3*dqr1*cos(q2)*sin(q3))/2000000 + (1369*dq3*dqr1*cos(q3)*sin(q2))/2000000 - (1073*dq2*dqr2*cos(q4)*sin(q3))/100000 + (1073*dq1*dqr1*cos(2*q2)*cos(q4)*sin(q3))/200000 - (1073*dq1*dqr1*sin(2*q2)*cos(q3)*cos(q4))/200000 - (1369*dq1*dqr2*cos(2*q4)*cos(q2)*sin(q3))/2000000 + (1369*dq1*dqr2*cos(2*q4)*cos(q3)*sin(q2))/2000000 - (1369*dq2*dqr1*cos(2*q4)*cos(q2)*sin(q3))/2000000 + (1369*dq2*dqr1*cos(2*q4)*cos(q3)*sin(q2))/2000000 + (1369*dq1*dqr3*cos(2*q4)*cos(q2)*sin(q3))/2000000 - (1369*dq1*dqr3*cos(2*q4)*cos(q3)*sin(q2))/2000000 + (1369*dq3*dqr1*cos(2*q4)*cos(q2)*sin(q3))/2000000 - (1369*dq3*dqr1*cos(2*q4)*cos(q3)*sin(q2))/2000000 - (4329*dq1*dqr1*cos(2*q2)*sin(2*q3)*cos(q4))/1250000 + (4329*dq1*dqr1*cos(2*q3)*sin(2*q2)*cos(q4))/1250000 - (4329*dq1*dqr2*cos(q2)*cos(q3)*sin(q4))/625000 - (4329*dq2*dqr1*cos(q2)*cos(q3)*sin(q4))/625000 + (4329*dq1*dqr3*cos(q2)*cos(q3)*sin(q4))/625000 + (4329*dq3*dqr1*cos(q2)*cos(q3)*sin(q4))/625000 - (1369*dq1*dqr1*cos(2*q2)*cos(2*q3)*sin(2*q4))/4000000 - (4329*dq1*dqr2*sin(q2)*sin(q3)*sin(q4))/625000 - (4329*dq2*dqr1*sin(q2)*sin(q3)*sin(q4))/625000 + (4329*dq1*dqr3*sin(q2)*sin(q3)*sin(q4))/625000 + (4329*dq3*dqr1*sin(q2)*sin(q3)*sin(q4))/625000 - (1369*dq1*dqr1*sin(2*q2)*sin(2*q3)*sin(2*q4))/4000000;
Y4_5_1=(259*dq1*dqr1*cos(q4)*sin(q5))/1000000 - dq1*dqr1*sin(q4)*((4487*3^(1/2))/20000000 + 259/1000000) + (259*dq1*dqr1*cos(q5)*sin(q4))/2000000 - (4107*dq2*dqr1*cos(2*q5)*cos(q2)*sin(q3))/16000000 + (4107*dq2*dqr1*cos(2*q5)*cos(q3)*sin(q2))/16000000 + (4107*dq3*dqr1*cos(2*q5)*cos(q2)*sin(q3))/16000000 - (4107*dq3*dqr1*cos(2*q5)*cos(q3)*sin(q2))/16000000 + (4107*dq5*dqr1*sin(2*q5)*cos(q2)*cos(q3))/8000000 + dq2*dqr1*cos(q2)*sin(q3)*((23717*3^(1/2))/20000000 + 2122493/800000000) - dq2*dqr1*cos(q3)*sin(q2)*((23717*3^(1/2))/20000000 + 2122493/800000000) - dq3*dqr1*cos(q2)*sin(q3)*((23717*3^(1/2))/20000000 + 2122493/800000000) + dq3*dqr1*cos(q3)*sin(q2)*((23717*3^(1/2))/20000000 + 2122493/800000000) + (4107*dq5*dqr1*sin(2*q5)*sin(q2)*sin(q3))/8000000 - dq1*dqr1*cos(2*q4)*sin(q5)*((23717*3^(1/2))/40000000 + 1369/2000000) - dq1*dqr1*sin(2*q4)*cos(q5)*((23717*3^(1/2))/80000000 + 1369/4000000) + (1073*dq1*dqr1*cos(q4)*cos(q5)*sin(q3))/400000 - (1073*dq2*dqr1*cos(q2)*cos(q4)*sin(q5))/100000 - (1073*dq2*dqr1*cos(q2)*cos(q5)*sin(q4))/200000 - (1073*dq1*dqr1*sin(q3)*sin(q4)*sin(q5))/200000 + dq2*dqr1*cos(q2)*sin(q4)*((18589*3^(1/2))/2000000 + 1073/100000) - dq1*dqr1*cos(q4)*sin(q3)*((18589*3^(1/2))/4000000 + 1073/200000) - (1369*dq1*dqr1*cos(2*q2)*cos(2*q3)*cos(2*q5)*sin(2*q4))/6400000 + (1073*dq1*dqr1*cos(2*q2)*sin(q3)*sin(q4)*sin(q5))/200000 - (1073*dq1*dqr1*sin(2*q2)*cos(q3)*sin(q4)*sin(q5))/200000 + (1369*3^(1/2)*dq5*dqr1*cos(q2)*cos(q4)*sin(q3))/4000000 - (1369*3^(1/2)*dq5*dqr1*cos(q3)*cos(q4)*sin(q2))/4000000 - (1369*dq1*dqr1*cos(2*q4)*sin(2*q2)*sin(2*q3)*sin(2*q5))/8000000 - (1369*dq1*dqr1*cos(2*q5)*sin(2*q2)*sin(2*q3)*sin(2*q4))/6400000 + dq1*dqr1*cos(2*q2)*cos(q4)*sin(q3)*((18589*3^(1/2))/4000000 + 1073/200000) - dq1*dqr1*sin(2*q2)*cos(q3)*cos(q4)*((18589*3^(1/2))/4000000 + 1073/200000) - (1369*dq2*dqr1*cos(2*q4)*cos(2*q5)*cos(q2)*sin(q3))/3200000 + (1369*dq2*dqr1*cos(2*q4)*cos(2*q5)*cos(q3)*sin(q2))/3200000 + (1369*dq3*dqr1*cos(2*q4)*cos(2*q5)*cos(q2)*sin(q3))/3200000 - (1369*dq3*dqr1*cos(2*q4)*cos(2*q5)*cos(q3)*sin(q2))/3200000 - dq1*dqr1*cos(2*q2)*cos(2*q3)*sin(2*q4)*((23717*3^(1/2))/40000000 + 1574893/1600000000) - dq2*dqr1*cos(2*q4)*cos(q2)*sin(q3)*((23717*3^(1/2))/20000000 + 1574893/800000000) + dq2*dqr1*cos(2*q4)*cos(q3)*sin(q2)*((23717*3^(1/2))/20000000 + 1574893/800000000) + dq3*dqr1*cos(2*q4)*cos(q2)*sin(q3)*((23717*3^(1/2))/20000000 + 1574893/800000000) - dq3*dqr1*cos(2*q4)*cos(q3)*sin(q2)*((23717*3^(1/2))/20000000 + 1574893/800000000) - (32449*dq1*dqr1*cos(2*q2)*sin(2*q3)*sin(q4)*sin(q5))/8000000 + (32449*dq1*dqr1*cos(2*q3)*sin(2*q2)*sin(q4)*sin(q5))/8000000 + (1369*dq2*dqr1*sin(2*q4)*sin(2*q5)*cos(q2)*sin(q3))/4000000 - (1369*dq2*dqr1*sin(2*q4)*sin(2*q5)*cos(q3)*sin(q2))/4000000 - (1369*dq3*dqr1*sin(2*q4)*sin(2*q5)*cos(q2)*sin(q3))/4000000 + (1369*dq3*dqr1*sin(2*q4)*sin(2*q5)*cos(q3)*sin(q2))/4000000 - dq1*dqr1*sin(2*q2)*sin(2*q3)*sin(2*q4)*((23717*3^(1/2))/40000000 + 1574893/1600000000) + (32449*dq2*dqr1*cos(q2)*cos(q3)*cos(q4)*sin(q5))/4000000 - (32449*dq3*dqr1*cos(q2)*cos(q3)*cos(q4)*sin(q5))/4000000 - dq1*dqr1*cos(2*q2)*sin(2*q3)*cos(q4)*((548467*3^(1/2))/160000000 + 32449/8000000) + dq1*dqr1*cos(2*q3)*sin(2*q2)*cos(q4)*((548467*3^(1/2))/160000000 + 32449/8000000) + (32449*dq2*dqr1*cos(q4)*sin(q2)*sin(q3)*sin(q5))/4000000 - (32449*dq3*dqr1*cos(q4)*sin(q2)*sin(q3)*sin(q5))/4000000 - dq2*dqr1*cos(q2)*cos(q5)*sin(q3)*((23717*3^(1/2))/40000000 + 1369/2000000) + dq2*dqr1*cos(q3)*cos(q5)*sin(q2)*((23717*3^(1/2))/40000000 + 1369/2000000) + dq3*dqr1*cos(q2)*cos(q5)*sin(q3)*((23717*3^(1/2))/40000000 + 1369/2000000) - dq3*dqr1*cos(q3)*cos(q5)*sin(q2)*((23717*3^(1/2))/40000000 + 1369/2000000) + dq5*dqr1*cos(q2)*cos(q3)*sin(q5)*((23717*3^(1/2))/40000000 + 1369/2000000) - dq2*dqr1*cos(q2)*cos(q3)*sin(q4)*((548467*3^(1/2))/80000000 + 32449/4000000) + dq3*dqr1*cos(q2)*cos(q3)*sin(q4)*((548467*3^(1/2))/80000000 + 32449/4000000) - (1073*dq1*dqr1*cos(2*q2)*cos(q4)*cos(q5)*sin(q3))/400000 + (1073*dq1*dqr1*sin(2*q2)*cos(q3)*cos(q4)*cos(q5))/400000 + dq5*dqr1*sin(q2)*sin(q3)*sin(q5)*((23717*3^(1/2))/40000000 + 1369/2000000) - dq2*dqr1*sin(q2)*sin(q3)*sin(q4)*((548467*3^(1/2))/80000000 + 32449/4000000) + dq3*dqr1*sin(q2)*sin(q3)*sin(q4)*((548467*3^(1/2))/80000000 + 32449/4000000) + (1369*3^(1/2)*dq1*dqr1*cos(2*q2)*cos(2*q5)*sin(2*q3)*cos(q4))/16000000 - (1369*3^(1/2)*dq1*dqr1*cos(2*q3)*cos(2*q5)*sin(2*q2)*cos(q4))/16000000 + dq2*dqr1*cos(2*q4)*cos(q2)*cos(q5)*sin(q3)*((23717*3^(1/2))/40000000 + 1369/2000000) - dq2*dqr1*cos(2*q4)*cos(q3)*cos(q5)*sin(q2)*((23717*3^(1/2))/40000000 + 1369/2000000) - dq3*dqr1*cos(2*q4)*cos(q2)*cos(q5)*sin(q3)*((23717*3^(1/2))/40000000 + 1369/2000000) + dq3*dqr1*cos(2*q4)*cos(q3)*cos(q5)*sin(q2)*((23717*3^(1/2))/40000000 + 1369/2000000) - (1369*3^(1/2)*dq1*dqr1*cos(2*q2)*sin(2*q3)*sin(2*q5)*sin(q4))/8000000 + (1369*3^(1/2)*dq1*dqr1*cos(2*q3)*sin(2*q2)*sin(2*q5)*sin(q4))/8000000 - dq2*dqr1*sin(2*q4)*cos(q2)*sin(q3)*sin(q5)*((23717*3^(1/2))/20000000 + 1369/1000000) + dq2*dqr1*sin(2*q4)*cos(q3)*sin(q2)*sin(q5)*((23717*3^(1/2))/20000000 + 1369/1000000) + dq3*dqr1*sin(2*q4)*cos(q2)*sin(q3)*sin(q5)*((23717*3^(1/2))/20000000 + 1369/1000000) - dq3*dqr1*sin(2*q4)*cos(q3)*sin(q2)*sin(q5)*((23717*3^(1/2))/20000000 + 1369/1000000) + (1369*3^(1/2)*dq2*dqr1*cos(2*q5)*cos(q2)*cos(q3)*sin(q4))/8000000 + (1369*3^(1/2)*dq2*dqr1*sin(2*q5)*cos(q2)*cos(q3)*cos(q4))/4000000 - (1369*3^(1/2)*dq3*dqr1*cos(2*q5)*cos(q2)*cos(q3)*sin(q4))/8000000 - (1369*3^(1/2)*dq3*dqr1*sin(2*q5)*cos(q2)*cos(q3)*cos(q4))/4000000 - (1369*3^(1/2)*dq5*dqr1*cos(2*q5)*cos(q2)*cos(q4)*sin(q3))/4000000 + (1369*3^(1/2)*dq5*dqr1*cos(2*q5)*cos(q3)*cos(q4)*sin(q2))/4000000 + (1369*3^(1/2)*dq2*dqr1*cos(2*q5)*sin(q2)*sin(q3)*sin(q4))/8000000 + (1369*3^(1/2)*dq2*dqr1*sin(2*q5)*cos(q4)*sin(q2)*sin(q3))/4000000 - (1369*3^(1/2)*dq3*dqr1*cos(2*q5)*sin(q2)*sin(q3)*sin(q4))/8000000 - (1369*3^(1/2)*dq3*dqr1*sin(2*q5)*cos(q4)*sin(q2)*sin(q3))/4000000 + (1369*3^(1/2)*dq5*dqr1*sin(2*q5)*cos(q2)*sin(q3)*sin(q4))/8000000 - (1369*3^(1/2)*dq5*dqr1*sin(2*q5)*cos(q3)*sin(q2)*sin(q4))/8000000 - dq1*dqr1*cos(2*q2)*sin(2*q3)*cos(q4)*cos(q5)*((1369*3^(1/2))/4000000 - 45547/40000000) + dq1*dqr1*cos(2*q3)*sin(2*q2)*cos(q4)*cos(q5)*((1369*3^(1/2))/4000000 - 45547/40000000) - dq2*dqr1*cos(q2)*cos(q3)*cos(q5)*sin(q4)*((1369*3^(1/2))/2000000 - 45547/20000000) + dq3*dqr1*cos(q2)*cos(q3)*cos(q5)*sin(q4)*((1369*3^(1/2))/2000000 - 45547/20000000) + dq1*dqr1*cos(2*q2)*cos(2*q3)*cos(2*q4)*sin(q5)*((23717*3^(1/2))/40000000 + 1369/2000000) - dq2*dqr1*cos(q5)*sin(q2)*sin(q3)*sin(q4)*((1369*3^(1/2))/2000000 - 45547/20000000) + dq3*dqr1*cos(q5)*sin(q2)*sin(q3)*sin(q4)*((1369*3^(1/2))/2000000 - 45547/20000000) - dq5*dqr1*cos(q2)*sin(q3)*sin(q4)*sin(q5)*((1369*3^(1/2))/2000000 + 71151/40000000) + dq5*dqr1*cos(q3)*sin(q2)*sin(q4)*sin(q5)*((1369*3^(1/2))/2000000 + 71151/40000000) + dq1*dqr1*cos(2*q2)*cos(2*q3)*sin(2*q4)*cos(q5)*((23717*3^(1/2))/80000000 + 1369/4000000) + dq1*dqr1*cos(2*q4)*sin(2*q2)*sin(2*q3)*sin(q5)*((23717*3^(1/2))/40000000 + 1369/2000000) + dq1*dqr1*sin(2*q2)*sin(2*q3)*sin(2*q4)*cos(q5)*((23717*3^(1/2))/80000000 + 1369/4000000);
Y4_5_2=(4107*dq5*dqr4*sin(2*q5))/8000000 + dq5*dqr4*sin(q5)*((23717*3^(1/2))/40000000 + 1369/2000000) + (1369*3^(1/2)*dq5*dqr2*sin(q4))/4000000 - (1369*3^(1/2)*dq5*dqr3*sin(q4))/4000000 + (1369*dq1*dqr1*cos(2*q4)*sin(2*q5))/8000000 + (1369*dq1*dqr1*cos(2*q5)*sin(2*q4))/6400000 - (1369*dq2*dqr2*cos(2*q4)*sin(2*q5))/4000000 - (1369*dq2*dqr2*cos(2*q5)*sin(2*q4))/3200000 + (1369*dq2*dqr3*cos(2*q4)*sin(2*q5))/4000000 + (1369*dq2*dqr3*cos(2*q5)*sin(2*q4))/3200000 + (1369*dq3*dqr2*cos(2*q4)*sin(2*q5))/4000000 + (1369*dq3*dqr2*cos(2*q5)*sin(2*q4))/3200000 - (1369*dq3*dqr3*cos(2*q4)*sin(2*q5))/4000000 - (1369*dq3*dqr3*cos(2*q5)*sin(2*q4))/3200000 - dq2*dqr2*sin(2*q4)*((23717*3^(1/2))/20000000 + 1574893/800000000) + dq2*dqr3*sin(2*q4)*((23717*3^(1/2))/20000000 + 1574893/800000000) + dq3*dqr2*sin(2*q4)*((23717*3^(1/2))/20000000 + 1574893/800000000) - dq3*dqr3*sin(2*q4)*((23717*3^(1/2))/20000000 + 1574893/800000000) + dq1*dqr1*sin(2*q4)*((23717*3^(1/2))/40000000 + 1574893/1600000000) + dq5*dqr2*cos(q4)*sin(q5)*((1369*3^(1/2))/2000000 + 71151/40000000) - dq5*dqr3*cos(q4)*sin(q5)*((1369*3^(1/2))/2000000 + 71151/40000000) - (4107*dq1*dqr2*cos(2*q5)*cos(q2)*sin(q3))/16000000 + (4107*dq1*dqr2*cos(2*q5)*cos(q3)*sin(q2))/16000000 + (4107*dq1*dqr3*cos(2*q5)*cos(q2)*sin(q3))/16000000 - (4107*dq1*dqr3*cos(2*q5)*cos(q3)*sin(q2))/16000000 + dq1*dqr2*cos(q2)*sin(q3)*((23717*3^(1/2))/20000000 + 2122493/800000000) - dq1*dqr2*cos(q3)*sin(q2)*((23717*3^(1/2))/20000000 + 2122493/800000000) - dq1*dqr3*cos(q2)*sin(q3)*((23717*3^(1/2))/20000000 + 2122493/800000000) + dq1*dqr3*cos(q3)*sin(q2)*((23717*3^(1/2))/20000000 + 2122493/800000000) + (4107*dq1*dqr5*sin(2*q5)*sin(q2)*sin(q3))/8000000 + dq2*dqr2*cos(2*q4)*sin(q5)*((23717*3^(1/2))/20000000 + 1369/1000000) - dq2*dqr3*cos(2*q4)*sin(q5)*((23717*3^(1/2))/20000000 + 1369/1000000) - dq3*dqr2*cos(2*q4)*sin(q5)*((23717*3^(1/2))/20000000 + 1369/1000000) + dq3*dqr3*cos(2*q4)*sin(q5)*((23717*3^(1/2))/20000000 + 1369/1000000) + dq2*dqr2*sin(2*q4)*cos(q5)*((23717*3^(1/2))/40000000 + 1369/2000000) - dq2*dqr3*sin(2*q4)*cos(q5)*((23717*3^(1/2))/40000000 + 1369/2000000) - dq3*dqr2*sin(2*q4)*cos(q5)*((23717*3^(1/2))/40000000 + 1369/2000000) + dq3*dqr3*sin(2*q4)*cos(q5)*((23717*3^(1/2))/40000000 + 1369/2000000) - (1369*3^(1/2)*dq5*dqr2*cos(2*q5)*sin(q4))/4000000 - (1369*3^(1/2)*dq5*dqr2*sin(2*q5)*cos(q4))/8000000 + (1369*3^(1/2)*dq5*dqr3*cos(2*q5)*sin(q4))/4000000 + (1369*3^(1/2)*dq5*dqr3*sin(2*q5)*cos(q4))/8000000 - (1073*dq1*dqr2*cos(q2)*cos(q4)*sin(q5))/100000 - (1073*dq1*dqr2*cos(q2)*cos(q5)*sin(q4))/200000 + (1073*dq2*dqr2*cos(q4)*cos(q5)*sin(q3))/200000 - (1073*dq2*dqr2*sin(q3)*sin(q4)*sin(q5))/100000 + dq1*dqr2*cos(q2)*sin(q4)*((18589*3^(1/2))/2000000 + 1073/100000) - dq2*dqr2*cos(q4)*sin(q3)*((18589*3^(1/2))/2000000 + 1073/100000) - (1369*dq1*dqr1*cos(2*q2)*cos(2*q3)*cos(2*q4)*sin(2*q5))/8000000 - (1369*3^(1/2)*dq1*dqr5*cos(q3)*cos(q4)*sin(q2))/4000000 - (1369*dq1*dqr2*cos(2*q4)*cos(2*q5)*cos(q2)*sin(q3))/3200000 + (1369*dq1*dqr2*cos(2*q4)*cos(2*q5)*cos(q3)*sin(q2))/3200000 + (1369*dq1*dqr3*cos(2*q4)*cos(2*q5)*cos(q2)*sin(q3))/3200000 - (1369*dq1*dqr3*cos(2*q4)*cos(2*q5)*cos(q3)*sin(q2))/3200000 - dq1*dqr2*cos(2*q4)*cos(q2)*sin(q3)*((23717*3^(1/2))/20000000 + 1574893/800000000) + dq1*dqr2*cos(2*q4)*cos(q3)*sin(q2)*((23717*3^(1/2))/20000000 + 1574893/800000000) + dq1*dqr3*cos(2*q4)*cos(q2)*sin(q3)*((23717*3^(1/2))/20000000 + 1574893/800000000) - dq1*dqr3*cos(2*q4)*cos(q3)*sin(q2)*((23717*3^(1/2))/20000000 + 1574893/800000000) + (1369*dq1*dqr2*sin(2*q4)*sin(2*q5)*cos(q2)*sin(q3))/4000000 - (1369*dq1*dqr2*sin(2*q4)*sin(2*q5)*cos(q3)*sin(q2))/4000000 - (1369*dq1*dqr3*sin(2*q4)*sin(2*q5)*cos(q2)*sin(q3))/4000000 + (1369*dq1*dqr3*sin(2*q4)*sin(2*q5)*cos(q3)*sin(q2))/4000000 + (32449*dq1*dqr2*cos(q2)*cos(q3)*cos(q4)*sin(q5))/4000000 - (32449*dq1*dqr3*cos(q2)*cos(q3)*cos(q4)*sin(q5))/4000000 + (32449*dq1*dqr2*cos(q4)*sin(q2)*sin(q3)*sin(q5))/4000000 - (32449*dq1*dqr3*cos(q4)*sin(q2)*sin(q3)*sin(q5))/4000000 - dq1*dqr2*cos(q2)*cos(q5)*sin(q3)*((23717*3^(1/2))/40000000 + 1369/2000000) + dq1*dqr2*cos(q3)*cos(q5)*sin(q2)*((23717*3^(1/2))/40000000 + 1369/2000000) + dq1*dqr3*cos(q2)*cos(q5)*sin(q3)*((23717*3^(1/2))/40000000 + 1369/2000000) - dq1*dqr3*cos(q3)*cos(q5)*sin(q2)*((23717*3^(1/2))/40000000 + 1369/2000000) - dq1*dqr2*cos(q2)*cos(q3)*sin(q4)*((548467*3^(1/2))/80000000 + 32449/4000000) + dq1*dqr3*cos(q2)*cos(q3)*sin(q4)*((548467*3^(1/2))/80000000 + 32449/4000000) + dq1*dqr5*sin(q2)*sin(q3)*sin(q5)*((23717*3^(1/2))/40000000 + 1369/2000000) - dq1*dqr2*sin(q2)*sin(q3)*sin(q4)*((548467*3^(1/2))/80000000 + 32449/4000000) + dq1*dqr3*sin(q2)*sin(q3)*sin(q4)*((548467*3^(1/2))/80000000 + 32449/4000000) + dq1*dqr2*cos(2*q4)*cos(q2)*cos(q5)*sin(q3)*((23717*3^(1/2))/40000000 + 1369/2000000) - dq1*dqr2*cos(2*q4)*cos(q3)*cos(q5)*sin(q2)*((23717*3^(1/2))/40000000 + 1369/2000000) - dq1*dqr3*cos(2*q4)*cos(q2)*cos(q5)*sin(q3)*((23717*3^(1/2))/40000000 + 1369/2000000) + dq1*dqr3*cos(2*q4)*cos(q3)*cos(q5)*sin(q2)*((23717*3^(1/2))/40000000 + 1369/2000000) - dq1*dqr2*sin(2*q4)*cos(q2)*sin(q3)*sin(q5)*((23717*3^(1/2))/20000000 + 1369/1000000) + dq1*dqr2*sin(2*q4)*cos(q3)*sin(q2)*sin(q5)*((23717*3^(1/2))/20000000 + 1369/1000000) + dq1*dqr3*sin(2*q4)*cos(q2)*sin(q3)*sin(q5)*((23717*3^(1/2))/20000000 + 1369/1000000) - dq1*dqr3*sin(2*q4)*cos(q3)*sin(q2)*sin(q5)*((23717*3^(1/2))/20000000 + 1369/1000000) + (1369*3^(1/2)*dq1*dqr2*cos(2*q5)*cos(q2)*cos(q3)*sin(q4))/8000000 + (1369*3^(1/2)*dq1*dqr2*sin(2*q5)*cos(q2)*cos(q3)*cos(q4))/4000000 - (1369*3^(1/2)*dq1*dqr3*cos(2*q5)*cos(q2)*cos(q3)*sin(q4))/8000000 - (1369*3^(1/2)*dq1*dqr3*sin(2*q5)*cos(q2)*cos(q3)*cos(q4))/4000000 + (1369*3^(1/2)*dq1*dqr5*cos(2*q5)*cos(q3)*cos(q4)*sin(q2))/4000000 + (1369*3^(1/2)*dq1*dqr2*cos(2*q5)*sin(q2)*sin(q3)*sin(q4))/8000000 + (1369*3^(1/2)*dq1*dqr2*sin(2*q5)*cos(q4)*sin(q2)*sin(q3))/4000000 - (1369*3^(1/2)*dq1*dqr3*cos(2*q5)*sin(q2)*sin(q3)*sin(q4))/8000000 - (1369*3^(1/2)*dq1*dqr3*sin(2*q5)*cos(q4)*sin(q2)*sin(q3))/4000000 + (1369*3^(1/2)*dq1*dqr5*sin(2*q5)*cos(q2)*sin(q3)*sin(q4))/8000000 - (1369*3^(1/2)*dq1*dqr5*sin(2*q5)*cos(q3)*sin(q2)*sin(q4))/8000000 - dq1*dqr2*cos(q2)*cos(q3)*cos(q5)*sin(q4)*((1369*3^(1/2))/2000000 - 45547/20000000) + dq1*dqr3*cos(q2)*cos(q3)*cos(q5)*sin(q4)*((1369*3^(1/2))/2000000 - 45547/20000000) - dq1*dqr2*cos(q5)*sin(q2)*sin(q3)*sin(q4)*((1369*3^(1/2))/2000000 - 45547/20000000) + dq1*dqr3*cos(q5)*sin(q2)*sin(q3)*sin(q4)*((1369*3^(1/2))/2000000 - 45547/20000000) - dq1*dqr5*cos(q2)*sin(q3)*sin(q4)*sin(q5)*((1369*3^(1/2))/2000000 + 71151/40000000) + dq1*dqr5*cos(q3)*sin(q2)*sin(q4)*sin(q5)*((1369*3^(1/2))/2000000 + 71151/40000000);
Y4_5_3=(1369*ddqr5)/2000000 - (1073*ddqr1*cos(q2 + q4 - q5))/800000 + (1073*ddqr1*cos(q2 - q4 + q5))/800000 - (3219*ddqr1*cos(q4 - q2 + q5))/800000 + (1073*ddqr2*cos(q3 + q4 - q5))/800000 + (1073*ddqr2*cos(q3 - q4 + q5))/800000 - (3219*ddqr2*cos(q4 - q3 + q5))/800000 - (4107*ddqr1*cos(q2 - q3 + 2*q5))/16000000 - (4107*ddqr1*cos(q3 - q2 + 2*q5))/16000000 + (3219*ddqr1*cos(q2 + q4 + q5))/800000 - (3219*ddqr2*cos(q3 + q4 + q5))/800000 - (4107*ddqr4*cos(2*q5))/8000000 + ddqr4*((23717*3^(1/2))/10000000 + 2122493/400000000) - (1369*3^(1/2)*ddqr2*cos(q4 - 2*q5))/16000000 + (4107*3^(1/2)*ddqr2*cos(q4 + 2*q5))/16000000 + (1369*3^(1/2)*ddqr3*cos(q4 - 2*q5))/16000000 - (4107*3^(1/2)*ddqr3*cos(q4 + 2*q5))/16000000 - ddqr1*cos(q2 - q3 - q4 + q5)*((1369*3^(1/2))/8000000 + 14911/10000000) + ddqr1*cos(q2 - q3 + q4 - q5)*((1369*3^(1/2))/8000000 + 28527/20000000) - ddqr1*cos(q3 - q2 + q4)*((113283*3^(1/2))/32000000 + 6697/1600000) - ddqr1*cos(q2 - q3 + q5)*((23717*3^(1/2))/40000000 + 1369/2000000) - ddqr1*cos(q3 - q2 + q5)*((23717*3^(1/2))/40000000 + 1369/2000000) + ddqr1*cos(q2 - q3 + q4)*((530519*3^(1/2))/160000000 + 31413/8000000) + (1369*3^(1/2)*ddqr1*cos(q2 - q3 + q4 - 2*q5))/32000000 - (4107*3^(1/2)*ddqr1*cos(q2 - q3 + q4 + 2*q5))/32000000 + (4107*3^(1/2)*ddqr1*cos(q3 - q2 + q4 + 2*q5))/32000000 + (4107*dq4*dqr5*sin(2*q5))/8000000 - ddqr1*cos(q2 + q4)*((18589*3^(1/2))/4000000 + 1073/200000) + ddqr2*cos(q3 + q4)*((18589*3^(1/2))/4000000 + 1073/200000) - ddqr2*cos(q4 + q5)*((1369*3^(1/2))/4000000 - 12987/2500000) + ddqr3*cos(q4 + q5)*((1369*3^(1/2))/4000000 - 12987/2500000) - ddqr4*cos(q5)*((23717*3^(1/2))/20000000 + 1369/1000000) - ddqr5*cos(q5)*((23717*3^(1/2))/20000000 + 1369/1000000) - ddqr2*cos(q4)*((548467*3^(1/2))/80000000 + 32449/4000000) + ddqr3*cos(q4)*((548467*3^(1/2))/80000000 + 32449/4000000) - (1369*3^(1/2)*ddqr1*cos(q2 - q3 - q4 + 2*q5))/32000000 + ddqr1*cos(q2 - q3 + q4 + q5)*((1369*3^(1/2))/8000000 - 100011/40000000) - ddqr1*cos(q3 - q2 + q4 + q5)*((1369*3^(1/2))/8000000 - 107781/40000000) + ddqr1*cos(q2 - q4)*((18589*3^(1/2))/4000000 + 1073/200000) + ddqr2*cos(q3 - q4)*((18589*3^(1/2))/4000000 + 1073/200000) - ddqr2*cos(q4 - q5)*((1369*3^(1/2))/4000000 + 58349/20000000) + ddqr3*cos(q4 - q5)*((1369*3^(1/2))/4000000 + 58349/20000000) + ddqr1*cos(q2 - q3)*((23717*3^(1/2))/10000000 + 2122493/400000000) + dq5*dqr5*sin(q5)*((23717*3^(1/2))/20000000 + 1369/1000000) + dq4*dqr5*sin(q5)*((23717*3^(1/2))/40000000 + 1369/2000000) + (1369*3^(1/2)*dq2*dqr5*sin(q4))/4000000 - (1369*3^(1/2)*dq3*dqr5*sin(q4))/4000000 + dq2*dqr5*cos(q4)*sin(q5)*((1369*3^(1/2))/2000000 + 71151/40000000) - dq3*dqr5*cos(q4)*sin(q5)*((1369*3^(1/2))/2000000 + 71151/40000000) + (4107*dq1*dqr5*sin(2*q5)*cos(q2)*cos(q3))/8000000 - (1369*3^(1/2)*dq2*dqr5*cos(2*q5)*sin(q4))/4000000 - (1369*3^(1/2)*dq2*dqr5*sin(2*q5)*cos(q4))/8000000 + (1369*3^(1/2)*dq3*dqr5*cos(2*q5)*sin(q4))/4000000 + (1369*3^(1/2)*dq3*dqr5*sin(2*q5)*cos(q4))/8000000 + (1369*3^(1/2)*dq1*dqr5*cos(q2)*cos(q4)*sin(q3))/4000000 + dq1*dqr5*cos(q2)*cos(q3)*sin(q5)*((23717*3^(1/2))/40000000 + 1369/2000000) - (1369*3^(1/2)*dq1*dqr5*cos(2*q5)*cos(q2)*cos(q4)*sin(q3))/4000000;
Y4_9_1=ddqr1*cos(q3 - q2 + q4)*((971*3^(1/2))/20000 + 37/4000) - (37*3^(1/2)*ddqr1*cos(q2 - q3))/1000 - (29*3^(1/2)*ddqr1*cos(q2 - q4))/400 - (29*3^(1/2)*ddqr2*cos(q3 - q4))/400 - ddqr1*cos(q2 - q3 + q4)*((901*3^(1/2))/20000 + 37/4000) - (37*3^(1/2)*ddqr4)/1000 + ddqr2*cos(q4)*((117*3^(1/2))/1250 + 37/2000) - ddqr3*cos(q4)*((117*3^(1/2))/1250 + 37/2000) + (29*3^(1/2)*ddqr1*cos(q2 + q4))/400 - (29*3^(1/2)*ddqr2*cos(q3 + q4))/400 + (7*3^(1/2)*dq1*dqr1*sin(q4))/2000 - (37*3^(1/2)*dq1*dqr1*sin(2*q4))/4000 + (37*3^(1/2)*dq2*dqr2*sin(2*q4))/2000 - (37*3^(1/2)*dq2*dqr3*sin(2*q4))/2000 - (37*3^(1/2)*dq3*dqr2*sin(2*q4))/2000 + (37*3^(1/2)*dq3*dqr3*sin(2*q4))/2000 - (37*3^(1/2)*dq1*dqr2*cos(q2)*sin(q3))/2000 + (37*3^(1/2)*dq1*dqr2*cos(q3)*sin(q2))/2000 - (37*3^(1/2)*dq2*dqr1*cos(q2)*sin(q3))/2000 + (37*3^(1/2)*dq2*dqr1*cos(q3)*sin(q2))/2000 + (29*3^(1/2)*dq1*dqr1*cos(q4)*sin(q3))/400 - (29*3^(1/2)*dq1*dqr2*cos(q2)*sin(q4))/200 + (37*3^(1/2)*dq1*dqr3*cos(q2)*sin(q3))/2000 - (37*3^(1/2)*dq1*dqr3*cos(q3)*sin(q2))/2000 - (29*3^(1/2)*dq2*dqr1*cos(q2)*sin(q4))/200 + (37*3^(1/2)*dq3*dqr1*cos(q2)*sin(q3))/2000 - (37*3^(1/2)*dq3*dqr1*cos(q3)*sin(q2))/2000 + (29*3^(1/2)*dq2*dqr2*cos(q4)*sin(q3))/200 + (37*3^(1/2)*dq1*dqr1*cos(2*q2)*cos(2*q3)*sin(2*q4))/4000 + (37*3^(1/2)*dq1*dqr1*sin(2*q2)*sin(2*q3)*sin(2*q4))/4000 - (29*3^(1/2)*dq1*dqr1*cos(2*q2)*cos(q4)*sin(q3))/400 + (29*3^(1/2)*dq1*dqr1*sin(2*q2)*cos(q3)*cos(q4))/400 + (37*3^(1/2)*dq1*dqr2*cos(2*q4)*cos(q2)*sin(q3))/2000 - (37*3^(1/2)*dq1*dqr2*cos(2*q4)*cos(q3)*sin(q2))/2000 + (37*3^(1/2)*dq2*dqr1*cos(2*q4)*cos(q2)*sin(q3))/2000 - (37*3^(1/2)*dq2*dqr1*cos(2*q4)*cos(q3)*sin(q2))/2000 - (37*3^(1/2)*dq1*dqr3*cos(2*q4)*cos(q2)*sin(q3))/2000 + (37*3^(1/2)*dq1*dqr3*cos(2*q4)*cos(q3)*sin(q2))/2000 - (37*3^(1/2)*dq3*dqr1*cos(2*q4)*cos(q2)*sin(q3))/2000 + (37*3^(1/2)*dq3*dqr1*cos(2*q4)*cos(q3)*sin(q2))/2000 + dq1*dqr1*cos(2*q2)*sin(2*q3)*cos(q4)*((117*3^(1/2))/2500 + 37/4000) - dq1*dqr1*cos(2*q3)*sin(2*q2)*cos(q4)*((117*3^(1/2))/2500 + 37/4000) + dq1*dqr2*cos(q2)*cos(q3)*sin(q4)*((117*3^(1/2))/1250 + 37/2000) + dq2*dqr1*cos(q2)*cos(q3)*sin(q4)*((117*3^(1/2))/1250 + 37/2000) - dq1*dqr3*cos(q2)*cos(q3)*sin(q4)*((117*3^(1/2))/1250 + 37/2000) - dq3*dqr1*cos(q2)*cos(q3)*sin(q4)*((117*3^(1/2))/1250 + 37/2000) + dq1*dqr2*sin(q2)*sin(q3)*sin(q4)*((117*3^(1/2))/1250 + 37/2000) + dq2*dqr1*sin(q2)*sin(q3)*sin(q4)*((117*3^(1/2))/1250 + 37/2000) - dq1*dqr3*sin(q2)*sin(q3)*sin(q4)*((117*3^(1/2))/1250 + 37/2000) - dq3*dqr1*sin(q2)*sin(q3)*sin(q4)*((117*3^(1/2))/1250 + 37/2000);
Y4_10_1=(7*3^(1/2)*dq1*dqr1*sin(q4))/4000 + (29*3^(1/2)*dq1*dqr1*cos(q4)*sin(q3))/800 - (29*3^(1/2)*dq2*dqr1*cos(q2)*sin(q4))/400 - (7*3^(1/2)*dq1*dqr1*cos(q4)*sin(q5))/2000 - (7*3^(1/2)*dq1*dqr1*cos(q5)*sin(q4))/4000 + dq1*dqr1*cos(2*q4)*sin(q5)*((111*3^(1/2))/8000 + 1923/80000) + dq1*dqr1*sin(2*q4)*cos(q5)*((111*3^(1/2))/16000 + 1923/160000) - (111*dq5*dqr1*cos(q2)*cos(q4)*sin(q3))/4000 + (111*dq5*dqr1*cos(q3)*cos(q4)*sin(q2))/4000 - dq2*dqr1*cos(q2)*sin(q3)*((333*3^(1/2))/16000 + 1923/80000) + dq2*dqr1*cos(q3)*sin(q2)*((333*3^(1/2))/16000 + 1923/80000) + dq3*dqr1*cos(q2)*sin(q3)*((333*3^(1/2))/16000 + 1923/80000) - dq3*dqr1*cos(q3)*sin(q2)*((333*3^(1/2))/16000 + 1923/80000) - (111*dq2*dqr1*cos(2*q5)*sin(q2)*sin(q3)*sin(q4))/8000 - (111*dq2*dqr1*sin(2*q5)*cos(q4)*sin(q2)*sin(q3))/4000 + (111*dq3*dqr1*cos(2*q5)*sin(q2)*sin(q3)*sin(q4))/8000 + (111*dq3*dqr1*sin(2*q5)*cos(q4)*sin(q2)*sin(q3))/4000 - (111*dq5*dqr1*sin(2*q5)*cos(q2)*sin(q3)*sin(q4))/8000 + (111*dq5*dqr1*sin(2*q5)*cos(q3)*sin(q2)*sin(q4))/8000 + dq1*dqr1*sin(2*q2)*sin(2*q3)*sin(2*q4)*((37*3^(1/2))/32000 + 1923/160000) - (29*3^(1/2)*dq1*dqr1*cos(q4)*cos(q5)*sin(q3))/800 + (29*3^(1/2)*dq2*dqr1*cos(q2)*cos(q4)*sin(q5))/200 + (29*3^(1/2)*dq2*dqr1*cos(q2)*cos(q5)*sin(q4))/400 + dq2*dqr1*cos(2*q4)*cos(q2)*sin(q3)*((37*3^(1/2))/16000 + 1923/80000) - dq2*dqr1*cos(2*q4)*cos(q3)*sin(q2)*((37*3^(1/2))/16000 + 1923/80000) - dq3*dqr1*cos(2*q4)*cos(q2)*sin(q3)*((37*3^(1/2))/16000 + 1923/80000) + dq3*dqr1*cos(2*q4)*cos(q3)*sin(q2)*((37*3^(1/2))/16000 + 1923/80000) + (29*3^(1/2)*dq1*dqr1*sin(q3)*sin(q4)*sin(q5))/400 - (29*3^(1/2)*dq1*dqr1*cos(2*q2)*cos(q4)*sin(q3))/800 + (29*3^(1/2)*dq1*dqr1*sin(2*q2)*cos(q3)*cos(q4))/800 + (111*3^(1/2)*dq2*dqr1*cos(2*q5)*cos(q2)*sin(q3))/16000 - (111*3^(1/2)*dq2*dqr1*cos(2*q5)*cos(q3)*sin(q2))/16000 - (111*3^(1/2)*dq3*dqr1*cos(2*q5)*cos(q2)*sin(q3))/16000 + (111*3^(1/2)*dq3*dqr1*cos(2*q5)*cos(q3)*sin(q2))/16000 - (111*3^(1/2)*dq5*dqr1*sin(2*q5)*cos(q2)*cos(q3))/8000 + dq1*dqr1*cos(2*q2)*sin(2*q3)*cos(q4)*((2513*3^(1/2))/80000 - 37/16000) - dq1*dqr1*cos(2*q3)*sin(2*q2)*cos(q4)*((2513*3^(1/2))/80000 - 37/16000) - (111*3^(1/2)*dq5*dqr1*sin(2*q5)*sin(q2)*sin(q3))/8000 - (111*dq1*dqr1*cos(2*q2)*cos(2*q5)*sin(2*q3)*cos(q4))/16000 + (111*dq1*dqr1*cos(2*q3)*cos(2*q5)*sin(2*q2)*cos(q4))/16000 + (111*dq1*dqr1*cos(2*q2)*sin(2*q3)*sin(2*q5)*sin(q4))/8000 - (111*dq1*dqr1*cos(2*q3)*sin(2*q2)*sin(2*q5)*sin(q4))/8000 + dq2*dqr1*cos(q2)*cos(q3)*sin(q4)*((2513*3^(1/2))/40000 - 37/8000) - dq3*dqr1*cos(q2)*cos(q3)*sin(q4)*((2513*3^(1/2))/40000 - 37/8000) + dq2*dqr1*cos(q2)*cos(q5)*sin(q3)*((111*3^(1/2))/8000 + 1923/80000) - dq2*dqr1*cos(q3)*cos(q5)*sin(q2)*((111*3^(1/2))/8000 + 1923/80000) - dq3*dqr1*cos(q2)*cos(q5)*sin(q3)*((111*3^(1/2))/8000 + 1923/80000) + dq3*dqr1*cos(q3)*cos(q5)*sin(q2)*((111*3^(1/2))/8000 + 1923/80000) - dq5*dqr1*cos(q2)*cos(q3)*sin(q5)*((111*3^(1/2))/8000 + 1923/80000) - (111*dq2*dqr1*cos(2*q5)*cos(q2)*cos(q3)*sin(q4))/8000 - (111*dq2*dqr1*sin(2*q5)*cos(q2)*cos(q3)*cos(q4))/4000 + (111*dq3*dqr1*cos(2*q5)*cos(q2)*cos(q3)*sin(q4))/8000 + (111*dq3*dqr1*sin(2*q5)*cos(q2)*cos(q3)*cos(q4))/4000 + (111*dq5*dqr1*cos(2*q5)*cos(q2)*cos(q4)*sin(q3))/4000 - (111*dq5*dqr1*cos(2*q5)*cos(q3)*cos(q4)*sin(q2))/4000 + dq1*dqr1*cos(2*q2)*cos(2*q3)*sin(2*q4)*((37*3^(1/2))/32000 + 1923/160000) + dq2*dqr1*sin(q2)*sin(q3)*sin(q4)*((2513*3^(1/2))/40000 - 37/8000) - dq3*dqr1*sin(q2)*sin(q3)*sin(q4)*((2513*3^(1/2))/40000 - 37/8000) - dq5*dqr1*sin(q2)*sin(q3)*sin(q5)*((111*3^(1/2))/8000 + 1923/80000) - dq2*dqr1*cos(2*q4)*cos(q2)*cos(q5)*sin(q3)*((111*3^(1/2))/8000 + 1923/80000) + dq2*dqr1*cos(2*q4)*cos(q3)*cos(q5)*sin(q2)*((111*3^(1/2))/8000 + 1923/80000) + dq3*dqr1*cos(2*q4)*cos(q2)*cos(q5)*sin(q3)*((111*3^(1/2))/8000 + 1923/80000) - dq3*dqr1*cos(2*q4)*cos(q3)*cos(q5)*sin(q2)*((111*3^(1/2))/8000 + 1923/80000) + dq2*dqr1*sin(2*q4)*cos(q2)*sin(q3)*sin(q5)*((111*3^(1/2))/4000 + 1923/40000) - dq2*dqr1*sin(2*q4)*cos(q3)*sin(q2)*sin(q5)*((111*3^(1/2))/4000 + 1923/40000) - dq3*dqr1*sin(2*q4)*cos(q2)*sin(q3)*sin(q5)*((111*3^(1/2))/4000 + 1923/40000) + dq3*dqr1*sin(2*q4)*cos(q3)*sin(q2)*sin(q5)*((111*3^(1/2))/4000 + 1923/40000) + (29*3^(1/2)*dq1*dqr1*cos(2*q2)*cos(q4)*cos(q5)*sin(q3))/800 - (29*3^(1/2)*dq1*dqr1*sin(2*q2)*cos(q3)*cos(q4)*cos(q5))/800 + (37*3^(1/2)*dq1*dqr1*cos(2*q2)*cos(2*q3)*cos(2*q5)*sin(2*q4))/6400 - dq1*dqr1*cos(2*q2)*sin(2*q3)*cos(q4)*cos(q5)*((1231*3^(1/2))/80000 - 37/2000) + dq1*dqr1*cos(2*q3)*sin(2*q2)*cos(q4)*cos(q5)*((1231*3^(1/2))/80000 - 37/2000) - (29*3^(1/2)*dq1*dqr1*cos(2*q2)*sin(q3)*sin(q4)*sin(q5))/400 + (29*3^(1/2)*dq1*dqr1*sin(2*q2)*cos(q3)*sin(q4)*sin(q5))/400 + (37*3^(1/2)*dq1*dqr1*cos(2*q4)*sin(2*q2)*sin(2*q3)*sin(2*q5))/8000 + (37*3^(1/2)*dq1*dqr1*cos(2*q5)*sin(2*q2)*sin(2*q3)*sin(2*q4))/6400 + dq1*dqr1*cos(2*q2)*sin(2*q3)*sin(q4)*sin(q5)*((877*3^(1/2))/16000 + 37/8000) - dq1*dqr1*cos(2*q3)*sin(2*q2)*sin(q4)*sin(q5)*((877*3^(1/2))/16000 + 37/8000) + (37*3^(1/2)*dq2*dqr1*cos(2*q4)*cos(2*q5)*cos(q2)*sin(q3))/3200 - (37*3^(1/2)*dq2*dqr1*cos(2*q4)*cos(2*q5)*cos(q3)*sin(q2))/3200 - (37*3^(1/2)*dq3*dqr1*cos(2*q4)*cos(2*q5)*cos(q2)*sin(q3))/3200 + (37*3^(1/2)*dq3*dqr1*cos(2*q4)*cos(2*q5)*cos(q3)*sin(q2))/3200 - dq2*dqr1*cos(q2)*cos(q3)*cos(q4)*sin(q5)*((877*3^(1/2))/8000 + 37/4000) + dq3*dqr1*cos(q2)*cos(q3)*cos(q4)*sin(q5)*((877*3^(1/2))/8000 + 37/4000) - dq2*dqr1*cos(q2)*cos(q3)*cos(q5)*sin(q4)*((1231*3^(1/2))/40000 - 37/1000) + dq3*dqr1*cos(q2)*cos(q3)*cos(q5)*sin(q4)*((1231*3^(1/2))/40000 - 37/1000) - dq1*dqr1*cos(2*q2)*cos(2*q3)*cos(2*q4)*sin(q5)*((111*3^(1/2))/8000 + 1923/80000) - dq1*dqr1*cos(2*q2)*cos(2*q3)*sin(2*q4)*cos(q5)*((111*3^(1/2))/16000 + 1923/160000) - (37*3^(1/2)*dq2*dqr1*sin(2*q4)*sin(2*q5)*cos(q2)*sin(q3))/4000 + (37*3^(1/2)*dq2*dqr1*sin(2*q4)*sin(2*q5)*cos(q3)*sin(q2))/4000 + (37*3^(1/2)*dq3*dqr1*sin(2*q4)*sin(2*q5)*cos(q2)*sin(q3))/4000 - (37*3^(1/2)*dq3*dqr1*sin(2*q4)*sin(2*q5)*cos(q3)*sin(q2))/4000 - dq2*dqr1*cos(q4)*sin(q2)*sin(q3)*sin(q5)*((877*3^(1/2))/8000 + 37/4000) + dq3*dqr1*cos(q4)*sin(q2)*sin(q3)*sin(q5)*((877*3^(1/2))/8000 + 37/4000) - dq2*dqr1*cos(q5)*sin(q2)*sin(q3)*sin(q4)*((1231*3^(1/2))/40000 - 37/1000) + dq3*dqr1*cos(q5)*sin(q2)*sin(q3)*sin(q4)*((1231*3^(1/2))/40000 - 37/1000) + dq5*dqr1*cos(q2)*sin(q3)*sin(q4)*sin(q5)*((1923*3^(1/2))/80000 + 333/8000) - dq5*dqr1*cos(q3)*sin(q2)*sin(q4)*sin(q5)*((1923*3^(1/2))/80000 + 333/8000) - dq1*dqr1*cos(2*q4)*sin(2*q2)*sin(2*q3)*sin(q5)*((111*3^(1/2))/8000 + 1923/80000) - dq1*dqr1*sin(2*q2)*sin(2*q3)*sin(2*q4)*cos(q5)*((111*3^(1/2))/16000 + 1923/160000);
